simulink model "DFL_IMAP"  (R2018b)
settings: Solver=FixedStepDiscrete  StartTime=0.0  StopTime=10.0  FixedStep=0.01  RelTol=1e-3
(part 1 of 5)
settings Model: Creator=hejr  LastModifiedBy=hejr
settings OptimizationCC: BlockReduction=off  DefaultParameterBehavior=Inlined  DefaultUnderspecifiedDataType=single  EnhancedBackFolding=on  PassReuseOutputArgsAs=Individual arguments  ZeroExternalMemoryAtStartup=off  ZeroInternalMemoryAtStartup=off  OptimizeBlockOrder=speed  DifferentSizesBufferReuse=on  OptimizationCustomize=off
settings DebuggingCC: ParameterTunabilityLossMsg=error
settings SFSimCC: MATLABDynamicMemAlloc=off
settings RTWCC: SystemTargetFile=autosar.tlc  GenCodeOnly=on  TemplateMakefile=ert_default_tmf  Description=AUTOSAR  GenerateReport=on  IncludeHyperlinkInReport=on  LaunchReport=on  GenerateTraceInfo=on  GenerateTraceReport=on  GenerateTraceReportSl=on  GenerateTraceReportSf=on  GenerateTraceReportEml=on  GenerateCodeMetricsReport=on
settings CodeAppCC: ForceParamTrailComments=on  IgnoreCustomStorageClasses=off  OperatorAnnotations=on  SimulinkDataObjDesc=on  SFDataObjDesc=on  InsertBlockDesc=on
settings STFCustomTargetCC: TargetLangStandard=C99 (ISO)  MultiwordLength=256  ParMdlRefBuildCompliant=on  CompOptLevelCompliant=on  IncludeMdlTerminateFcn=off  CombineOutputUpdateFcns=on  SuppressErrorStatus=on  ERTCustomFileBanners=on  SupportNonFinite=off  SupportComplex=off  SupportContinuousTime=off  SupportNonInlinedSFcns=off  RemoveResetFunc=on  MATLABClassNameForMDSCustomization=Simulink.SoftwareTarget.ERTCustomization  AutosarCompliant=on  UseToolchainInfoCompliant=on  LookupTableObjectStructAxisOrder=2,1,3,4,...  LUTObjectStructOrderEvenSpacing=Size,Table,Breakpoints  SystemTargetFile=autosar.tlc
settings ERTTargetCC: TargetLangStandard=C99 (ISO)  ConcurrentExecutionCompliant=off  IncludeMdlTerminateFcn=off  SuppressErrorStatus=on  SupportNonFinite=off  SupportComplex=off  ModelStepFunctionPrototypeControlCompliant=off  CPPClassGenCompliant=off  AutosarCompliant=on  LookupTableObjectStructAxisOrder=2,1,3,4,...  LUTObjectStructOrderEvenSpacing=Size,Table,Breakpoints  GenerateASAP2=on  InlinedParameterPlacement=NonHierarchical  ERTCustomFileTemplate=example_file_process.tlc

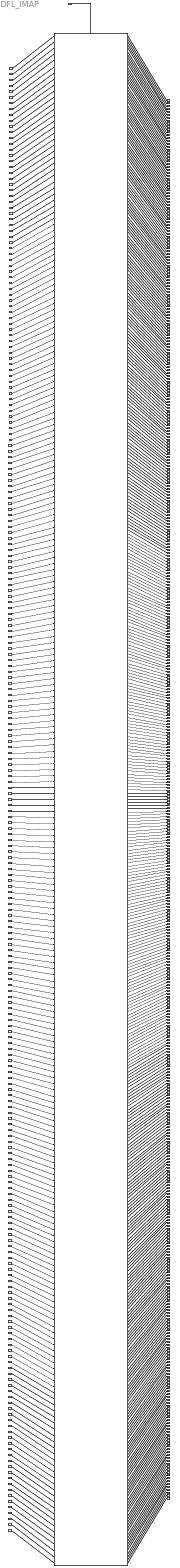
== system DFL_IMAP ==
  SWINve_y_ABS_active : Inport  OutDataTypeStr=UInt8  PortDimensions=1
  SWINve_g_ax : Inport  Port=2  OutDataTypeStr=T_M_Nm_Float32  PortDimensions=1
  SWINve_y_ESP_EnableSts : Inport  Port=3  OutDataTypeStr=UInt8  PortDimensions=1
  SWINve_y_TCS_active : Inport  Port=4  OutDataTypeStr=UInt8  PortDimensions=1
  SWINve_y_Front_Wiper_Status : Inport  Port=5  OutDataTypeStr=UInt8  PortDimensions=1
  SWINve_y_brake_pedal_status : Inport  Port=6  OutDataTypeStr=UInt8  PortDimensions=1
  SWINve_y_Engine1_IND_AccelPadel_Override : Inport  Port=7  OutDataTypeStr=UInt8  PortDimensions=1
  SWINve_y_Engine3_Status_ExtFunctionValid : Inport  Port=8  OutDataTypeStr=UInt8  PortDimensions=1
  SWINve_g_Accelerator_ActPedPos : Inport  Port=9  OutDataTypeStr=T_M_Nm_Float32  PortDimensions=1
  SWINve_g_actual_powertrain_torque : Inport  Port=10  OutDataTypeStr=T_M_Nm_Float32  PortDimensions=1
  SWINve_d_engine_revolution_speed : Inport  Port=11  OutDataTypeStr=UInt16  PortDimensions=1
  SWINve_y_Engine_Status : Inport  Port=12  OutDataTypeStr=UInt8  PortDimensions=1
  SWINve_g_maximum_powertrain_torque : Inport  Port=13  OutDataTypeStr=T_M_Nm_Float32  PortDimensions=1
  SWINve_g_minimum_powertrain_torque : Inport  Port=14  OutDataTypeStr=T_M_Nm_Float32  PortDimensions=1
  SWINve_y_VDC_active : Inport  Port=15  OutDataTypeStr=UInt8  PortDimensions=1
  SWINve_y_ABS3_FLWhlPulseCnt_Valid : Inport  Port=16  OutDataTypeStr=UInt8  PortDimensions=1
  SWINve_y_ABS3_FRWhlPulseCnt_Valid : Inport  Port=17  OutDataTypeStr=UInt8  PortDimensions=1
  SWINve_y_BCM_IgnKeyPOS : Inport  Port=18  OutDataTypeStr=UInt8  PortDimensions=1
  SWINve_y_Engine1_Status_DASReq_Resp : Inport  Port=19  OutDataTypeStr=UInt8  PortDimensions=1
  SWINve_y_Mp5_ISA_Switch : Inport  Port=20  OutDataTypeStr=UInt8  PortDimensions=1
  SWINve_y_Mp5_TSR_Switch : Inport  Port=21  OutDataTypeStr=UInt8  PortDimensions=1
  SWINve_y_BCM1_IND_HighBeamSwt_OnOff : Inport  Port=22  OutDataTypeStr=UInt8  PortDimensions=1
  SWINve_y_MP5_FCWSwitch : Inport  Port=23  OutDataTypeStr=UInt8  PortDimensions=1
  SWINve_y_MP5_FCW_Sensitivity : Inport  Port=24  OutDataTypeStr=UInt8  PortDimensions=1
  SWINve_y_Psngr_Seat_Belt_Sts : Inport  Port=25  OutDataTypeStr=UInt8  PortDimensions=1
  SWINve_y_Driver_Seat_Belt_Sts : Inport  Port=26  OutDataTypeStr=UInt8  PortDimensions=1
  SWINve_y_steering_angle_valid : Inport  Port=27  OutDataTypeStr=UInt8  PortDimensions=1
  SWINve_g_ay : Inport  Port=28  OutDataTypeStr=T_M_Nm_Float32  PortDimensions=1
  SWINve_y_Mp5_LSS_Mode : Inport  Port=29  OutDataTypeStr=UInt8  PortDimensions=1
  SWINve_y_Mp5_LSS_main_SW : Inport  Port=30  OutDataTypeStr=UInt8  PortDimensions=1
  SWINve_y_MP5_AEBSwitch : Inport  Port=31  OutDataTypeStr=UInt8  PortDimensions=1
  SWINve_g_wheel_speed_FL : Inport  Port=32  OutDataTypeStr=T_M_Nm_Float32  PortDimensions=1
  SWINve_g_wheel_speed_FR : Inport  Port=33  OutDataTypeStr=T_M_Nm_Float32  PortDimensions=1
  SWINve_g_wheel_speed_RL : Inport  Port=34  OutDataTypeStr=T_M_Nm_Float32  PortDimensions=1
  SWINve_g_wheel_speed_RR : Inport  Port=35  OutDataTypeStr=T_M_Nm_Float32  PortDimensions=1
  SWINve_g_odometer_value : Inport  Port=36  OutDataTypeStr=UInt32  PortDimensions=1
  SWINve_y_APB_Status : Inport  Port=37  OutDataTypeStr=UInt8  PortDimensions=1
  SWINve_y_ABS3_WhlPulseCnt_FL : Inport  Port=38  OutDataTypeStr=UInt8  PortDimensions=1
  SWINve_y_ABS3_WhlPulseCnt_FR : Inport  Port=39  OutDataTypeStr=UInt8  PortDimensions=1
  SWINve_y_ABS3_WhlPulseCnt_RL : Inport  Port=40  OutDataTypeStr=UInt8  PortDimensions=1
  SWINve_y_ABS3_WhlPulseCnt_RR : Inport  Port=41  OutDataTypeStr=UInt8  PortDimensions=1
  SWINve_y_ABS3_RLWhlPulseCnt_Valid : Inport  Port=42  OutDataTypeStr=UInt8  PortDimensions=1
  SWINve_y_ABS3_RRWhlPulseCnt_Valid : Inport  Port=43  OutDataTypeStr=UInt8  PortDimensions=1
  SWINve_y_VDC_Fault : Inport  Port=44  OutDataTypeStr=UInt8  PortDimensions=1
  SWINve_y_EPS1_Status_Handsoff : Inport  Port=45  OutDataTypeStr=UInt8  PortDimensions=1
  SWINve_y_EPS1_LKA_AvailSts : Inport  Port=46  OutDataTypeStr=UInt8  PortDimensions=1
  SWINve_g_steering_angle : Inport  Port=47  OutDataTypeStr=T_M_Nm_Float32  PortDimensions=1
  SWINve_g_steering_angle_spd : Inport  Port=48  OutDataTypeStr=T_M_Nm_Float32  PortDimensions=1
  SWINve_y_calibrated_status : Inport  Port=49  OutDataTypeStr=UInt8  PortDimensions=1
  SWINve_y_trimming_status : Inport  Port=50  OutDataTypeStr=UInt8  PortDimensions=1
  SWINve_y_TargetGear : Inport  Port=51  OutDataTypeStr=UInt8  PortDimensions=1
  SWINve_y_TCU2_Status_TransFailure : Inport  Port=52  OutDataTypeStr=UInt8  PortDimensions=1
  SWINve_y_ActualGear : Inport  Port=53  OutDataTypeStr=UInt8  PortDimensions=1
  SWINve_y_brake_pressure : Inport  Port=54  OutDataTypeStr=UInt8  PortDimensions=1
  SWINve_y_ESP_Status_Hold : Inport  Port=55  OutDataTypeStr=UInt8  PortDimensions=1
  SWINve_g_vehicle_speed : Inport  Port=56  OutDataTypeStr=T_M_Nm_Float32  PortDimensions=1
  SWINve_g_yrs : Inport  Port=57  OutDataTypeStr=T_M_Nm_Float32  PortDimensions=1
  System_Clock : Inport  Port=58  OutDataTypeStr=UInt16  PortDimensions=1
  SWINve_y_ABS1_RotDir_FL : Inport  Port=59  OutDataTypeStr=UInt8  PortDimensions=1
  SWINve_y_ABS1_RotDir_FR : Inport  Port=60  OutDataTypeStr=UInt8  PortDimensions=1
  SWINve_y_TCS_Fault : Inport  Port=61  OutDataTypeStr=UInt8  PortDimensions=1
  SWINve_y_ABS1_RotDir_RL : Inport  Port=62  OutDataTypeStr=UInt8  PortDimensions=1
  SWINve_y_ABS1_RotDir_RR : Inport  Port=63  OutDataTypeStr=UInt8  PortDimensions=1
  SWINve_y_APB_IND_Error : Inport  Port=64  OutDataTypeStr=UInt8  PortDimensions=1
  SWINve_y_BCM1_Status_ACCSwt : Inport  Port=65  OutDataTypeStr=UInt8  PortDimensions=1
  SWINve_y_Mp5_ISA_Mode : Inport  Port=66  OutDataTypeStr=UInt8  PortDimensions=1
  SWINve_y_Mp5_LDW_Warning_Mode : Inport  Port=67  OutDataTypeStr=UInt8  PortDimensions=1
  SWINve_y_MP5_TLCModeSelection : Inport  Port=68  OutDataTypeStr=UInt8  PortDimensions=1
  SWINve_y_MP5_ESASwitch : Inport  Port=69  OutDataTypeStr=UInt8  PortDimensions=1
  SWINve_y_MP5_BSD_LCW_Activation : Inport  Port=70  OutDataTypeStr=UInt8  PortDimensions=1
  SWINve_y_MP5_FCTAActivation : Inport  Port=71  OutDataTypeStr=UInt8  PortDimensions=1
  SWINve_y_MP5_RCTAActivation : Inport  Port=72  OutDataTypeStr=UInt8  PortDimensions=1
  SWINve_y_MP5_DOWActivation : Inport  Port=73  OutDataTypeStr=UInt8  PortDimensions=1
  SWINve_y_MP5_JASwitch : Inport  Port=74  OutDataTypeStr=UInt8
  Runnable_IMAP_Step : Inport  Port=75  SampleTime=0.01  OutputFunctionCall=on
  SWINve_y_BCM_DrDoorLockSwStatus : Inport  Port=76  OutDataTypeStr=UInt8  PortDimensions=1
  SWINve_y_Low_Beam_Status : Inport  Port=77  OutDataTypeStr=UInt8  PortDimensions=1
  SWINve_g_AC1_Status_AmbientTemp_Lvl : Inport  Port=78  OutDataTypeStr=T_M_Nm_Float32  PortDimensions=1
  SWINve_y_ay_fault : Inport  Port=79  OutDataTypeStr=UInt8  PortDimensions=1
  SWINve_y_yrs_fault : Inport  Port=80  OutDataTypeStr=UInt8  PortDimensions=1
  SWINve_y_ax_fault : Inport  Port=81  OutDataTypeStr=UInt8  PortDimensions=1
  SWINve_y_ABS_fault : Inport  Port=82  OutDataTypeStr=UInt8  PortDimensions=1
  SWINve_y_wheel_speed_FL_fault : Inport  Port=83  OutDataTypeStr=UInt8  PortDimensions=1
  SWINve_y_wheel_speed_FR_fault : Inport  Port=84  OutDataTypeStr=UInt8  PortDimensions=1
  SWINve_y_wheel_speed_RL_fault : Inport  Port=85  OutDataTypeStr=UInt8  PortDimensions=1
  SWINve_y_wheel_speed_RR_fault : Inport  Port=86  OutDataTypeStr=UInt8  PortDimensions=1
  SWINve_y_ESP_Status_AEB_Available : Inport  Port=87  OutDataTypeStr=UInt8  PortDimensions=1
  SWINve_y_ESP_Status_AEBReq_Response : Inport  Port=88  OutDataTypeStr=UInt8  PortDimensions=1
  SWINve_y_ESP_Status_ACC_Available : Inport  Port=89  OutDataTypeStr=UInt8  PortDimensions=1
  SWINve_y_ESP_Status_ACCReq_Response : Inport  Port=90  OutDataTypeStr=UInt8  PortDimensions=1
  SWINve_y_EBD_fault : Inport  Port=91  OutDataTypeStr=UInt8  PortDimensions=1
  SWINve_y_Left_Turn_Lamp_Status : Inport  Port=92  OutDataTypeStr=UInt8  PortDimensions=1
  SWINve_y_Right_Turn_Lamp_Status : Inport  Port=93  OutDataTypeStr=UInt8  PortDimensions=1
  SWINve_y_BCM_LuggageDoorSt : Inport  Port=94  OutDataTypeStr=UInt8  PortDimensions=1
  SWINve_y_BCM_DriverDoorSt : Inport  Port=95  OutDataTypeStr=UInt8  PortDimensions=1
  SWINve_y_BCM_PassDoorSt : Inport  Port=96  OutDataTypeStr=UInt8  PortDimensions=1
  SWINve_y_BCM_RRDoorSt : Inport  Port=97  OutDataTypeStr=UInt8  PortDimensions=1
  SWINve_y_BCM_RLDoorSt : Inport  Port=98  OutDataTypeStr=UInt8  PortDimensions=1
  SWINve_y_High_Beam_Status : Inport  Port=99  OutDataTypeStr=UInt8  PortDimensions=1
  SWINve_y_Front_Fog_Lamp_Status : Inport  Port=100  OutDataTypeStr=UInt8  PortDimensions=1
  SWINve_y_Rear_Fog_Lamp_Status : Inport  Port=101  OutDataTypeStr=UInt8  PortDimensions=1
  SWINve_y_BCM1_Rain_Intensity : Inport  Port=102  OutDataTypeStr=UInt8  PortDimensions=1
  SWINve_y_BCM1_IND_OvertakinglampSwt_OnOff : Inport  Port=103  OutDataTypeStr=UInt8  PortDimensions=1
  SWINve_y_kick_down : Inport  Port=104  OutDataTypeStr=UInt8  PortDimensions=1
  SWINve_g_Mech_Loss_Eng_Torq : Inport  Port=105  OutDataTypeStr=T_M_Nm_Float32  PortDimensions=1
  SWINve_y_Powertrain_Torque_Validity : Inport  Port=106  OutDataTypeStr=UInt8  PortDimensions=1
  SWINve_y_ESP_Status_ACCInfo_Error : Inport  Port=107  OutDataTypeStr=UInt8  PortDimensions=1
  SWINve_y_ESP_Status_Prefill_Response : Inport  Port=108  OutDataTypeStr=UInt8  PortDimensions=1
  SWINve_y_ESP_Status_AEBJerk_Response : Inport  Port=109  OutDataTypeStr=UInt8  PortDimensions=1
  SWINve_y_ESP_Status_FCW_DBS_Response : Inport  Port=110  OutDataTypeStr=UInt8  PortDimensions=1
  SWINve_y_ESP_Status_AEBJerk_Available : Inport  Port=111  OutDataTypeStr=UInt8  PortDimensions=1
  SWINve_y_ESP_Status_FCW_DBS_Available : Inport  Port=112  OutDataTypeStr=UInt8  PortDimensions=1
  SWINve_y_ESP_Status_Prefill_Available : Inport  Port=113  OutDataTypeStr=UInt8  PortDimensions=1
  SWINve_g_EPS1_IND_LKAOverlayTorque_Value : Inport  Port=114  OutDataTypeStr=T_M_Nm_Float32  PortDimensions=1
  SWINve_g_EPS1_IND_DriverTorque_Value : Inport  Port=115  OutDataTypeStr=T_M_Nm_Float32  PortDimensions=1
  SWINve_y_EPS1_Status_HandsoffValid : Inport  Port=116  OutDataTypeStr=UInt8  PortDimensions=1
  CAFDva_y_F_CameraData600 : Inport  Port=117  OutDataTypeStr=UInt8  PortDimensions=66
  CAFDva_y_F_CameraData424 : Inport  Port=118  OutDataTypeStr=UInt8  PortDimensions=66
  CAFDva_y_F_CameraData425 : Inport  Port=119  OutDataTypeStr=UInt8  PortDimensions=66
  CAFDva_y_F_CameraData450 : Inport  Port=120  OutDataTypeStr=UInt8  PortDimensions=66
  CAFDva_y_F_CameraData459 : Inport  Port=121  OutDataTypeStr=UInt8  PortDimensions=66
  CAFDva_y_F_CameraData45A : Inport  Port=122  OutDataTypeStr=UInt8  PortDimensions=66
  CAFDva_y_F_CameraData45B : Inport  Port=123  OutDataTypeStr=UInt8  PortDimensions=66
  CAFDva_y_F_CameraData45C : Inport  Port=124  OutDataTypeStr=UInt8  PortDimensions=66
  CAFDva_y_F_CameraData45D : Inport  Port=125  OutDataTypeStr=UInt8  PortDimensions=66
  CAFDva_y_F_CameraData45E : Inport  Port=126  OutDataTypeStr=UInt8  PortDimensions=66
  CAFDva_y_F_CameraData45F : Inport  Port=127  OutDataTypeStr=UInt8  PortDimensions=66
  CAFDva_y_F_CameraData420 : Inport  Port=128  OutDataTypeStr=UInt8  PortDimensions=66
  CAFDva_y_F_CameraData421 : Inport  Port=129  OutDataTypeStr=UInt8  PortDimensions=66
  CAFDva_y_F_CameraData422 : Inport  Port=130  OutDataTypeStr=UInt8  PortDimensions=66
  CAFDva_y_F_CameraData451 : Inport  Port=131  OutDataTypeStr=UInt8  PortDimensions=66
  CAFDva_y_F_CameraData423 : Inport  Port=132  OutDataTypeStr=UInt8  PortDimensions=66
  CAFDva_y_F_CameraData452 : Inport  Port=133  OutDataTypeStr=UInt8  PortDimensions=66
  CAFDva_y_F_CameraData453 : Inport  Port=134  OutDataTypeStr=UInt8  PortDimensions=66
  CAFDva_y_F_CameraData454 : Inport  Port=135  OutDataTypeStr=UInt8  PortDimensions=66
  CAFDva_y_F_CameraData455 : Inport  Port=136  OutDataTypeStr=UInt8  PortDimensions=66
  CAFDva_y_F_CameraData456 : Inport  Port=137  OutDataTypeStr=UInt8  PortDimensions=66
  CAFDva_y_F_CameraData457 : Inport  Port=138  OutDataTypeStr=UInt8  PortDimensions=66
  CAFDva_y_F_CameraData458 : Inport  Port=139  OutDataTypeStr=UInt8  PortDimensions=66
  CAFDva_y_F_CameraData426 : Inport  Port=140  OutDataTypeStr=UInt8  PortDimensions=66
  CAFDva_y_F_CameraData47E : Inport  Port=141  OutDataTypeStr=uint8  PortDimensions=66
  SDFAve_d_sensor_status : Inport  Port=142  OutDataTypeStr=UInt16  PortDimensions=1
  SDFAve_d_sen_sta_LF_radar : Inport  Port=143  OutDataTypeStr=UInt16  PortDimensions=1
  SDFAve_d_sen_sta_RF_radar : Inport  Port=144  OutDataTypeStr=UInt16  PortDimensions=1
  SDFAve_d_sen_sta_LB_radar : Inport  Port=145  OutDataTypeStr=UInt16  PortDimensions=1
  SDFAve_d_sen_sta_RB_radar : Inport  Port=146  OutDataTypeStr=UInt16  PortDimensions=1
  SDFAve_d_fusion_status : Inport  Port=147  OutDataTypeStr=UInt16  PortDimensions=1
  SDFAve_g_fusion_time_stamp : Inport  Port=148  OutDataTypeStr=T_M_Nm_Float32  PortDimensions=1
  SDFAve_d_obj_Num : Inport  Port=149  OutDataTypeStr=UInt16  PortDimensions=1
  SDFAva_y_obj_id : Inport  Port=150  OutDataTypeStr=UInt8  PortDimensions=40
  SDFAva_g_obj_pos_x : Inport  Port=151  OutDataTypeStr=T_M_Nm_Float32  PortDimensions=40
  SDFAva_g_obj_pos_y : Inport  Port=152  OutDataTypeStr=T_M_Nm_Float32  PortDimensions=40
  SDFAva_g_obj_vel_x : Inport  Port=153  OutDataTypeStr=T_M_Nm_Float32  PortDimensions=40
  SDFAva_g_obj_vel_y : Inport  Port=154  OutDataTypeStr=T_M_Nm_Float32  PortDimensions=40
  SDFAva_g_obj_acc_x : Inport  Port=155  OutDataTypeStr=T_M_Nm_Float32  PortDimensions=40
  SDFAva_g_obj_acc_y : Inport  Port=156  OutDataTypeStr=T_M_Nm_Float32  PortDimensions=40
  SDFAva_g_obj_pos_var_x : Inport  Port=157  OutDataTypeStr=T_M_Nm_Float32  PortDimensions=40
  SDFAva_g_obj_pos_var_y : Inport  Port=158  OutDataTypeStr=T_M_Nm_Float32  PortDimensions=40
  SDFAva_g_obj_pos_var_xy : Inport  Port=159  OutDataTypeStr=T_M_Nm_Float32  PortDimensions=40
  SDFAva_g_obj_width : Inport  Port=160  OutDataTypeStr=T_M_Nm_Float32  PortDimensions=40
  SDFAva_g_obj_length : Inport  Port=161  OutDataTypeStr=T_M_Nm_Float32  PortDimensions=40
  SDFAva_y_obj_class : Inport  Port=162  OutDataTypeStr=UInt8  PortDimensions=40
  SDFAva_y_obj_lane : Inport  Port=163  OutDataTypeStr=UInt8  PortDimensions=40
  SDFAva_y_obj_status : Inport  Port=164  OutDataTypeStr=UInt8  PortDimensions=40
  SDFAva_d_obj_age : Inport  Port=165  OutDataTypeStr=UInt16  PortDimensions=40
  SDFAva_y_obj_TurnLight : Inport  Port=166  OutDataTypeStr=UInt8  PortDimensions=40
  SDFAva_y_obj_BrakeLight : Inport  Port=167  OutDataTypeStr=UInt8  PortDimensions=40
  SDFAva_y_obj_MotionStatus : Inport  Port=168  OutDataTypeStr=UInt8  PortDimensions=40
  SDFAve_y_LANE_DETECT_ACTIV : Inport  Port=169  OutDataTypeStr=UInt8  PortDimensions=1
  SDFAve_y_ROAD_TYPE : Inport  Port=170  OutDataTypeStr=UInt8  PortDimensions=1
  SDFAve_y_CONSTRUCTION_AREA : Inport  Port=171  OutDataTypeStr=UInt8  PortDimensions=1
  SDFAve_g_L0_C0_COEF : Inport  Port=172  OutDataTypeStr=T_M_Nm_Float32  PortDimensions=1
  SDFAve_g_L0_C1_COEF : Inport  Port=173  OutDataTypeStr=T_M_Nm_Float32  PortDimensions=1
  SDFAve_g_L0_C2_COEF : Inport  Port=174  OutDataTypeStr=T_M_Nm_Float32  PortDimensions=1
  SDFAve_g_L0_C3_COEF : Inport  Port=175  OutDataTypeStr=T_M_Nm_Float32  PortDimensions=1
  SDFAve_g_L0_VIEW_RANGE : Inport  Port=176  OutDataTypeStr=T_M_Nm_Float32  PortDimensions=1
  SDFAve_y_L0_DETECT_QUALITY : Inport  Port=177  OutDataTypeStr=UInt8  PortDimensions=1
  SDFAve_d_L0_LINE_TYPE : Inport  Port=178  OutDataTypeStr=UInt16  PortDimensions=1
  SDFAve_g_L0_LINE_COFIDENCE : Inport  Port=179  OutDataTypeStr=T_M_Nm_Float32  PortDimensions=1
  SDFAve_g_L0_MARK_WIDTH : Inport  Port=180  OutDataTypeStr=T_M_Nm_Float32  PortDimensions=1
  SDFAve_g_L0_TLC : Inport  Port=181  OutDataTypeStr=T_M_Nm_Float32  PortDimensions=1
  SDFAve_y_L0_LANE_CHANGE : Inport  Port=182  OutDataTypeStr=UInt8  PortDimensions=1
  SDFAve_g_R0_C0_COEF : Inport  Port=183  OutDataTypeStr=T_M_Nm_Float32  PortDimensions=1
  SDFAve_g_R0_C1_COEF : Inport  Port=184  OutDataTypeStr=T_M_Nm_Float32  PortDimensions=1
  SDFAve_g_R0_C2_COEF : Inport  Port=185  OutDataTypeStr=T_M_Nm_Float32  PortDimensions=1
  SDFAve_g_R0_C3_COEF : Inport  Port=186  OutDataTypeStr=T_M_Nm_Float32  PortDimensions=1
  SDFAve_g_R0_VIEW_RANGE : Inport  Port=187  OutDataTypeStr=T_M_Nm_Float32  PortDimensions=1
  SDFAve_y_R0_DETECT_QUALITY : Inport  Port=188  OutDataTypeStr=UInt8  PortDimensions=1
  SDFAve_d_R0_LINE_TYPE : Inport  Port=189  OutDataTypeStr=UInt16  PortDimensions=1
  SDFAve_g_R0_LINE_COFIDENCE : Inport  Port=190  OutDataTypeStr=T_M_Nm_Float32  PortDimensions=1
  SDFAve_g_R0_MARK_WIDTH : Inport  Port=191  OutDataTypeStr=T_M_Nm_Float32  PortDimensions=1
  SDFAve_g_R0_TLC : Inport  Port=192  OutDataTypeStr=T_M_Nm_Float32  PortDimensions=1
  SDFAve_y_R0_LANE_CHANGE : Inport  Port=193  OutDataTypeStr=UInt8  PortDimensions=1
  SDFAve_g_L1_C0_COEF : Inport  Port=194  OutDataTypeStr=T_M_Nm_Float32  PortDimensions=1
  SDFAve_g_L1_C1_COEF : Inport  Port=195  OutDataTypeStr=T_M_Nm_Float32  PortDimensions=1
  SDFAve_g_L1_C2_COEF : Inport  Port=196  OutDataTypeStr=T_M_Nm_Float32  PortDimensions=1
  SDFAve_g_L1_C3_COEF : Inport  Port=197  OutDataTypeStr=T_M_Nm_Float32  PortDimensions=1
  SDFAve_g_L1_VIEW_RANGE : Inport  Port=198  OutDataTypeStr=T_M_Nm_Float32  PortDimensions=1
  SDFAve_y_L1_DETECT_QUALITY : Inport  Port=199  OutDataTypeStr=UInt8  PortDimensions=1
  SDFAve_d_L1_LINE_TYPE : Inport  Port=200  OutDataTypeStr=UInt16  PortDimensions=1
  SDFAve_g_L1_LINE_COFIDENCE : Inport  Port=201  OutDataTypeStr=T_M_Nm_Float32  PortDimensions=1
  SDFAve_g_L1_MARK_WIDTH : Inport  Port=202  OutDataTypeStr=T_M_Nm_Float32  PortDimensions=1
  SDFAve_g_L1_TLC : Inport  Port=203  OutDataTypeStr=T_M_Nm_Float32  PortDimensions=1
  SDFAve_y_L1_LANE_CHANGE : Inport  Port=204  OutDataTypeStr=UInt8  PortDimensions=1
  SDFAve_g_R1_C0_COEF : Inport  Port=205  OutDataTypeStr=T_M_Nm_Float32  PortDimensions=1
  SDFAve_g_R1_C1_COEF : Inport  Port=206  OutDataTypeStr=T_M_Nm_Float32  PortDimensions=1
  SDFAve_g_R1_C2_COEF : Inport  Port=207  OutDataTypeStr=T_M_Nm_Float32  PortDimensions=1
  SDFAve_g_R1_C3_COEF : Inport  Port=208  OutDataTypeStr=T_M_Nm_Float32  PortDimensions=1
  SDFAve_g_R1_VIEW_RANGE : Inport  Port=209  OutDataTypeStr=T_M_Nm_Float32  PortDimensions=1
  SDFAve_y_R1_DETECT_QUALITY : Inport  Port=210  OutDataTypeStr=UInt8  PortDimensions=1
  SDFAve_d_R1_LINE_TYPE : Inport  Port=211  OutDataTypeStr=UInt16  PortDimensions=1
  SDFAve_g_R1_LINE_COFIDENCE : Inport  Port=212  OutDataTypeStr=T_M_Nm_Float32  PortDimensions=1
  SDFAve_g_R1_MARK_WIDTH : Inport  Port=213  OutDataTypeStr=T_M_Nm_Float32  PortDimensions=1
  SDFAve_g_R1_TLC : Inport  Port=214  OutDataTypeStr=T_M_Nm_Float32  PortDimensions=1
  SDFAve_y_R1_LANE_CHANGE : Inport  Port=215  OutDataTypeStr=UInt8  PortDimensions=1
  SDFAve_g_L0_C0_BACK_COEF : Inport  Port=216  OutDataTypeStr=T_M_Nm_Float32  PortDimensions=1
  SDFAve_g_L0_C1_BACK_COEF : Inport  Port=217  OutDataTypeStr=T_M_Nm_Float32  PortDimensions=1
  SDFAve_g_L0_C2_BACK_COEF : Inport  Port=218  OutDataTypeStr=T_M_Nm_Float32  PortDimensions=1
  SDFAve_g_L0_C3_BACK_COEF : Inport  Port=219  OutDataTypeStr=T_M_Nm_Float32  PortDimensions=1
  SDFAve_g_L0_BACK_RANGE : Inport  Port=220  OutDataTypeStr=T_M_Nm_Float32  PortDimensions=1
  SDFAve_g_L0_C0_FR_PRE_COEF : Inport  Port=221  OutDataTypeStr=T_M_Nm_Float32  PortDimensions=1
  SDFAve_g_L0_C1_FR_PRE_COEF : Inport  Port=222  OutDataTypeStr=T_M_Nm_Float32  PortDimensions=1
  SDFAve_g_L0_C2_FR_PRE_COEF : Inport  Port=223  OutDataTypeStr=T_M_Nm_Float32  PortDimensions=1
  SDFAve_g_L0_FR_PRED_RANGE : Inport  Port=224  OutDataTypeStr=T_M_Nm_Float32  PortDimensions=1
  SDFAve_g_R0_C0_BACK_COEF : Inport  Port=225  OutDataTypeStr=T_M_Nm_Float32  PortDimensions=1
  SDFAve_g_R0_C1_BACK_COEF : Inport  Port=226  OutDataTypeStr=T_M_Nm_Float32  PortDimensions=1
  SDFAve_g_R0_C2_BACK_COEF : Inport  Port=227  OutDataTypeStr=T_M_Nm_Float32  PortDimensions=1
  SDFAve_g_R0_C3_BACK_COEF : Inport  Port=228  OutDataTypeStr=T_M_Nm_Float32  PortDimensions=1
  SDFAve_g_R0_BACK_RANGE : Inport  Port=229  OutDataTypeStr=T_M_Nm_Float32  PortDimensions=1
  SDFAve_g_R0_C0_FR_PRE_COEF : Inport  Port=230  OutDataTypeStr=T_M_Nm_Float32  PortDimensions=1
  SDFAve_g_R0_C1_FR_PRE_COEF : Inport  Port=231  OutDataTypeStr=T_M_Nm_Float32  PortDimensions=1
  SDFAve_g_R0_C2_FR_PRE_COEF : Inport  Port=232  OutDataTypeStr=T_M_Nm_Float32  PortDimensions=1
  SDFAve_g_R0_FR_PRED_RANGE : Inport  Port=233  OutDataTypeStr=T_M_Nm_Float32  PortDimensions=1
  SDFAve_g_L1_C0_BACK_COEF : Inport  Port=234  OutDataTypeStr=T_M_Nm_Float32  PortDimensions=1
  SDFAve_g_L1_C1_BACK_COEF : Inport  Port=235  OutDataTypeStr=T_M_Nm_Float32  PortDimensions=1
  SDFAve_g_L1_C2_BACK_COEF : Inport  Port=236  OutDataTypeStr=T_M_Nm_Float32  PortDimensions=1
  SDFAve_g_L1_C3_BACK_COEF : Inport  Port=237  OutDataTypeStr=T_M_Nm_Float32  PortDimensions=1
  SDFAve_g_L1_BACK_RANGE : Inport  Port=238  OutDataTypeStr=T_M_Nm_Float32  PortDimensions=1
  SDFAve_g_L1_C0_FR_PRE_COEF : Inport  Port=239  OutDataTypeStr=T_M_Nm_Float32  PortDimensions=1
  SDFAve_g_L1_C1_FR_PRE_COEF : Inport  Port=240  OutDataTypeStr=T_M_Nm_Float32  PortDimensions=1
  SDFAve_g_L1_C2_FR_PRE_COEF : Inport  Port=241  OutDataTypeStr=T_M_Nm_Float32  PortDimensions=1
  SDFAve_g_L1_FR_PRED_RANGE : Inport  Port=242  OutDataTypeStr=T_M_Nm_Float32  PortDimensions=1
  SDFAve_g_R1_C0_BACK_COEF : Inport  Port=243  OutDataTypeStr=T_M_Nm_Float32  PortDimensions=1
  SDFAve_g_R1_C1_BACK_COEF : Inport  Port=244  OutDataTypeStr=T_M_Nm_Float32  PortDimensions=1
  SDFAve_g_R1_C2_BACK_COEF : Inport  Port=245  OutDataTypeStr=T_M_Nm_Float32  PortDimensions=1
  SDFAve_g_R1_C3_BACK_COEF : Inport  Port=246  OutDataTypeStr=T_M_Nm_Float32  PortDimensions=1
  SDFAve_g_R1_BACK_RANGE : Inport  Port=247  OutDataTypeStr=T_M_Nm_Float32  PortDimensions=1
  SDFAve_g_R1_C0_FR_PRE_COEF : Inport  Port=248  OutDataTypeStr=T_M_Nm_Float32  PortDimensions=1
  SDFAve_g_R1_C1_FR_PRE_COEF : Inport  Port=249  OutDataTypeStr=T_M_Nm_Float32  PortDimensions=1
  SDFAve_g_R1_C2_FR_PRE_COEF : Inport  Port=250  OutDataTypeStr=T_M_Nm_Float32  PortDimensions=1
  SDFAve_g_R1_FR_PRED_RANGE : Inport  Port=251  OutDataTypeStr=T_M_Nm_Float32  PortDimensions=1
  SDFAve_y_SIGN_ISA_Value : Inport  Port=252  OutDataTypeStr=UInt8  PortDimensions=1
  SDFAve_y_TSR_Sign_Type : Inport  Port=253  OutDataTypeStr=UInt8  PortDimensions=1
  SDFAve_y_CameraSignalFault : Inport  Port=254  OutDataTypeStr=UInt8  PortDimensions=1
  Runnable_IMAP_10ms_sys : Subsystem  TreatAsAtomicUnit=on
  IMAPve_d_LKA_Main_Switch : Outport  OutDataTypeStr=UInt16  PortDimensions=1
  IMAPve_d_LKA_Mode : Outport  Port=2  OutDataTypeStr=UInt16  PortDimensions=1
  IMAPve_d_AEB_Switch : Outport  Port=3  OutDataTypeStr=UInt16  PortDimensions=1
  IMAPve_d_FCW_Switch : Outport  Port=4  OutDataTypeStr=UInt16  PortDimensions=1
  IMAPve_d_FCW_Sensitivity : Outport  Port=5  OutDataTypeStr=UInt16  PortDimensions=1
  IMAPve_d_ISA_Switch : Outport  Port=6  OutDataTypeStr=UInt16  PortDimensions=1  LockScale=on
  IMAPve_d_TSR_Switch : Outport  Port=7  OutDataTypeStr=UInt16  PortDimensions=1
  IMAPve_d_ISA_ISLC_Mode : Outport  Port=8  OutDataTypeStr=UInt16  PortDimensions=1
  IMAPve_d_LDW_Warn_Mode : Outport  Port=9  OutDataTypeStr=UInt16  PortDimensions=1
  IMAPve_d_Speed_Limit : Outport  Port=10  OutDataTypeStr=UInt16  PortDimensions=1
  IMAPve_d_ALC_TLC_Mode : Outport  Port=11  OutDataTypeStr=UInt16  PortDimensions=1
  IMAPve_d_ESA_Switch : Outport  Port=12  OutDataTypeStr=UInt16  PortDimensions=1
  IMAPve_d_ELK_Switch : Outport  Port=13  OutDataTypeStr=UInt16  PortDimensions=1
  IMAPve_d_APA_Command : Outport  Port=14  OutDataTypeStr=UInt16  PortDimensions=1
  IMAPve_d_PEPS_RKE_Command : Outport  Port=15  OutDataTypeStr=UInt16  PortDimensions=1
  IMAPve_d_BSD_LCW_Switch : Outport  Port=16  OutDataTypeStr=UInt16  PortDimensions=1
  IMAPve_d_FCTA_Switch : Outport  Port=17  OutDataTypeStr=UInt16  PortDimensions=1
  IMAPve_d_RCTA_Swtich : Outport  Port=18  OutDataTypeStr=UInt16  PortDimensions=1
  IMAPve_d_DOW_Switch : Outport  Port=19  OutDataTypeStr=UInt16  PortDimensions=1
  IMAPve_d_JA_Brake_Switch : Outport  Port=20  OutDataTypeStr=UInt16  PortDimensions=1
  IMAPve_d_JA_Alert_Switch : Outport  Port=21  OutDataTypeStr=UInt16  PortDimensions=1
  IMAPve_d_JA_Alert_Sensitivity : Outport  Port=22  OutDataTypeStr=UInt16  PortDimensions=1
  IMAPve_d_LF_Switch : Outport  Port=23  OutDataTypeStr=UInt16  PortDimensions=1
  IMAPve_d_ICA_Config : Outport  Port=24  OutDataTypeStr=UInt16  PortDimensions=1
  IMAPve_d_ALC_Sensitivity : Outport  Port=25  OutDataTypeStr=UInt16  PortDimensions=1
  IMAPve_d_EPS_LKA_State : Outport  Port=26  OutDataTypeStr=UInt16  PortDimensions=1
  IMAPve_g_EPS_SW_Trq : Outport  Port=27  OutDataTypeStr=T_M_Nm_Float32  PortDimensions=1
  IMAPve_d_EPS_Error_State : Outport  Port=28  OutDataTypeStr=UInt16  PortDimensions=1
  IMAPve_d_EPS_Trq_State : Outport  Port=29  OutDataTypeStr=UInt16  PortDimensions=1
  IMAPve_d_SAS_Clb_State : Outport  Port=30  OutDataTypeStr=UInt16  PortDimensions=1
  IMAPve_d_SAS_Trim_State : Outport  Port=31  OutDataTypeStr=UInt16  PortDimensions=1
  IMAPve_d_EPS_TrqLim_State : Outport  Port=32  OutDataTypeStr=UInt16  PortDimensions=1
  IMAPve_g_EPS_LKA_Current : Outport  Port=33  OutDataTypeStr=T_M_Nm_Float32  PortDimensions=1
  IMAPve_g_ESC_LatAcc : Outport  Port=34  OutDataTypeStr=T_M_Nm_Float32  PortDimensions=1
  IMAPve_d_ESC_LatAcc_Valid : Outport  Port=35  OutDataTypeStr=UInt16  PortDimensions=1
  IMAPve_g_ESC_YawRate : Outport  Port=36  OutDataTypeStr=T_M_Nm_Float32  PortDimensions=1
  IMAPve_d_ESC_YawRate_Valid : Outport  Port=37  OutDataTypeStr=UInt16  PortDimensions=1
  IMAPve_g_ESC_UnYawRate : Outport  Port=38  OutDataTypeStr=T_M_Nm_Float32  PortDimensions=1
  IMAPve_g_ESC_VehSpd : Outport  Port=39  OutDataTypeStr=T_M_Nm_Float32  PortDimensions=1
  IMAPve_g_ESC_LonAcc : Outport  Port=40  OutDataTypeStr=T_M_Nm_Float32  PortDimensions=1
  IMAPve_d_ESC_LonAcc_Valid : Outport  Port=41  OutDataTypeStr=UInt16  PortDimensions=1
  IMAPve_g_ESC_Brake_Press : Outport  Port=42  OutDataTypeStr=T_M_Nm_Float32  PortDimensions=1
  IMAPve_g_ESC_Static_Slope : Outport  Port=43  OutDataTypeStr=T_M_Nm_Float32  PortDimensions=1
  IMAPve_g_ESC_DySlope_Accuracy : Outport  Port=44  OutDataTypeStr=T_M_Nm_Float32  PortDimensions=1
  IMAPve_g_ESC_DySlope : Outport  Port=45  OutDataTypeStr=T_M_Nm_Float32  PortDimensions=1
  IMAPve_g_SW_Angle : Outport  Port=46  OutDataTypeStr=T_M_Nm_Float32  PortDimensions=1
  IMAPve_g_SW_Angle_Speed : Outport  Port=47  OutDataTypeStr=T_M_Nm_Float32  PortDimensions=1
  IMAPve_d_BCM_HazardLamp : Outport  Port=48  OutDataTypeStr=UInt16  PortDimensions=1
  IMAPve_d_BCM_Left_Light : Outport  Port=49  OutDataTypeStr=UInt16  PortDimensions=1
  IMAPve_d_BCM_Right_Light : Outport  Port=50  OutDataTypeStr=UInt16  PortDimensions=1
  IMAPve_d_ESC_BrakeLamp_Req : Outport  Port=51  OutDataTypeStr=UInt16  PortDimensions=1
  IMAPve_d_BCM_Opening_State : Outport  Port=52  OutDataTypeStr=UInt16  PortDimensions=1
  IMAPve_d_BCM_Trunk_State : Outport  Port=53  OutDataTypeStr=UInt16  PortDimensions=1
  IMAPve_d_BCM_LF_Door_State : Outport  Port=54  OutDataTypeStr=UInt16  PortDimensions=1
  IMAPve_d_BCM_RF_Door_State : Outport  Port=55  OutDataTypeStr=UInt16  PortDimensions=1
  IMAPve_d_BCM_RR_Door_State : Outport  Port=56  OutDataTypeStr=UInt16  PortDimensions=1
  IMAPve_d_BCM_LR_Door_State : Outport  Port=57  OutDataTypeStr=UInt16  PortDimensions=1
  IMAPve_d_SCC_Left_SwitchSig : Outport  Port=58  OutDataTypeStr=UInt16  PortDimensions=1
  IMAPve_d_SCC_Right_SwitchSig : Outport  Port=59  OutDataTypeStr=UInt16  PortDimensions=1
  IMAPve_d_PEPS_Door_Lock_Req : Outport  Port=60  OutDataTypeStr=UInt16  PortDimensions=1
  IMAPve_d_BCM_Door_Lock_State : Outport  Port=61  OutDataTypeStr=UInt16  PortDimensions=1
  IMAPve_d_EMS_ACC_Status : Outport  Port=62  OutDataTypeStr=UInt16  PortDimensions=1
  IMAPve_g_EMS_Pot_WhlT_Max : Outport  Port=63  OutDataTypeStr=T_M_Nm_Float32  PortDimensions=1
  IMAPve_g_EMS_Pot_WhlT_Min : Outport  Port=64  OutDataTypeStr=T_M_Nm_Float32  PortDimensions=1
  IMAPve_g_EMS_RealPedal : Outport  Port=65  OutDataTypeStr=T_M_Nm_Float32  PortDimensions=1
  IMAPve_g_EMS_MaxTWhl : Outport  Port=66  OutDataTypeStr=T_M_Nm_Float32  PortDimensions=1
  IMAPve_g_EMS_MaxTWhl_Offset : Outport  Port=67  OutDataTypeStr=T_M_Nm_Float32  PortDimensions=1
  IMAPve_g_EMS_MinTWhl : Outport  Port=68  OutDataTypeStr=T_M_Nm_Float32  PortDimensions=1
  IMAPve_g_EMS_MinTWhl_Offset : Outport  Port=69  OutDataTypeStr=T_M_Nm_Float32  PortDimensions=1
  IMAPve_g_EMS_Actual_FlwT : Outport  Port=70  OutDataTypeStr=T_M_Nm_Float32  PortDimensions=1
  IMAPve_g_EMS_Actual_IndT : Outport  Port=71  OutDataTypeStr=T_M_Nm_Float32  PortDimensions=1
  IMAPve_g_EMS_Realize_TWhl : Outport  Port=72  OutDataTypeStr=T_M_Nm_Float32  PortDimensions=1
  IMAPve_g_EMS_ACC_VirtualPedal : Outport  Port=73  OutDataTypeStr=T_M_Nm_Float32  PortDimensions=1
  IMAPve_d_EMS_AccPedal_Fault : Outport  Port=74  OutDataTypeStr=UInt16  PortDimensions=1
  IMAPve_g_EMS_Driver_Torque : Outport  Port=75  OutDataTypeStr=T_M_Nm_Float32  PortDimensions=1
  IMAPve_d_ESC_Brake_Effort : Outport  Port=76  OutDataTypeStr=UInt16  PortDimensions=1
  IMAPve_g_EMS_Engine_Speed : Outport  Port=77  OutDataTypeStr=T_M_Nm_Float32  PortDimensions=1
  IMAPve_d_ESC_Veh_Standstill : Outport  Port=78  OutDataTypeStr=UInt16  PortDimensions=1
  IMAPve_d_TCU_Actual_Gear : Outport  Port=79  OutDataTypeStr=UInt16  PortDimensions=1
  IMAPve_d_TCU_Target_Gear : Outport  Port=80  OutDataTypeStr=UInt16  PortDimensions=1
  IMAPve_d_TCU_PRND_State : Outport  Port=81  OutDataTypeStr=UInt16  PortDimensions=1
  IMAPve_d_BCM_Ignition_State : Outport  Port=82  OutDataTypeStr=UInt16  PortDimensions=1
  IMAPve_d_ACU_Driver_Belt : Outport  Port=83  OutDataTypeStr=UInt16  PortDimensions=1
  IMAPve_d_SWS_Fault_Code : Outport  Port=84  OutDataTypeStr=UInt16  PortDimensions=1
  IMAPve_d_SWS_Failure_Status : Outport  Port=85  OutDataTypeStr=UInt16  PortDimensions=1
  IMAPve_d_ESC_OFF : Outport  Port=86  OutDataTypeStr=UInt16  PortDimensions=1
  IMAPve_d_ESC_AlarmSig : Outport  Port=87  OutDataTypeStr=UInt16  PortDimensions=1
  IMAPve_d_Speed_Limit_Switch : Outport  Port=88  OutDataTypeStr=UInt16  PortDimensions=1
  IMAPve_d_ESC_ESC_Active : Outport  Port=89  OutDataTypeStr=UInt16  PortDimensions=1
  IMAPve_d_ESC_MSR_Active : Outport  Port=90  OutDataTypeStr=UInt16  PortDimensions=1
  IMAPve_d_ESC_TCS_Active : Outport  Port=91  OutDataTypeStr=UInt16  PortDimensions=1
  IMAPve_d_ESC_VehSpd_Valid : Outport  Port=92  OutDataTypeStr=UInt16  PortDimensions=1
  IMAPve_d_Brake_Pedal_Fault : Outport  Port=93  OutDataTypeStr=UInt16  PortDimensions=1
  IMAPve_d_ESC_ABS_Active : Outport  Port=94  OutDataTypeStr=UInt16  PortDimensions=1
  IMAPve_d_ESC_ABS_Valid : Outport  Port=95  OutDataTypeStr=UInt16  PortDimensions=1
  IMAPve_d_ESC_ABS_AlarmSig : Outport  Port=96  OutDataTypeStr=UInt16  PortDimensions=1
  IMAPve_d_ESC_FL_WheelPulVal : Outport  Port=97  OutDataTypeStr=UInt16  PortDimensions=1
  IMAPve_d_ESC_FR_WheelPulVal : Outport  Port=98  OutDataTypeStr=UInt16  PortDimensions=1
  IMAPve_d_ESC_RL_WheelPulVal : Outport  Port=99  OutDataTypeStr=UInt16  PortDimensions=1
  IMAPve_d_ESC_RR_WheelPulVal : Outport  Port=100  OutDataTypeStr=UInt16  PortDimensions=1
  IMAPve_g_ESC_FL_WhlSpd : Outport  Port=101  OutDataTypeStr=T_M_Nm_Float32  PortDimensions=1
  IMAPve_d_ESC_FL_WhlSpd_Fault : Outport  Port=102  OutDataTypeStr=UInt16  PortDimensions=1
  IMAPve_g_ESC_FR_WhlSpd : Outport  Port=103  OutDataTypeStr=T_M_Nm_Float32  PortDimensions=1
  IMAPve_d_ESC_FR_WhlSpd_Fault : Outport  Port=104  OutDataTypeStr=UInt16  PortDimensions=1
  IMAPve_g_ESC_RL_WhlSpd : Outport  Port=105  OutDataTypeStr=T_M_Nm_Float32  PortDimensions=1
  IMAPve_d_ESC_RL_WhlSpd_Fault : Outport  Port=106  OutDataTypeStr=UInt16  PortDimensions=1
  IMAPve_g_ESC_RR_WhlSpd : Outport  Port=107  OutDataTypeStr=T_M_Nm_Float32  PortDimensions=1
  IMAPve_d_ESC_RR_WhlSpd_Fault : Outport  Port=108  OutDataTypeStr=UInt16  PortDimensions=1
  IMAPve_d_ESC_FL_Wheel_Pulse : Outport  Port=109  OutDataTypeStr=UInt16  PortDimensions=1
  IMAPve_d_ESC_FR_Wheel_Pulse : Outport  Port=110  OutDataTypeStr=UInt16  PortDimensions=1
  IMAPve_d_ESC_RL_Wheel_Pulse : Outport  Port=111  OutDataTypeStr=UInt16  PortDimensions=1
  IMAPve_d_ESC_RR_Wheel_Pulse : Outport  Port=112  OutDataTypeStr=UInt16  PortDimensions=1
  IMAPve_d_TCU_AT_Failure : Outport  Port=113  OutDataTypeStr=UInt16  PortDimensions=1
  IMAPve_d_TCU_Shift_Valid : Outport  Port=114  OutDataTypeStr=UInt16  PortDimensions=1
  IMAPve_d_TCU_DCT_Clutch_State : Outport  Port=115  OutDataTypeStr=UInt16  PortDimensions=1
  IMAPve_d_TCU_Gear_Engage : Outport  Port=116  OutDataTypeStr=UInt16  PortDimensions=1
  IMAPve_d_TCU_Select_ATMode : Outport  Port=117  OutDataTypeStr=UInt16  PortDimensions=1
  IMAPve_d_EMS_Engine_Status : Outport  Port=118  OutDataTypeStr=UInt16  PortDimensions=1
  IMAPve_d_EMS_Gearbox_CtlAvail : Outport  Port=119  OutDataTypeStr=UInt16  PortDimensions=1
  IMAPve_d_ESC_Brake_Failsafe : Outport  Port=120  OutDataTypeStr=UInt16  PortDimensions=1
  IMAPve_d_ESC_AEB_Status : Outport  Port=121  OutDataTypeStr=UInt16  PortDimensions=1
  IMAPve_d_ESC_AEB_Available : Outport  Port=122  OutDataTypeStr=UInt16  PortDimensions=1
  IMAPve_d_ESC_AEB_Active : Outport  Port=123  OutDataTypeStr=UInt16  PortDimensions=1
  IMAPve_d_ESC_ACC_Status : Outport  Port=124  OutDataTypeStr=UInt16  PortDimensions=1
  IMAPve_d_ESC_ACC_Available : Outport  Port=125  OutDataTypeStr=UInt16  PortDimensions=1
  IMAPve_d_ESC_ACC_Active : Outport  Port=126  OutDataTypeStr=UInt16  PortDimensions=1
  IMAPve_d_EMS_ACC_Effective : Outport  Port=127  OutDataTypeStr=UInt16  PortDimensions=1
  IMAPve_d_BCM_FrontWiper_State : Outport  Port=128  OutDataTypeStr=UInt16  PortDimensions=1
  IMAPve_d_BCM_CHMSL_Status : Outport  Port=129  OutDataTypeStr=UInt16  PortDimensions=1
  IMAPve_d_BCM_BrakeLamp_State : Outport  Port=130  OutDataTypeStr=UInt16  PortDimensions=1
  IMAPve_d_GW_Brake_Only_Req : Outport  Port=131  OutDataTypeStr=UInt16  PortDimensions=1
  IMAPve_d_ACU_Passenger_Belt : Outport  Port=132  OutDataTypeStr=UInt16  PortDimensions=1
  IMAPve_d_EMS_ACC_CtlAvail : Outport  Port=133  OutDataTypeStr=UInt16  PortDimensions=1
  IMAPve_d_EMS_ACC_Inhibited : Outport  Port=134  OutDataTypeStr=UInt16  PortDimensions=1
  IMAPve_d_EMS_Brake_Pedal : Outport  Port=135  OutDataTypeStr=UInt16  PortDimensions=1
  IMAPve_d_BCM_LowBeam_State : Outport  Port=136  OutDataTypeStr=UInt16  PortDimensions=1
  IMAPve_d_BCM_HighBeam_State : Outport  Port=137  OutDataTypeStr=UInt16  PortDimensions=1
  IMAPve_d_EPB_Status : Outport  Port=138  OutDataTypeStr=UInt16  PortDimensions=1
  IMAPve_d_EPB_Display_Req : Outport  Port=139  OutDataTypeStr=UInt16  PortDimensions=1
  IMAPve_d_EPB_Warn_Req : Outport  Port=140  OutDataTypeStr=UInt16  PortDimensions=1
  IMAPve_d_EPB_Switch_State : Outport  Port=141  OutDataTypeStr=UInt16  PortDimensions=1
  IMAPve_d_EPB_Switch_Valid : Outport  Port=142  OutDataTypeStr=UInt16  PortDimensions=1
  IMAPve_d_ESC_Drive_Direction : Outport  Port=143  OutDataTypeStr=UInt16  PortDimensions=1
  IMAPve_d_ESC_Hold_State : Outport  Port=144  OutDataTypeStr=UInt16  PortDimensions=1
  IMAPve_d_EPS_Steer_Hold_State : Outport  Port=145  OutDataTypeStr=UInt16  PortDimensions=1
  IMAPve_d_EPS_Warning_State : Outport  Port=146  OutDataTypeStr=UInt16  PortDimensions=1
  IMAPve_g_EPS_PowerCon : Outport  Port=147  OutDataTypeStr=T_M_Nm_Float32  PortDimensions=1
  IMAPve_d_ESC_EBD_AlarmSig : Outport  Port=148  OutDataTypeStr=UInt16  PortDimensions=1
  IMAPve_d_ESC_AVH_Status : Outport  Port=149  OutDataTypeStr=UInt16  PortDimensions=1
  IMAPve_d_Radar_Detective_Req : Outport  Port=150  OutDataTypeStr=UInt16  PortDimensions=1
  IMAPve_g_BCM_Battery_Voltage : Outport  Port=151  OutDataTypeStr=T_M_Nm_Float32  PortDimensions=1
  IMAPve_d_TBOX_LocalTimeY : Outport  Port=152  OutDataTypeStr=UInt16  PortDimensions=1
  IMAPve_d_TBOX_LocalTimeM : Outport  Port=153  OutDataTypeStr=UInt16  PortDimensions=1
  IMAPve_d_TBOX_LocalTimeD : Outport  Port=154  OutDataTypeStr=UInt16  PortDimensions=1
  IMAPve_d_TBOX_LocalTimeH : Outport  Port=155  OutDataTypeStr=UInt16  PortDimensions=1
  IMAPve_d_TBOX_LocalTimeMin : Outport  Port=156  OutDataTypeStr=UInt16  PortDimensions=1
  IMAPve_d_TBOX_LocalTimeS : Outport  Port=157  OutDataTypeStr=UInt16  PortDimensions=1
  IMAPve_d_TBOX_LocalTime_Valid : Outport  Port=158  OutDataTypeStr=UInt16  PortDimensions=1
  IMAPve_d_TPMS_Warn_Indicate : Outport  Port=159  OutDataTypeStr=UInt16  PortDimensions=1
  IMAPve_d_Radar_State : Outport  Port=160  OutDataTypeStr=UInt16  PortDimensions=1
  IMAPve_d_ACC_Desired_Headway : Outport  Port=161  OutDataTypeStr=UInt16  PortDimensions=1
  IMAPve_d_Time_System_Clock : Outport  Port=162  OutDataTypeStr=UInt16  PortDimensions=1
  IMAPve_d_Signal_Time_Stamp : Outport  Port=163  OutDataTypeStr=UInt16  PortDimensions=1
  IMAPve_g_GW_IC_Odometer : Outport  Port=164  OutDataTypeStr=UInt32  PortDimensions=1
  IMAPve_g_FAPA_State : Outport  Port=165  OutDataTypeStr=UInt32  PortDimensions=1
  IMAPve_d_Outside_Temp : Outport  Port=166  OutDataTypeStr=UInt16  PortDimensions=1
  IMAPve_d_ORI_CIPV_ID : Outport  Port=167  OutDataTypeStr=UInt16  PortDimensions=1
  IMAPve_d_ORI_Obj_Num : Outport  Port=168  OutDataTypeStr=UInt16  PortDimensions=1
  IMAPva_g_ORI_Probability : Outport  Port=169  OutDataTypeStr=T_M_Nm_Float32  PortDimensions=20
  IMAPva_d_ORI_Obj_Class : Outport  Port=170  OutDataTypeStr=UInt16  PortDimensions=20
  IMAPva_d_ORI_Obj_Motion : Outport  Port=171  OutDataTypeStr=UInt16  PortDimensions=20
  IMAPva_g_ORI_Obj_RelVel : Outport  Port=172  OutDataTypeStr=T_M_Nm_Float32  PortDimensions=20
  IMAPva_g_ORI_Obj_LongDis : Outport  Port=173  OutDataTypeStr=T_M_Nm_Float32  PortDimensions=20
  IMAPva_d_ORI_Obj_Lane : Outport  Port=174  OutDataTypeStr=UInt16  PortDimensions=20
  IMAPva_g_ORI_Obj_LAngle : Outport  Port=175  OutDataTypeStr=T_M_Nm_Float32  PortDimensions=20
  IMAPva_g_ORI_Obj_RAngle : Outport  Port=176  OutDataTypeStr=T_M_Nm_Float32  PortDimensions=20
  IMAPva_g_ORI_Obj_Width : Outport  Port=177  OutDataTypeStr=T_M_Nm_Float32  PortDimensions=20
  IMAPva_d_ORI_Obj_ID : Outport  Port=178  OutDataTypeStr=UInt16  PortDimensions=20
  IMAPve_d_ORI_Lane_Valid : Outport  Port=179  OutDataTypeStr=UInt16  PortDimensions=1
  IMAPve_d_ORI_Lane_ConsArea : Outport  Port=180  OutDataTypeStr=UInt16  PortDimensions=1
  IMAPve_d_ORI_Lane_RoadType : Outport  Port=181  OutDataTypeStr=UInt16  PortDimensions=1
  IMAPve_g_ORI_L0_C3 : Outport  Port=182  OutDataTypeStr=T_M_Nm_Float32  PortDimensions=1
  IMAPve_g_ORI_L0_C2 : Outport  Port=183  OutDataTypeStr=T_M_Nm_Float32  PortDimensions=1
  IMAPve_g_ORI_L0_C1 : Outport  Port=184  OutDataTypeStr=T_M_Nm_Float32  PortDimensions=1
  IMAPve_g_ORI_L0_C0 : Outport  Port=185  OutDataTypeStr=T_M_Nm_Float32  PortDimensions=1
  IMAPve_d_ORI_L0_Q : Outport  Port=186  OutDataTypeStr=UInt16  PortDimensions=1
  IMAPve_d_ORI_L0_Type : Outport  Port=187  OutDataTypeStr=UInt16  PortDimensions=1
  IMAPve_g_ORI_L0_VR : Outport  Port=188  OutDataTypeStr=T_M_Nm_Float32  PortDimensions=1
  IMAPve_g_ORI_L0_TLC : Outport  Port=189  OutDataTypeStr=T_M_Nm_Float32  PortDimensions=1
  IMAPve_g_ORI_L0_W : Outport  Port=190  OutDataTypeStr=T_M_Nm_Float32  PortDimensions=1
  IMAPve_d_ORI_L0_LC : Outport  Port=191  OutDataTypeStr=UInt16  PortDimensions=1
  IMAPve_g_ORI_L1_C3 : Outport  Port=192  OutDataTypeStr=T_M_Nm_Float32  PortDimensions=1
  IMAPve_g_ORI_L1_C2 : Outport  Port=193  OutDataTypeStr=T_M_Nm_Float32  PortDimensions=1
  IMAPve_g_ORI_L1_C1 : Outport  Port=194  OutDataTypeStr=T_M_Nm_Float32  PortDimensions=1
  IMAPve_g_ORI_L1_C0 : Outport  Port=195  OutDataTypeStr=T_M_Nm_Float32  PortDimensions=1
  IMAPve_d_ORI_L1_Q : Outport  Port=196  OutDataTypeStr=UInt16  PortDimensions=1
  IMAPve_d_ORI_L1_Type : Outport  Port=197  OutDataTypeStr=UInt16  PortDimensions=1
  IMAPve_g_ORI_L1_VR : Outport  Port=198  OutDataTypeStr=T_M_Nm_Float32  PortDimensions=1
  IMAPve_g_ORI_L1_TLC : Outport  Port=199  OutDataTypeStr=T_M_Nm_Float32  PortDimensions=1
  IMAPve_g_ORI_L1_W : Outport  Port=200  OutDataTypeStr=T_M_Nm_Float32  PortDimensions=1
  IMAPve_d_ORI_L1_LC : Outport  Port=201  OutDataTypeStr=UInt16  PortDimensions=1
  IMAPve_g_ORI_R0_C3 : Outport  Port=202  OutDataTypeStr=T_M_Nm_Float32  PortDimensions=1
  IMAPve_g_ORI_R0_C2 : Outport  Port=203  OutDataTypeStr=T_M_Nm_Float32  PortDimensions=1
  IMAPve_g_ORI_R0_C1 : Outport  Port=204  OutDataTypeStr=T_M_Nm_Float32  PortDimensions=1
  IMAPve_g_ORI_R0_C0 : Outport  Port=205  OutDataTypeStr=T_M_Nm_Float32  PortDimensions=1
  IMAPve_d_ORI_R0_Q : Outport  Port=206  OutDataTypeStr=UInt16  PortDimensions=1
  IMAPve_d_ORI_R0_LT : Outport  Port=207  OutDataTypeStr=UInt16  PortDimensions=1
  IMAPve_g_ORI_R0_VR : Outport  Port=208  OutDataTypeStr=T_M_Nm_Float32  PortDimensions=1
  IMAPve_g_ORI_R0_TLC : Outport  Port=209  OutDataTypeStr=T_M_Nm_Float32  PortDimensions=1
  IMAPve_g_ORI_R0_W : Outport  Port=210  OutDataTypeStr=T_M_Nm_Float32  PortDimensions=1
  IMAPve_d_ORI_R0_LC : Outport  Port=211  OutDataTypeStr=UInt16  PortDimensions=1
  IMAPve_g_ORI_R1_C3 : Outport  Port=212  OutDataTypeStr=T_M_Nm_Float32  PortDimensions=1
  IMAPve_g_ORI_R1_C2 : Outport  Port=213  OutDataTypeStr=T_M_Nm_Float32  PortDimensions=1
  IMAPve_g_ORI_R1_C1 : Outport  Port=214  OutDataTypeStr=T_M_Nm_Float32  PortDimensions=1
  IMAPve_g_ORI_R1_C0 : Outport  Port=215  OutDataTypeStr=T_M_Nm_Float32  PortDimensions=1
  IMAPve_d_ORI_R1_Q : Outport  Port=216  OutDataTypeStr=UInt16  PortDimensions=1
  IMAPve_d_ORI_R1_LT : Outport  Port=217  OutDataTypeStr=UInt16  PortDimensions=1
  IMAPve_g_ORI_R1_VR : Outport  Port=218  OutDataTypeStr=T_M_Nm_Float32  PortDimensions=1
  IMAPve_g_ORI_R1_TLC : Outport  Port=219  OutDataTypeStr=T_M_Nm_Float32  PortDimensions=1
  IMAPve_g_ORI_R1_W : Outport  Port=220  OutDataTypeStr=T_M_Nm_Float32  PortDimensions=1
  IMAPve_d_ORI_R1_LC : Outport  Port=221  OutDataTypeStr=UInt16  PortDimensions=1
  IMAPve_d_Sensor_Status : Outport  Port=222  OutDataTypeStr=UInt16  PortDimensions=1
  IMAPve_d_LF_Radar_Status : Outport  Port=223  OutDataTypeStr=UInt16  PortDimensions=1
  IMAPve_d_RF_Radar_Status : Outport  Port=224  OutDataTypeStr=UInt16  PortDimensions=1
  IMAPve_d_LR_Radar_Status : Outport  Port=225  OutDataTypeStr=UInt16  PortDimensions=1
  IMAPve_d_RR_Radar_Status : Outport  Port=226  OutDataTypeStr=UInt16  PortDimensions=1
  IMAPve_d_Fusion_Status : Outport  Port=227  OutDataTypeStr=UInt16  PortDimensions=1
  IMAPve_g_Fusion_Time_Stamp : Outport  Port=228  OutDataTypeStr=T_M_Nm_Float32  PortDimensions=1
  IMAPve_d_obj_Num : Outport  Port=229  OutDataTypeStr=UInt16  PortDimensions=1
  IMAPva_d_obj_id : Outport  Port=230  OutDataTypeStr=UInt16  PortDimensions=40
  IMAPva_g_obj_pos_x : Outport  Port=231  OutDataTypeStr=T_M_Nm_Float32  PortDimensions=40
  IMAPva_g_obj_pos_y : Outport  Port=232  OutDataTypeStr=T_M_Nm_Float32  PortDimensions=40
  IMAPva_g_obj_vel_x : Outport  Port=233  OutDataTypeStr=T_M_Nm_Float32  PortDimensions=40
  IMAPva_g_obj_vel_y : Outport  Port=234  OutDataTypeStr=T_M_Nm_Float32  PortDimensions=40
  IMAPva_g_obj_acc_x : Outport  Port=235  OutDataTypeStr=T_M_Nm_Float32  PortDimensions=40
  IMAPva_g_obj_acc_y : Outport  Port=236  OutDataTypeStr=T_M_Nm_Float32  PortDimensions=40
  IMAPva_g_obj_pos_var_x : Outport  Port=237  OutDataTypeStr=T_M_Nm_Float32  PortDimensions=40
  IMAPva_g_obj_pos_var_y : Outport  Port=238  OutDataTypeStr=T_M_Nm_Float32  PortDimensions=40
  IMAPva_g_obj_pos_var_xy : Outport  Port=239  OutDataTypeStr=T_M_Nm_Float32  PortDimensions=40
  IMAPva_g_obj_width : Outport  Port=240  OutDataTypeStr=T_M_Nm_Float32  PortDimensions=40
  IMAPva_g_obj_length : Outport  Port=241  OutDataTypeStr=T_M_Nm_Float32  PortDimensions=40
  IMAPva_d_obj_class : Outport  Port=242  OutDataTypeStr=UInt16  PortDimensions=40
  IMAPva_d_obj_lane : Outport  Port=243  OutDataTypeStr=UInt16  PortDimensions=40
  IMAPva_d_obj_status : Outport  Port=244  OutDataTypeStr=UInt16  PortDimensions=40
  IMAPva_d_obj_age : Outport  Port=245  OutDataTypeStr=UInt16  PortDimensions=40
  IMAPva_d_obj_TurnLight : Outport  Port=246  OutDataTypeStr=UInt16  PortDimensions=40
  IMAPva_d_obj_BrakeLight : Outport  Port=247  OutDataTypeStr=UInt16  PortDimensions=40
  IMAPva_d_obj_MotionStatus : Outport  Port=248  OutDataTypeStr=UInt16  PortDimensions=40
  IMAPve_d_Lane_Valid : Outport  Port=249  OutDataTypeStr=UInt16  PortDimensions=1
  IMAPve_d_Road_Type : Outport  Port=250  OutDataTypeStr=UInt16  PortDimensions=1
  IMAPve_d_ConsArea : Outport  Port=251  OutDataTypeStr=UInt16  PortDimensions=1
  IMAPve_g_L0_C0 : Outport  Port=252  OutDataTypeStr=T_M_Nm_Float32  PortDimensions=1
  IMAPve_g_L0_C1 : Outport  Port=253  OutDataTypeStr=T_M_Nm_Float32  PortDimensions=1
  IMAPve_g_L0_C2 : Outport  Port=254  OutDataTypeStr=T_M_Nm_Float32  PortDimensions=1
  IMAPve_g_L0_C3 : Outport  Port=255  OutDataTypeStr=T_M_Nm_Float32  PortDimensions=1
  IMAPve_g_L0_VR : Outport  Port=256  OutDataTypeStr=T_M_Nm_Float32  PortDimensions=1
  IMAPve_d_L0_Q : Outport  Port=257  OutDataTypeStr=UInt16  PortDimensions=1
  IMAPve_d_L0_Type : Outport  Port=258  OutDataTypeStr=UInt16  PortDimensions=1
  IMAPve_g_L0_Confidence : Outport  Port=259  OutDataTypeStr=T_M_Nm_Float32  PortDimensions=1
  IMAPve_g_L0_W : Outport  Port=260  OutDataTypeStr=T_M_Nm_Float32  PortDimensions=1
  IMAPve_g_L0_TLC : Outport  Port=261  OutDataTypeStr=T_M_Nm_Float32  PortDimensions=1
  IMAPve_d_L0_LC : Outport  Port=262  OutDataTypeStr=UInt16  PortDimensions=1
  IMAPve_g_R0_C0 : Outport  Port=263  OutDataTypeStr=T_M_Nm_Float32  PortDimensions=1
  IMAPve_g_R0_C1 : Outport  Port=264  OutDataTypeStr=T_M_Nm_Float32  PortDimensions=1
  IMAPve_g_R0_C2 : Outport  Port=265  OutDataTypeStr=T_M_Nm_Float32  PortDimensions=1
  IMAPve_g_R0_C3 : Outport  Port=266  OutDataTypeStr=T_M_Nm_Float32  PortDimensions=1
  IMAPve_g_R0_VR : Outport  Port=267  OutDataTypeStr=T_M_Nm_Float32  PortDimensions=1
  IMAPve_d_R0_Q : Outport  Port=268  OutDataTypeStr=UInt16  PortDimensions=1
  IMAPve_d_R0_Type : Outport  Port=269  OutDataTypeStr=UInt16  PortDimensions=1
  IMAPve_g_R0_Confidence : Outport  Port=270  OutDataTypeStr=T_M_Nm_Float32  PortDimensions=1
  IMAPve_g_R0_W : Outport  Port=271  OutDataTypeStr=T_M_Nm_Float32  PortDimensions=1
  IMAPve_g_R0_TLC : Outport  Port=272  OutDataTypeStr=T_M_Nm_Float32  PortDimensions=1
  IMAPve_d_R0_LC : Outport  Port=273  OutDataTypeStr=UInt16  PortDimensions=1
  IMAPve_g_L1_C0 : Outport  Port=274  OutDataTypeStr=T_M_Nm_Float32  PortDimensions=1
  IMAPve_g_L1_C1 : Outport  Port=275  OutDataTypeStr=T_M_Nm_Float32  PortDimensions=1
  IMAPve_g_L1_C2 : Outport  Port=276  OutDataTypeStr=T_M_Nm_Float32  PortDimensions=1
  IMAPve_g_L1_C3 : Outport  Port=277  OutDataTypeStr=T_M_Nm_Float32  PortDimensions=1
  IMAPve_g_L1_VR : Outport  Port=278  OutDataTypeStr=T_M_Nm_Float32  PortDimensions=1
  IMAPve_d_L1_Q : Outport  Port=279  OutDataTypeStr=UInt16  PortDimensions=1
  IMAPve_d_L1_Type : Outport  Port=280  OutDataTypeStr=UInt16  PortDimensions=1
  IMAPve_g_L1_Confidence : Outport  Port=281  OutDataTypeStr=T_M_Nm_Float32  PortDimensions=1
  IMAPve_g_L1_W : Outport  Port=282  OutDataTypeStr=T_M_Nm_Float32  PortDimensions=1
  IMAPve_g_L1_TLC : Outport  Port=283  OutDataTypeStr=T_M_Nm_Float32  PortDimensions=1
  IMAPve_d_L1_LC : Outport  Port=284  OutDataTypeStr=UInt16  PortDimensions=1
  IMAPve_g_R1_C0 : Outport  Port=285  OutDataTypeStr=T_M_Nm_Float32  PortDimensions=1
  IMAPve_g_R1_C1 : Outport  Port=286  OutDataTypeStr=T_M_Nm_Float32  PortDimensions=1
  IMAPve_g_R1_C2 : Outport  Port=287  OutDataTypeStr=T_M_Nm_Float32  PortDimensions=1
  IMAPve_g_R1_C3 : Outport  Port=288  OutDataTypeStr=T_M_Nm_Float32  PortDimensions=1
  IMAPve_g_R1_VR : Outport  Port=289  OutDataTypeStr=T_M_Nm_Float32  PortDimensions=1
  IMAPve_d_R1_Q : Outport  Port=290  OutDataTypeStr=UInt16  PortDimensions=1
  IMAPve_d_R1_Type : Outport  Port=291  OutDataTypeStr=UInt16  PortDimensions=1
  IMAPve_g_R1_Confidence : Outport  Port=292  OutDataTypeStr=T_M_Nm_Float32  PortDimensions=1
  IMAPve_g_R1_W : Outport  Port=293  OutDataTypeStr=T_M_Nm_Float32  PortDimensions=1
  IMAPve_g_R1_TLC : Outport  Port=294  OutDataTypeStr=T_M_Nm_Float32  PortDimensions=1
  IMAPve_d_R1_LC : Outport  Port=295  OutDataTypeStr=UInt16  PortDimensions=1
  IMAPve_g_L0_C0_Back : Outport  Port=296  OutDataTypeStr=T_M_Nm_Float32  PortDimensions=1
  IMAPve_g_L0_C1_Back : Outport  Port=297  OutDataTypeStr=T_M_Nm_Float32  PortDimensions=1
  IMAPve_g_L0_C2_Back : Outport  Port=298  OutDataTypeStr=T_M_Nm_Float32  PortDimensions=1
  IMAPve_g_L0_C3_Back : Outport  Port=299  OutDataTypeStr=T_M_Nm_Float32  PortDimensions=1
  IMAPve_g_L0_Range_Back : Outport  Port=300  OutDataTypeStr=T_M_Nm_Float32  PortDimensions=1
  IMAPve_g_L0_C0_FR_Pred : Outport  Port=301  OutDataTypeStr=T_M_Nm_Float32  PortDimensions=1
  IMAPve_g_L0_C1_FR_Pred : Outport  Port=302  OutDataTypeStr=T_M_Nm_Float32  PortDimensions=1
  IMAPve_g_L0_C2_FR_Pred : Outport  Port=303  OutDataTypeStr=T_M_Nm_Float32  PortDimensions=1
  IMAPve_g_L0_Range_FR_Pred : Outport  Port=304  OutDataTypeStr=T_M_Nm_Float32  PortDimensions=1
  IMAPve_g_R0_C0_Back : Outport  Port=305  OutDataTypeStr=T_M_Nm_Float32  PortDimensions=1
  IMAPve_g_R0_C1_Back : Outport  Port=306  OutDataTypeStr=T_M_Nm_Float32  PortDimensions=1
  IMAPve_g_R0_C2_Back : Outport  Port=307  OutDataTypeStr=T_M_Nm_Float32  PortDimensions=1
  IMAPve_g_R0_C3_Back : Outport  Port=308  OutDataTypeStr=T_M_Nm_Float32  PortDimensions=1
  IMAPve_g_R0_Range_Back : Outport  Port=309  OutDataTypeStr=T_M_Nm_Float32  PortDimensions=1
  IMAPve_g_R0_C0_FR_Pred : Outport  Port=310  OutDataTypeStr=T_M_Nm_Float32  PortDimensions=1
  IMAPve_g_R0_C1_FR_Pred : Outport  Port=311  OutDataTypeStr=T_M_Nm_Float32  PortDimensions=1
  IMAPve_g_R0_C2_FR_Pred : Outport  Port=312  OutDataTypeStr=T_M_Nm_Float32  PortDimensions=1
  IMAPve_g_R0_Range_FR_Pred : Outport  Port=313  OutDataTypeStr=T_M_Nm_Float32  PortDimensions=1
  IMAPve_g_L1_C0_Back : Outport  Port=314  OutDataTypeStr=T_M_Nm_Float32  PortDimensions=1
  IMAPve_g_L1_C1_Back : Outport  Port=315  OutDataTypeStr=T_M_Nm_Float32  PortDimensions=1
  IMAPve_g_L1_C2_Back : Outport  Port=316  OutDataTypeStr=T_M_Nm_Float32  PortDimensions=1
  IMAPve_g_L1_C3_Back : Outport  Port=317  OutDataTypeStr=T_M_Nm_Float32  PortDimensions=1
  IMAPve_g_L1_Range_Back : Outport  Port=318  OutDataTypeStr=T_M_Nm_Float32  PortDimensions=1
  IMAPve_g_L1_C0_FR_Pred : Outport  Port=319  OutDataTypeStr=T_M_Nm_Float32  PortDimensions=1
  IMAPve_g_L1_C1_FR_Pred : Outport  Port=320  OutDataTypeStr=T_M_Nm_Float32  PortDimensions=1
  IMAPve_g_L1_C2_FR_Pred : Outport  Port=321  OutDataTypeStr=T_M_Nm_Float32  PortDimensions=1
  IMAPve_g_L1_Range_FR_Pred : Outport  Port=322  OutDataTypeStr=T_M_Nm_Float32  PortDimensions=1
  IMAPve_g_R1_C0_Back : Outport  Port=323  OutDataTypeStr=T_M_Nm_Float32  PortDimensions=1
  IMAPve_g_R1_C1_Back : Outport  Port=324  OutDataTypeStr=T_M_Nm_Float32  PortDimensions=1
  IMAPve_g_R1_C2_Back : Outport  Port=325  OutDataTypeStr=T_M_Nm_Float32  PortDimensions=1
  IMAPve_g_R1_C3_Back : Outport  Port=326  OutDataTypeStr=T_M_Nm_Float32  PortDimensions=1
  IMAPve_g_R1_Range_Back : Outport  Port=327  OutDataTypeStr=T_M_Nm_Float32  PortDimensions=1
  IMAPve_g_R1_C0_FR_Pred : Outport  Port=328  OutDataTypeStr=T_M_Nm_Float32  PortDimensions=1
  IMAPve_g_R1_C1_FR_Pred : Outport  Port=329  OutDataTypeStr=T_M_Nm_Float32  PortDimensions=1
  IMAPve_g_R1_C2_FR_Pred : Outport  Port=330  OutDataTypeStr=T_M_Nm_Float32  PortDimensions=1
  IMAPve_g_R1_Range_FR_Pred : Outport  Port=331  OutDataTypeStr=T_M_Nm_Float32  PortDimensions=1
  IMAPve_d_Sign_ISA_Value : Outport  Port=332  OutDataTypeStr=UInt16  PortDimensions=1
  IMAPve_d_TSR_Sign_Type : Outport  Port=333  OutDataTypeStr=UInt16  PortDimensions=1
  IMAPve_d_Camera_Signal_Fault : Outport  Port=334  OutDataTypeStr=UInt16  PortDimensions=1
  IMAPve_d_Radar_Status : Outport  Port=335  OutDataTypeStr=UInt16  PortDimensions=1
  IMAPve_d_Camera_Status : Outport  Port=336  OutDataTypeStr=UInt16  PortDimensions=1
  IMAPve_d_ESC_FLW_Direction : Outport  Port=337  OutDataTypeStr=UInt16
  IMAPve_d_ESC_FRW_Direction : Outport  Port=338  OutDataTypeStr=UInt16
  IMAPve_d_ESC_TCS_ErrorStatus : Outport  Port=339  OutDataTypeStr=UInt16
  IMAPve_d_ESC_RLW_Direction : Outport  Port=340  OutDataTypeStr=UInt16
  IMAPve_d_ESC_RRW_Direction : Outport  Port=341  OutDataTypeStr=UInt16
  IMAPve_d_ESC_EPB_ErrorStatus : Outport  Port=342  OutDataTypeStr=UInt16
  IMAPve_d_EPS_SteeringAngle_Flag : Outport  Port=343  OutDataTypeStr=UInt16
  IMAPve_g_EPS_SteeringAngle : Outport  Port=344  OutDataTypeStr=T_M_Nm_Float32
  IMAPve_d_EPS_Driver_Override : Outport  Port=345  OutDataTypeStr=UInt16
  IMAPve_d_EPS_Driver_Active_ESA : Outport  Port=346  OutDataTypeStr=UInt16
  IMAPve_d_EPS_ESA_State : Outport  Port=347  OutDataTypeStr=UInt16
  IMAPve_d_ACU_RearLeft_Belt : Outport  Port=348  OutDataTypeStr=UInt16
  IMAPve_d_ACU_RearMiddle_Belt : Outport  Port=349  OutDataTypeStr=UInt16
  IMAPve_d_ACU_RearRight_Belt : Outport  Port=350  OutDataTypeStr=UInt16
  IMAPve_d_EMS_PowertrainCtl_State : Outport  Port=351  OutDataTypeStr=UInt16
  IMAPve_d_TCU_TCU_Available : Outport  Port=352  OutDataTypeStr=UInt16
  IMAPve_d_BCM_LeftTurn_Switch : Outport  Port=353  OutDataTypeStr=UInt16
  IMAPve_d_BCM_RightTurn_Switch : Outport  Port=354  OutDataTypeStr=UInt16
  IMAPve_d_BCM_FrontWiper_Switch : Outport  Port=355  OutDataTypeStr=UInt16
  IMAPve_d_BCM_IHBC_Enabled : Outport  Port=356  OutDataTypeStr=UInt16
  IMAPve_d_MP5_Work_State : Outport  Port=357  OutDataTypeStr=UInt16
  IMAPve_d_MP5_APA_ModeSelect : Outport  Port=358  OutDataTypeStr=UInt16
  IMAPve_d_MP5_LanguageSet : Outport  Port=359  OutDataTypeStr=UInt16
  IMAPve_d_MP5_UPA_Switch : Outport  Port=360  OutDataTypeStr=UInt16
  IMAPve_d_MP5_FLK_Activation : Outport  Port=361  OutDataTypeStr=UInt16
  IMAPve_d_MP5_AutoPilot_Switch : Outport  Port=362  OutDataTypeStr=UInt16
  IMAPve_d_MP5_DMS_MessageType : Outport  Port=363  OutDataTypeStr=UInt16
  IMAPve_d_MP5_DMS_SystemEnable : Outport  Port=364  OutDataTypeStr=UInt16
  IMAPve_d_MP5_DMS_DelUserNum : Outport  Port=365  OutDataTypeStr=UInt16
  IMAPve_d_MP5_DMS_Sensity : Outport  Port=366  OutDataTypeStr=UInt16
  IMAPve_d_MP5_DMS_EyeFatigue : Outport  Port=367  OutDataTypeStr=UInt16
  IMAPve_d_MP5_DMS_LongtimeDrive : Outport  Port=368  OutDataTypeStr=UInt16
  IMAPve_d_MP5_DMS_SideView : Outport  Port=369  OutDataTypeStr=UInt16
  IMAPve_d_MP5_DMS_UsingPhone : Outport  Port=370  OutDataTypeStr=UInt16
  IMAPve_d_MP5_DMS_Smoking : Outport  Port=371  OutDataTypeStr=UInt16
  IMAPve_d_MP5_DMS_DrinkWater : Outport  Port=372  OutDataTypeStr=UInt16
  IMAPve_d_MP5_DMS_UserAccount : Outport  Port=373  OutDataTypeStr=UInt16
  IMAPve_d_High_Beam_State : Outport  Port=374  OutDataTypeStr=UInt16
  IMAPve_d_Front_Fog_Lamp_State : Outport  Port=375  OutDataTypeStr=UInt16
  IMAPve_d_Rear_Fog_Lamp_State : Outport  Port=376  OutDataTypeStr=UInt16
  IMAPve_d_BCM_Rain_Intensity : Outport  Port=377  OutDataTypeStr=UInt16
  IMAPve_d_BCM_OvertakinglampSwt : Outport  Port=378  OutDataTypeStr=UInt16
  IMAPve_d_EMS_Kickdown : Outport  Port=379  OutDataTypeStr=UInt16
  IMAPve_g_EMS_Mech_Loss_Trq : Outport  Port=380  OutDataTypeStr=T_M_Nm_Float32
  IMAPve_d_Powertrain_Torque_Valid : Outport  Port=381  OutDataTypeStr=UInt16
  IMAPve_d_ESC_ACCInfo_Error : Outport  Port=382  OutDataTypeStr=UInt16
  IMAPve_d_ESC_Prefill_Response : Outport  Port=383  OutDataTypeStr=UInt16
  IMAPve_d_ESC_AEBJerk_Response : Outport  Port=384  OutDataTypeStr=UInt16
  IMAPve_d_ESC_FCW_DBS_Response : Outport  Port=385  OutDataTypeStr=UInt16
  IMAPve_d_ESC_AEBJerk_Available : Outport  Port=386  OutDataTypeStr=UInt16
  IMAPve_d_ESC_FCW_DBS_Available : Outport  Port=387  OutDataTypeStr=UInt16
  IMAPve_d_ESC_Prefill_Available : Outport  Port=388  OutDataTypeStr=UInt16
  IMAPve_g_EPS_LKAOverlay_Trq : Outport  Port=389  OutDataTypeStr=T_M_Nm_Float32
  IMAPve_g_EPS_DriverTorque : Outport  Port=390  OutDataTypeStr=T_M_Nm_Float32
  IMAPve_d_EPS_Steer_Hold_State_Valid : Outport  Port=391  OutDataTypeStr=UInt16
  IMAPva_d_ORI_Obj_TimeStamp : Outport  Port=392  OutDataTypeStr=UInt16  PortDimensions=20
  IMAPve_d_ORI_FS_OutOfCalib : Outport  Port=393  OutDataTypeStr=UInt16
  IMAPve_d_ORI_FS_Rain : Outport  Port=394  OutDataTypeStr=UInt16
  IMAPve_d_ORI_FS_Fog : Outport  Port=395  OutDataTypeStr=UInt16
  IMAPve_d_ORI_FS_Splashes0 : Outport  Port=396  OutDataTypeStr=UInt16
  IMAPve_d_ORI_FS_SunRay0 : Outport  Port=397  OutDataTypeStr=UInt16
  IMAPve_d_ORI_FS_LowSun0 : Outport  Port=398  OutDataTypeStr=UInt16
  IMAPve_d_ORI_FS_BlurImage0 : Outport  Port=399  OutDataTypeStr=UInt16
  IMAPve_d_ORI_FS_PartialBlockage0 : Outport  Port=400  OutDataTypeStr=UInt16
  IMAPve_d_ORI_FS_FullBlockage0 : Outport  Port=401  OutDataTypeStr=UInt16
  IMAPve_d_ORI_FS_FrozenWindshield0 : Outport  Port=402  OutDataTypeStr=UInt16
  IMAPve_d_ORI_FS_OutOfFocus0 : Outport  Port=403  OutDataTypeStr=UInt16
  IMAPva_g_ORI_Obj_AbsAx : Outport  Port=404  OutDataTypeStr=T_M_Nm_Float32  PortDimensions=20
  IMAPva_g_ORI_Obj_AbsAy : Outport  Port=405  OutDataTypeStr=T_M_Nm_Float32  PortDimensions=20
  IMAPva_g_ORI_Obj_TTIPCStdDev : Outport  Port=406  OutDataTypeStr=T_M_Nm_Float32  PortDimensions=20
  IMAPva_g_ORI_Obj_RelVely : Outport  Port=407  OutDataTypeStr=T_M_Nm_Float32  PortDimensions=20
  IMAPva_g_ORI_Obj_LateralDis : Outport  Port=408  OutDataTypeStr=T_M_Nm_Float32  PortDimensions=20
  IMAPva_g_ORI_Obj_AbsAxStdDev : Outport  Port=409  OutDataTypeStr=T_M_Nm_Float32  PortDimensions=20
  IMAPva_g_ORI_Obj_AbsAyStdDev : Outport  Port=410  OutDataTypeStr=T_M_Nm_Float32  PortDimensions=20
  IMAPva_g_ORI_Obj_RelVelStdDev : Outport  Port=411  OutDataTypeStr=T_M_Nm_Float32  PortDimensions=20
  IMAPva_g_ORI_Obj_RelVelyStdDev : Outport  Port=412  OutDataTypeStr=T_M_Nm_Float32  PortDimensions=20
  IMAPva_g_ORI_Obj_LongDisStdDev : Outport  Port=413  OutDataTypeStr=T_M_Nm_Float32  PortDimensions=20
  IMAPva_g_ORI_Obj_LateralDisStdDev : Outport  Port=414  OutDataTypeStr=T_M_Nm_Float32  PortDimensions=20
  IMAPva_d_ORI_Obj_RelVelValid : Outport  Port=415  OutDataTypeStr=UInt16  PortDimensions=20
  IMAPva_d_ORI_Obj_RelVelyValid : Outport  Port=416  OutDataTypeStr=UInt16  PortDimensions=20
  IMAPva_d_ORI_Obj_RelVelStdDevValid : Outport  Port=417  OutDataTypeStr=UInt16  PortDimensions=20
  IMAPva_d_ORI_Obj_RelVelyStdDevValid : Outport  Port=418  OutDataTypeStr=UInt16  PortDimensions=20
  IMAPva_g_ORI_Obj_ExistProb : Outport  Port=419  OutDataTypeStr=T_M_Nm_Float32  PortDimensions=20
  IMAPva_g_ORI_Obj_ClassProb : Outport  Port=420  OutDataTypeStr=T_M_Nm_Float32  PortDimensions=20
  IMAPva_g_ORI_Obj_Height : Outport  Port=421  OutDataTypeStr=T_M_Nm_Float32  PortDimensions=20
  IMAPva_g_ORI_Obj_LengthStdDev : Outport  Port=422  OutDataTypeStr=T_M_Nm_Float32  PortDimensions=20
  IMAPva_g_ORI_Obj_WidthStdDev : Outport  Port=423  OutDataTypeStr=T_M_Nm_Float32  PortDimensions=20
  IMAPva_g_ORI_Obj_HeightStdDev : Outport  Port=424  OutDataTypeStr=T_M_Nm_Float32  PortDimensions=20
  IMAPva_g_ORI_Obj_3DAngle : Outport  Port=425  OutDataTypeStr=T_M_Nm_Float32  PortDimensions=20
  IMAPva_g_ORI_Obj_LAngleStdDev : Outport  Port=426  OutDataTypeStr=T_M_Nm_Float32  PortDimensions=20
  IMAPva_g_ORI_Obj_RAngleStdDev : Outport  Port=427  OutDataTypeStr=T_M_Nm_Float32  PortDimensions=20
  IMAPva_g_ORI_Obj_3DAngleStdDev : Outport  Port=428  OutDataTypeStr=T_M_Nm_Float32  PortDimensions=20
  IMAPva_g_ORI_Obj_AngleRate : Outport  Port=429  OutDataTypeStr=T_M_Nm_Float32  PortDimensions=20
  IMAPva_g_ORI_Obj_AngleRateStdDev : Outport  Port=430  OutDataTypeStr=T_M_Nm_Float32  PortDimensions=20
  IMAPva_g_ORI_Obj_PhiBottom : Outport  Port=431  OutDataTypeStr=T_M_Nm_Float32  PortDimensions=20
  IMAPva_g_ORI_Obj_PhiBottomStdDev : Outport  Port=432  OutDataTypeStr=T_M_Nm_Float32  PortDimensions=20
  IMAPva_d_ORI_Obj_Measured : Outport  Port=433  OutDataTypeStr=UInt16  PortDimensions=20
  IMAPva_g_ORI_Obj_Heading : Outport  Port=434  OutDataTypeStr=T_M_Nm_Float32  PortDimensions=20
  IMAPva_g_ORI_Obj_HeadingStdDev : Outport  Port=435  OutDataTypeStr=T_M_Nm_Float32  PortDimensions=20
  IMAPva_d_ORI_Obj_HeadOrientation : Outport  Port=436  OutDataTypeStr=UInt16  PortDimensions=20
  IMAPva_g_ORI_Obj_TTIPC : Outport  Port=437  OutDataTypeStr=T_M_Nm_Float32  PortDimensions=20
  IMAPva_d_ORI_Obj_DirectionIndicator : Outport  Port=438  OutDataTypeStr=UInt16  PortDimensions=20
  IMAPva_d_ORI_Obj_BrakeLight : Outport  Port=439  OutDataTypeStr=UInt16  PortDimensions=20
  IMAPve_d_ORI_L0_ID : Outport  Port=440  OutDataTypeStr=UInt16
  IMAPve_g_ORI_L0_ExistProb : Outport  Port=441  OutDataTypeStr=T_M_Nm_Float32
  IMAPve_g_ORI_L0_DxStart : Outport  Port=442  OutDataTypeStr=T_M_Nm_Float32
  IMAPve_d_ORI_L0_ColorClass : Outport  Port=443  OutDataTypeStr=UInt16
  IMAPve_d_ORI_L0_MeasureType : Outport  Port=444  OutDataTypeStr=UInt16
  IMAPve_g_ORI_L0_TypeConf : Outport  Port=445  OutDataTypeStr=T_M_Nm_Float32
  IMAPve_d_ORI_R0_ID : Outport  Port=446  OutDataTypeStr=UInt16
  IMAPve_g_ORI_R0_ExistProb : Outport  Port=447  OutDataTypeStr=T_M_Nm_Float32
  IMAPve_g_ORI_R0_Dxstart : Outport  Port=448  OutDataTypeStr=T_M_Nm_Float32
  IMAPve_d_ORI_R0_ColorClass : Outport  Port=449  OutDataTypeStr=UInt16
  IMAPve_d_ORI_R0_MeasureType : Outport  Port=450  OutDataTypeStr=UInt16
  IMAPve_g_ORI_R0_TypeConf : Outport  Port=451  OutDataTypeStr=T_M_Nm_Float32
  IMAPve_d_ORI_L1_ID : Outport  Port=452  OutDataTypeStr=UInt16
  IMAPve_g_ORI_L1_ExistProb : Outport  Port=453  OutDataTypeStr=T_M_Nm_Float32
  IMAPve_g_ORI_L1_Dxstart : Outport  Port=454  OutDataTypeStr=T_M_Nm_Float32
  IMAPve_d_ORI_L1_ColorClass : Outport  Port=455  OutDataTypeStr=UInt16
  IMAPve_d_ORI_L1_MeasureType : Outport  Port=456  OutDataTypeStr=UInt16
  IMAPve_g_ORI_L1_TypeConf : Outport  Port=457  OutDataTypeStr=T_M_Nm_Float32
  IMAPve_d_ORI_R1_ID : Outport  Port=458  OutDataTypeStr=UInt16
  IMAPve_g_ORI_R1_ExistProb : Outport  Port=459  OutDataTypeStr=T_M_Nm_Float32
  IMAPve_g_ORI_R1_Dxstart : Outport  Port=460  OutDataTypeStr=T_M_Nm_Float32
  IMAPve_d_ORI_R1_ColorClass : Outport  Port=461  OutDataTypeStr=UInt16
  IMAPve_d_ORI_R1_MeasureType : Outport  Port=462  OutDataTypeStr=UInt16
  IMAPve_g_ORI_R1_TypeConf : Outport  Port=463  OutDataTypeStr=T_M_Nm_Float32
  IMAPve_d_ORI_RoadedgeL0_ID : Outport  Port=464  OutDataTypeStr=UInt16
  IMAPve_g_ORI_RoadedgeL0_ExistProb : Outport  Port=465  OutDataTypeStr=T_M_Nm_Float32
  IMAPve_g_ORI_RoadedgeL0_DxStart : Outport  Port=466  OutDataTypeStr=T_M_Nm_Float32
  IMAPve_g_ORI_RoadedgeL0_DxEnd : Outport  Port=467  OutDataTypeStr=T_M_Nm_Float32
  IMAPve_g_ORI_RoadedgeL0_C1 : Outport  Port=468  OutDataTypeStr=T_M_Nm_Float32
  IMAPve_g_ORI_RoadedgeL0_C0 : Outport  Port=469  OutDataTypeStr=T_M_Nm_Float32
  IMAPve_g_ORI_RoadedgeL0_C3 : Outport  Port=470  OutDataTypeStr=T_M_Nm_Float32
  IMAPve_g_ORI_RoadedgeL0_C2 : Outport  Port=471  OutDataTypeStr=T_M_Nm_Float32
  IMAPve_d_ORI_RoadedgeL0_MeasureType : Outport  Port=472  OutDataTypeStr=UInt16
  IMAPve_d_ORI_RoadedgeL0_Type : Outport  Port=473  OutDataTypeStr=UInt16
  IMAPve_d_ORI_RoadedgeR0_ID : Outport  Port=474  OutDataTypeStr=UInt16
  IMAPve_g_ORI_RoadedgeR0_ExistProb : Outport  Port=475  OutDataTypeStr=T_M_Nm_Float32
  IMAPve_g_ORI_RoadedgeR0_DxStart : Outport  Port=476  OutDataTypeStr=T_M_Nm_Float32
  IMAPve_g_ORI_RoadedgeR0_DxEnd : Outport  Port=477  OutDataTypeStr=T_M_Nm_Float32
  IMAPve_g_ORI_RoadedgeR0_C1 : Outport  Port=478  OutDataTypeStr=T_M_Nm_Float32
  IMAPve_g_ORI_RoadedgeR0_C0 : Outport  Port=479  OutDataTypeStr=T_M_Nm_Float32
  IMAPve_g_ORI_RoadedgeR0_C3 : Outport  Port=480  OutDataTypeStr=T_M_Nm_Float32
  IMAPve_g_ORI_RoadedgeR0_C2 : Outport  Port=481  OutDataTypeStr=T_M_Nm_Float32
  IMAPve_d_ORI_RoadedgeR0_MeasureType : Outport  Port=482  OutDataTypeStr=UInt16
  IMAPve_d_ORI_RoadedgeR0_Type : Outport  Port=483  OutDataTypeStr=UInt16
  wires:
  Runnable_IMAP_10ms_sys/417(IMAPva_d_ORI_Obj_RelVelStdDevValid) -> IMAPva_d_ORI_Obj_RelVelStdDevValid/1
  Runnable_IMAP_10ms_sys/455(IMAPve_d_ORI_L1_ColorClass) -> IMAPve_d_ORI_L1_ColorClass/1
  Runnable_IMAP_10ms_sys/456(IMAPve_d_ORI_L1_MeasureType) -> IMAPve_d_ORI_L1_MeasureType/1
  Runnable_IMAP_10ms_sys/437(IMAPva_g_ORI_Obj_TTIPC) -> IMAPva_g_ORI_Obj_TTIPC/1
  Runnable_IMAP_10ms_sys/404(IMAPva_g_ORI_Obj_AbsAx) -> IMAPva_g_ORI_Obj_AbsAx/1
  Runnable_IMAP_10ms_sys/463(IMAPve_g_ORI_R1_TypeConf) -> IMAPve_g_ORI_R1_TypeConf/1
  Runnable_IMAP_10ms_sys/480(IMAPve_g_ORI_RoadedgeR0_C3) -> IMAPve_g_ORI_RoadedgeR0_C3/1
  Runnable_IMAP_10ms_sys/395(IMAPve_d_ORI_FS_Fog) -> IMAPve_d_ORI_FS_Fog/1
  Runnable_IMAP_10ms_sys/414(IMAPva_g_ORI_Obj_LateralDisStdDev) -> IMAPva_g_ORI_Obj_LateralDisStdDev/1
  Runnable_IMAP_10ms_sys/433(IMAPva_d_ORI_Obj_Measured) -> IMAPva_d_ORI_Obj_Measured/1
  Runnable_IMAP_10ms_sys/443(IMAPve_d_ORI_L0_ColorClass) -> IMAPve_d_ORI_L0_ColorClass/1
  Runnable_IMAP_10ms_sys/406(IMAPva_g_ORI_Obj_TTIPCStdDev) -> IMAPva_g_ORI_Obj_TTIPCStdDev/1
  Runnable_IMAP_10ms_sys/403(IMAPve_d_ORI_FS_OutOfFocus0) -> IMAPve_d_ORI_FS_OutOfFocus0/1
  Runnable_IMAP_10ms_sys/416(IMAPva_d_ORI_Obj_RelVelyValid) -> IMAPva_d_ORI_Obj_RelVelyValid/1
  Runnable_IMAP_10ms_sys/472(IMAPve_d_ORI_RoadedgeL0_MeasureType) -> IMAPve_d_ORI_RoadedgeL0_MeasureType/1
  Runnable_IMAP_10ms_sys/407(IMAPva_g_ORI_Obj_RelVely) -> IMAPva_g_ORI_Obj_RelVely/1
  Runnable_IMAP_10ms_sys/474(IMAPve_d_ORI_RoadedgeR0_ID) -> IMAPve_d_ORI_RoadedgeR0_ID/1
  Runnable_IMAP_10ms_sys/394(IMAPve_d_ORI_FS_Rain) -> IMAPve_d_ORI_FS_Rain/1
  Runnable_IMAP_10ms_sys/425(IMAPva_g_ORI_Obj_3DAngle) -> IMAPva_g_ORI_Obj_3DAngle/1
  Runnable_IMAP_10ms_sys/431(IMAPva_g_ORI_Obj_PhiBottom) -> IMAPva_g_ORI_Obj_PhiBottom/1
  Runnable_IMAP_10ms_sys/423(IMAPva_g_ORI_Obj_WidthStdDev) -> IMAPva_g_ORI_Obj_WidthStdDev/1
  Runnable_IMAP_10ms_sys/458(IMAPve_d_ORI_R1_ID) -> IMAPve_d_ORI_R1_ID/1
  Runnable_IMAP_10ms_sys/461(IMAPve_d_ORI_R1_ColorClass) -> IMAPve_d_ORI_R1_ColorClass/1
  Runnable_IMAP_10ms_sys/415(IMAPva_d_ORI_Obj_RelVelValid) -> IMAPva_d_ORI_Obj_RelVelValid/1
  Runnable_IMAP_10ms_sys/451(IMAPve_g_ORI_R0_TypeConf) -> IMAPve_g_ORI_R0_TypeConf/1
  Runnable_IMAP_10ms_sys/418(IMAPva_d_ORI_Obj_RelVelyStdDevValid) -> IMAPva_d_ORI_Obj_RelVelyStdDevValid/1
  Runnable_IMAP_10ms_sys/483(IMAPve_d_ORI_RoadedgeR0_Type) -> IMAPve_d_ORI_RoadedgeR0_Type/1
  CAFDva_y_F_CameraData45F/1 -> Runnable_IMAP_10ms_sys/239(CAFDva_y_F_CameraData45F)
  Runnable_IMAP_10ms_sys/325(IMAPve_g_R1_C2_Back) -> IMAPve_g_R1_C2_Back/1
  Runnable_IMAP_10ms_sys/29(IMAPve_d_EPS_Trq_State) -> IMAPve_d_EPS_Trq_State/1
  Runnable_IMAP_10ms_sys/244(IMAPva_d_obj_status) -> IMAPva_d_obj_status/1
  SWINve_y_Left_Turn_Lamp_Status/1 -> Runnable_IMAP_10ms_sys/204(SWINve_y_BCM_LeftlightSt)
  Runnable_IMAP_10ms_sys/355(IMAPve_d_BCM_FrontWiper_Switch) -> IMAPve_d_BCM_FrontWiper_Switch/1
  Runnable_IMAP_10ms_sys/118(IMAPve_d_EMS_Engine_Status) -> IMAPve_d_EMS_Engine_Status/1
  Runnable_IMAP_10ms_sys/274(IMAPve_g_L1_C0) -> IMAPve_g_L1_C0/1
  Runnable_IMAP_10ms_sys/289(IMAPve_g_R1_VR) -> IMAPve_g_R1_VR/1
  Runnable_IMAP_10ms_sys/123(IMAPve_d_ESC_AEB_Active) -> IMAPve_d_ESC_AEB_Active/1
  Runnable_IMAP_10ms_sys/186(IMAPve_d_ORI_L0_Q) -> IMAPve_d_ORI_L0_Q/1
  SWINve_d_engine_revolution_speed/1 -> Runnable_IMAP_10ms_sys/11(SWINve_d_EMS_Engine_RPM)
  Runnable_IMAP_10ms_sys/52(IMAPve_d_BCM_Opening_State) -> IMAPve_d_BCM_Opening_State/1
  Runnable_IMAP_10ms_sys/156(IMAPve_d_TBOX_LocalTimeMin) -> IMAPve_d_TBOX_LocalTimeMin/1
  Runnable_IMAP_10ms_sys/242(IMAPva_d_obj_class) -> IMAPva_d_obj_class/1
  Runnable_IMAP_10ms_sys/66(IMAPve_g_EMS_MaxTWhl) -> IMAPve_g_EMS_MaxTWhl/1
  CAFDva_y_F_CameraData45D/1 -> Runnable_IMAP_10ms_sys/237(CAFDva_y_F_CameraData45D)
  SWINve_g_EPS1_IND_DriverTorque_Value/1 -> Runnable_IMAP_10ms_sys/227(SWINve_g_EPS1_IND_DriverTorque_Value)
  CAFDva_y_F_CameraData426/1 -> Runnable_IMAP_10ms_sys/252(CAFDva_y_F_CameraData426)
  SWINve_y_brake_pedal_status/1 -> Runnable_IMAP_10ms_sys/6(SWINve_y_Brake_secondary_contact)
  SDFAve_y_ROAD_TYPE/1 -> Runnable_IMAP_10ms_sys/87(SDFAve_y_ROAD_TYPE)
  SDFAva_g_obj_acc_y/1 -> Runnable_IMAP_10ms_sys/73(SDFAva_g_obj_acc_y)
  SWINve_g_wheel_speed_RR/1 -> Runnable_IMAP_10ms_sys/35(SWINve_g_No_filtered_rear_rignt_speed)
  SDFAve_g_R1_MARK_WIDTH/1 -> Runnable_IMAP_10ms_sys/130(SDFAve_g_R1_MARK_WIDTH)
  Runnable_IMAP_10ms_sys/196(IMAPve_d_ORI_L1_Q) -> IMAPve_d_ORI_L1_Q/1
  Runnable_IMAP_10ms_sys/273(IMAPve_d_R0_LC) -> IMAPve_d_R0_LC/1
  Runnable_IMAP_10ms_sys/292(IMAPve_g_R1_Confidence) -> IMAPve_g_R1_Confidence/1
  Runnable_IMAP_10ms_sys/310(IMAPve_g_R0_C0_FR_Pred) -> IMAPve_g_R0_C0_FR_Pred/1
  Runnable_IMAP_10ms_sys/111(IMAPve_d_ESC_RL_Wheel_Pulse) -> IMAPve_d_ESC_RL_Wheel_Pulse/1
  System_Clock/1 -> Runnable_IMAP_10ms_sys/58(System_Clock)
  Runnable_IMAP_10ms_sys/388(IMAPve_d_ESC_Prefill_Available) -> IMAPve_d_ESC_Prefill_Available/1
  Runnable_IMAP_10ms_sys/158(IMAPve_d_TBOX_LocalTime_Valid) -> IMAPve_d_TBOX_LocalTime_Valid/1
  SDFAva_g_obj_length/1 -> Runnable_IMAP_10ms_sys/78(SDFAva_g_obj_length)
  Runnable_IMAP_10ms_sys/64(IMAPve_g_EMS_Pot_WhlT_Min) -> IMAPve_g_EMS_Pot_WhlT_Min/1
  Runnable_IMAP_10ms_sys/27(IMAPve_g_EPS_SW_Trq) -> IMAPve_g_EPS_SW_Trq/1
  Runnable_IMAP_10ms_sys/72(IMAPve_g_EMS_Realize_TWhl) -> IMAPve_g_EMS_Realize_TWhl/1
  Runnable_IMAP_10ms_sys/208(IMAPve_g_ORI_R0_VR) -> IMAPve_g_ORI_R0_VR/1
  Runnable_IMAP_10ms_sys/56(IMAPve_d_BCM_RR_Door_State) -> IMAPve_d_BCM_RR_Door_State/1
  CAFDva_y_F_CameraData452/1 -> Runnable_IMAP_10ms_sys/245(CAFDva_y_F_CameraData452)
  SWINve_g_AC1_Status_AmbientTemp_Lvl/1 -> Runnable_IMAP_10ms_sys/190(SWINve_g_AC_AmbTemp)
  Runnable_IMAP_10ms_sys/149(IMAPve_d_ESC_AVH_Status) -> IMAPve_d_ESC_AVH_Status/1
  SDFAve_g_L0_TLC/1 -> Runnable_IMAP_10ms_sys/98(SDFAve_g_L0_TLC)
  Runnable_IMAP_10ms_sys/359(IMAPve_d_MP5_LanguageSet) -> IMAPve_d_MP5_LanguageSet/1
  Runnable_IMAP_10ms_sys/481(IMAPve_g_ORI_RoadedgeR0_C2) -> IMAPve_g_ORI_RoadedgeR0_C2/1
  SDFAve_g_R0_MARK_WIDTH/1 -> Runnable_IMAP_10ms_sys/108(SDFAve_g_R0_MARK_WIDTH)
  Runnable_IMAP_10ms_sys/299(IMAPve_g_L0_C3_Back) -> IMAPve_g_L0_C3_Back/1
  Runnable_IMAP_10ms_sys/171(IMAPva_d_ORI_Obj_Motion) -> IMAPva_d_ORI_Obj_Motion/1
  SWINve_y_Engine1_Status_DASReq_Resp/1 -> Runnable_IMAP_10ms_sys/19(SWINve_y_GW_EMS_EMS_Status_ACC)
  Runnable_IMAP_10ms_sys/85(IMAPve_d_SWS_Failure_Status) -> IMAPve_d_SWS_Failure_Status/1
  CAFDva_y_F_CameraData456/1 -> Runnable_IMAP_10ms_sys/249(CAFDva_y_F_CameraData456)
  Runnable_IMAP_10ms_sys/271(IMAPve_g_R0_W) -> IMAPve_g_R0_W/1
  Runnable_IMAP_10ms_sys/117(IMAPve_d_TCU_Select_ATMode) -> IMAPve_d_TCU_Select_ATMode/1
  SWINve_y_ESP_Status_FCW_DBS_Response/1 -> Runnable_IMAP_10ms_sys/222(SWINve_y_ESP_Status_FCW_DBS_Response)
  Runnable_IMAP_10ms_sys/90(IMAPve_d_ESC_MSR_Active) -> IMAPve_d_ESC_MSR_Active/1
  Runnable_IMAP_10ms_sys/120(IMAPve_d_ESC_Brake_Failsafe) -> IMAPve_d_ESC_Brake_Failsafe/1
  Runnable_IMAP_10ms_sys/445(IMAPve_g_ORI_L0_TypeConf) -> IMAPve_g_ORI_L0_TypeConf/1
  Runnable_IMAP_10ms_sys/49(IMAPve_d_BCM_Left_Light) -> IMAPve_d_BCM_Left_Light/1
  Runnable_IMAP_10ms_sys/253(IMAPve_g_L0_C1) -> IMAPve_g_L0_C1/1
  SDFAve_g_L0_C3_BACK_COEF/1 -> Runnable_IMAP_10ms_sys/136(SDFAve_g_L0_C3_BACK_COEF)
  SWINve_y_EBD_fault/1 -> Runnable_IMAP_10ms_sys/203(SWINve_y_ESC_EBDAlarmSig)
  Runnable_IMAP_10ms_sys/353(IMAPve_d_BCM_LeftTurn_Switch) -> IMAPve_d_BCM_LeftTurn_Switch/1
  Runnable_IMAP_10ms_sys/142(IMAPve_d_EPB_Switch_Valid) -> IMAPve_d_EPB_Switch_Valid/1
  Runnable_IMAP_10ms_sys/213(IMAPve_g_ORI_R1_C2) -> IMAPve_g_ORI_R1_C2/1
  Runnable_IMAP_10ms_sys/134(IMAPve_d_EMS_ACC_Inhibited) -> IMAPve_d_EMS_ACC_Inhibited/1
  Runnable_IMAP_10ms_sys/283(IMAPve_g_L1_TLC) -> IMAPve_g_L1_TLC/1
  Runnable_IMAP_10ms_sys/468(IMAPve_g_ORI_RoadedgeL0_C1) -> IMAPve_g_ORI_RoadedgeL0_C1/1
  Runnable_IMAP_10ms_sys/157(IMAPve_d_TBOX_LocalTimeS) -> IMAPve_d_TBOX_LocalTimeS/1
  Runnable_IMAP_10ms_sys/347(IMAPve_d_EPS_ESA_State) -> IMAPve_d_EPS_ESA_State/1
  Runnable_IMAP_10ms_sys/264(IMAPve_g_R0_C1) -> IMAPve_g_R0_C1/1
  Runnable_IMAP_10ms_sys/469(IMAPve_g_ORI_RoadedgeL0_C0) -> IMAPve_g_ORI_RoadedgeL0_C0/1
  Runnable_IMAP_10ms_sys/60(IMAPve_d_PEPS_Door_Lock_Req) -> IMAPve_d_PEPS_Door_Lock_Req/1
  SDFAve_y_R1_DETECT_QUALITY/1 -> Runnable_IMAP_10ms_sys/127(SDFAve_y_R1_DETECT_QUALITY)
  Runnable_IMAP_10ms_sys/398(IMAPve_d_ORI_FS_LowSun0) -> IMAPve_d_ORI_FS_LowSun0/1
  Runnable_IMAP_10ms_sys/87(IMAPve_d_ESC_AlarmSig) -> IMAPve_d_ESC_AlarmSig/1
  Runnable_IMAP_10ms_sys/185(IMAPve_g_ORI_L0_C0) -> IMAPve_g_ORI_L0_C0/1
  Runnable_IMAP_10ms_sys/115(IMAPve_d_TCU_DCT_Clutch_State) -> IMAPve_d_TCU_DCT_Clutch_State/1
  SDFAve_g_L1_LINE_COFIDENCE/1 -> Runnable_IMAP_10ms_sys/118(SDFAve_g_L1_LINE_COFIDENCE)
  Runnable_IMAP_10ms_sys/23(IMAPve_d_LF_Switch) -> IMAPve_d_LF_Switch/1
  Runnable_IMAP_10ms_sys/184(IMAPve_g_ORI_L0_C1) -> IMAPve_g_ORI_L0_C1/1
  Runnable_IMAP_10ms_sys/236(IMAPva_g_obj_acc_y) -> IMAPva_g_obj_acc_y/1
  Runnable_IMAP_10ms_sys/41(IMAPve_d_ESC_LonAcc_Valid) -> IMAPve_d_ESC_LonAcc_Valid/1
  Runnable_IMAP_10ms_sys/197(IMAPve_d_ORI_L1_Type) -> IMAPve_d_ORI_L1_Type/1
  Runnable_IMAP_10ms_sys/221(IMAPve_d_ORI_R1_LC) -> IMAPve_d_ORI_R1_LC/1
  Runnable_IMAP_10ms_sys/237(IMAPva_g_obj_pos_var_x) -> IMAPva_g_obj_pos_var_x/1
  SDFAva_g_obj_vel_x/1 -> Runnable_IMAP_10ms_sys/70(SDFAva_g_obj_vel_x)
  Runnable_IMAP_10ms_sys/97(IMAPve_d_ESC_FL_WheelPulVal) -> IMAPve_d_ESC_FL_WheelPulVal/1
  Runnable_IMAP_10ms_sys/233(IMAPva_g_obj_vel_x) -> IMAPva_g_obj_vel_x/1
  Runnable_IMAP_10ms_sys/330(IMAPve_g_R1_C2_FR_Pred) -> IMAPve_g_R1_C2_FR_Pred/1
  Runnable_IMAP_10ms_sys/50(IMAPve_d_BCM_Right_Light) -> IMAPve_d_BCM_Right_Light/1
  Runnable_IMAP_10ms_sys/110(IMAPve_d_ESC_FR_Wheel_Pulse) -> IMAPve_d_ESC_FR_Wheel_Pulse/1
  SWINve_g_Mech_Loss_Eng_Torq/1 -> Runnable_IMAP_10ms_sys/217(SWINve_g_Mech_Loss_Eng_Torq)
  CAFDva_y_F_CameraData453/1 -> Runnable_IMAP_10ms_sys/246(CAFDva_y_F_CameraData453)
  SWINve_y_ESP_Status_AEBJerk_Response/1 -> Runnable_IMAP_10ms_sys/221(SWINve_y_ESP_Status_AEBJerk_Response)
  SDFAve_g_R1_FR_PRED_RANGE/1 -> Runnable_IMAP_10ms_sys/168(SDFAve_g_R1_FR_PRED_RANGE)
  SDFAve_g_R0_C3_COEF/1 -> Runnable_IMAP_10ms_sys/103(SDFAve_g_R0_C3_COEF)
  Runnable_IMAP_10ms_sys/162(IMAPve_d_Time_System_Clock) -> IMAPve_d_Time_System_Clock/1
  Runnable_IMAP_10ms_sys/201(IMAPve_d_ORI_L1_LC) -> IMAPve_d_ORI_L1_LC/1
  SWINve_y_ESP_Status_ACC_Available/1 -> Runnable_IMAP_10ms_sys/201(SWINve_y_ESC_ACCAvailable)
  SDFAve_g_R0_C2_FR_PRE_COEF/1 -> Runnable_IMAP_10ms_sys/149(SDFAve_g_R0_C2_FR_PRE_COEF)
  SWINve_g_ax/1 -> Runnable_IMAP_10ms_sys/2(SWINve_g_ACCEL_LONGI_CALIB)
  Runnable_IMAP_10ms_sys/58(IMAPve_d_SCC_Left_SwitchSig) -> IMAPve_d_SCC_Left_SwitchSig/1
  Runnable_IMAP_10ms_sys/195(IMAPve_g_ORI_L1_C0) -> IMAPve_g_ORI_L1_C0/1
  Runnable_IMAP_10ms_sys/211(IMAPve_d_ORI_R0_LC) -> IMAPve_d_ORI_R0_LC/1
  Runnable_IMAP_10ms_sys/164(IMAPve_g_GW_IC_Odometer) -> IMAPve_g_GW_IC_Odometer/1
  SDFAve_g_L1_BACK_RANGE/1 -> Runnable_IMAP_10ms_sys/155(SDFAve_g_L1_BACK_RANGE)
  Runnable_IMAP_10ms_sys/333(IMAPve_d_TSR_Sign_Type) -> IMAPve_d_TSR_Sign_Type/1
  Runnable_IMAP_10ms_sys/187(IMAPve_d_ORI_L0_Type) -> IMAPve_d_ORI_L0_Type/1
  Runnable_IMAP_10ms_sys/301(IMAPve_g_L0_C0_FR_Pred) -> IMAPve_g_L0_C0_FR_Pred/1
  SDFAve_d_sen_sta_LF_radar/1 -> Runnable_IMAP_10ms_sys/60(SDFAve_d_sen_sta_LF_radar)
  SWINve_y_High_Beam_Status/1 -> Runnable_IMAP_10ms_sys/211(SWINve_y_High_Beam_Status)
  CAFDva_y_F_CameraData455/1 -> Runnable_IMAP_10ms_sys/248(CAFDva_y_F_CameraData455)
  SWINve_y_ABS1_RotDir_RR/1 -> Runnable_IMAP_10ms_sys/176(SWINve_y_ESC_RRWDirection)
  SWINve_y_ABS_active/1 -> Runnable_IMAP_10ms_sys/1(SWINve_y_ABS_in_regulation)
  SDFAva_g_obj_pos_var_x/1 -> Runnable_IMAP_10ms_sys/74(SDFAva_g_obj_pos_var_x)
  Runnable_IMAP_10ms_sys/188(IMAPve_g_ORI_L0_VR) -> IMAPve_g_ORI_L0_VR/1
  Runnable_IMAP_10ms_sys/354(IMAPve_d_BCM_RightTurn_Switch) -> IMAPve_d_BCM_RightTurn_Switch/1
  SDFAve_g_L1_MARK_WIDTH/1 -> Runnable_IMAP_10ms_sys/119(SDFAve_g_L1_MARK_WIDTH)
  Runnable_IMAP_10ms_sys/89(IMAPve_d_ESC_ESC_Active) -> IMAPve_d_ESC_ESC_Active/1
  Runnable_IMAP_10ms_sys/128(IMAPve_d_BCM_FrontWiper_State) -> IMAPve_d_BCM_FrontWiper_State/1
  SDFAve_g_R0_C2_BACK_COEF/1 -> Runnable_IMAP_10ms_sys/144(SDFAve_g_R0_C2_BACK_COEF)
  Runnable_IMAP_10ms_sys/183(IMAPve_g_ORI_L0_C2) -> IMAPve_g_ORI_L0_C2/1
  SDFAve_d_sensor_status/1 -> Runnable_IMAP_10ms_sys/59(SDFAve_d_sensor_status)
  Runnable_IMAP_10ms_sys/312(IMAPve_g_R0_C2_FR_Pred) -> IMAPve_g_R0_C2_FR_Pred/1
  Runnable_IMAP_10ms_sys/293(IMAPve_g_R1_W) -> IMAPve_g_R1_W/1
  Runnable_IMAP_10ms_sys/83(IMAPve_d_ACU_Driver_Belt) -> IMAPve_d_ACU_Driver_Belt/1
  Runnable_IMAP_10ms_sys/132(IMAPve_d_ACU_Passenger_Belt) -> IMAPve_d_ACU_Passenger_Belt/1
  Runnable_IMAP_10ms_sys/69(IMAPve_g_EMS_MinTWhl_Offset) -> IMAPve_g_EMS_MinTWhl_Offset/1
  Runnable_IMAP_10ms_sys/16(IMAPve_d_BSD_LCW_Switch) -> IMAPve_d_BSD_LCW_Switch/1
  Runnable_IMAP_10ms_sys/231(IMAPva_g_obj_pos_x) -> IMAPva_g_obj_pos_x/1
  Runnable_IMAP_10ms_sys/247(IMAPva_d_obj_BrakeLight) -> IMAPva_d_obj_BrakeLight/1
  SDFAve_g_L1_FR_PRED_RANGE/1 -> Runnable_IMAP_10ms_sys/159(SDFAve_g_L1_FR_PRED_RANGE)
  Runnable_IMAP_10ms_sys/308(IMAPve_g_R0_C3_Back) -> IMAPve_g_R0_C3_Back/1
  Runnable_IMAP_10ms_sys/376(IMAPve_d_Rear_Fog_Lamp_State) -> IMAPve_d_Rear_Fog_Lamp_State/1
  Runnable_IMAP_10ms_sys/277(IMAPve_g_L1_C3) -> IMAPve_g_L1_C3/1
  Runnable_IMAP_10ms_sys/339(IMAPve_d_ESC_TCS_ErrorStatus) -> IMAPve_d_ESC_TCS_ErrorStatus/1
  SDFAva_g_obj_width/1 -> Runnable_IMAP_10ms_sys/77(SDFAva_g_obj_width)
  SDFAve_g_L0_C2_FR_PRE_COEF/1 -> Runnable_IMAP_10ms_sys/140(SDFAve_g_L0_C2_FR_PRE_COEF)
  SWINve_y_MP5_FCTAActivation/1 -> Runnable_IMAP_10ms_sys/184(SWINve_y_MP5_FCTAActivation)
  Runnable_IMAP_10ms_sys/344(IMAPve_g_EPS_SteeringAngle) -> IMAPve_g_EPS_SteeringAngle/1
  SWINve_y_Mp5_ISA_Mode/1 -> Runnable_IMAP_10ms_sys/179(SWINve_y_Mp5_ISAMode)
  SWINve_y_ESP_Status_AEB_Available/1 -> Runnable_IMAP_10ms_sys/199(SWINve_y_ESC_AEBAvailable)
  SDFAve_g_L0_C1_FR_PRE_COEF/1 -> Runnable_IMAP_10ms_sys/139(SDFAve_g_L0_C1_FR_PRE_COEF)
  Runnable_IMAP_10ms_sys/169(IMAPva_g_ORI_Probability) -> IMAPva_g_ORI_Probability/1
  SWINve_y_wheel_speed_FL_fault/1 -> Runnable_IMAP_10ms_sys/195(SWINve_y_ESC_FLWHeelSpdFaultSignal)
  SDFAve_d_sen_sta_LB_radar/1 -> Runnable_IMAP_10ms_sys/62(SDFAve_d_sen_sta_LB_radar)
  Runnable_IMAP_10ms_sys/105(IMAPve_g_ESC_RL_WhlSpd) -> IMAPve_g_ESC_RL_WhlSpd/1
  Runnable_IMAP_10ms_sys/281(IMAPve_g_L1_Confidence) -> IMAPve_g_L1_Confidence/1
  SDFAve_g_L0_FR_PRED_RANGE/1 -> Runnable_IMAP_10ms_sys/141(SDFAve_g_L0_FR_PRED_RANGE)
  SWINve_y_Rear_Fog_Lamp_Status/1 -> Runnable_IMAP_10ms_sys/213(SWINve_y_Rear_Fog_Lamp_Status)
  Runnable_IMAP_10ms_sys/206(IMAPve_d_ORI_R0_Q) -> IMAPve_d_ORI_R0_Q/1
  Runnable_IMAP_10ms_sys/181(IMAPve_d_ORI_Lane_RoadType) -> IMAPve_d_ORI_Lane_RoadType/1
  Runnable_IMAP_10ms_sys/167(IMAPve_d_ORI_CIPV_ID) -> IMAPve_d_ORI_CIPV_ID/1
  SDFAve_g_R1_BACK_RANGE/1 -> Runnable_IMAP_10ms_sys/164(SDFAve_g_R1_BACK_RANGE)
  SDFAve_d_L1_LINE_TYPE/1 -> Runnable_IMAP_10ms_sys/117(SDFAve_d_L1_LINE_TYPE)
  SWINve_y_kick_down/1 -> Runnable_IMAP_10ms_sys/216(SWINve_y_kick_down)
  Runnable_IMAP_10ms_sys/447(IMAPve_g_ORI_R0_ExistProb) -> IMAPve_g_ORI_R0_ExistProb/1
  Runnable_IMAP_10ms_sys/375(IMAPve_d_Front_Fog_Lamp_State) -> IMAPve_d_Front_Fog_Lamp_State/1
  SDFAve_d_L0_LINE_TYPE/1 -> Runnable_IMAP_10ms_sys/95(SDFAve_d_L0_LINE_TYPE)
  Runnable_IMAP_10ms_sys/389(IMAPve_g_EPS_LKAOverlay_Trq) -> IMAPve_g_EPS_LKAOverlay_Trq/1
  SWINve_y_TCS_active/1 -> Runnable_IMAP_10ms_sys/4(SWINve_y_ASR_in_regulation)
  Runnable_IMAP_10ms_sys/204(IMAPve_g_ORI_R0_C1) -> IMAPve_g_ORI_R0_C1/1
  Runnable_IMAP_10ms_sys/412(IMAPva_g_ORI_Obj_RelVelyStdDev) -> IMAPva_g_ORI_Obj_RelVelyStdDev/1
  SDFAve_g_R0_C3_BACK_COEF/1 -> Runnable_IMAP_10ms_sys/145(SDFAve_g_R0_C3_BACK_COEF)
  Runnable_IMAP_10ms_sys/328(IMAPve_g_R1_C0_FR_Pred) -> IMAPve_g_R1_C0_FR_Pred/1
  Runnable_IMAP_10ms_sys/78(IMAPve_d_ESC_Veh_Standstill) -> IMAPve_d_ESC_Veh_Standstill/1
  SWINve_y_BCM_DrDoorLockSwStatus/1 -> Runnable_IMAP_10ms_sys/188(SWINve_y_BCM_DoorLockSt)
  Runnable_IMAP_10ms_sys/94(IMAPve_d_ESC_ABS_Active) -> IMAPve_d_ESC_ABS_Active/1
  Runnable_IMAP_10ms_sys/383(IMAPve_d_ESC_Prefill_Response) -> IMAPve_d_ESC_Prefill_Response/1
  SWINve_y_ESP_Status_Prefill_Available/1 -> Runnable_IMAP_10ms_sys/225(SWINve_y_ESP_Status_Prefill_Available)
  Runnable_IMAP_10ms_sys/363(IMAPve_d_MP5_DMS_MessageType) -> IMAPve_d_MP5_DMS_MessageType/1
  SDFAve_g_L0_BACK_RANGE/1 -> Runnable_IMAP_10ms_sys/137(SDFAve_g_L0_BACK_RANGE)
  Runnable_IMAP_10ms_sys/6(IMAPve_d_ISA_Switch) -> IMAPve_d_ISA_Switch/1
  Runnable_IMAP_10ms_sys/287(IMAPve_g_R1_C2) -> IMAPve_g_R1_C2/1
  Runnable_IMAP_10ms_sys/47(IMAPve_g_SW_Angle_Speed) -> IMAPve_g_SW_Angle_Speed/1
  SWINve_g_steering_angle_spd/1 -> Runnable_IMAP_10ms_sys/48(SWINve_g_Steering_wheel_rotation_speed)
  Runnable_IMAP_10ms_sys/7(IMAPve_d_TSR_Switch) -> IMAPve_d_TSR_Switch/1
  SDFAve_y_L1_DETECT_QUALITY/1 -> Runnable_IMAP_10ms_sys/116(SDFAve_y_L1_DETECT_QUALITY)
  Runnable_IMAP_10ms_sys/452(IMAPve_d_ORI_L1_ID) -> IMAPve_d_ORI_L1_ID/1
  Runnable_IMAP_10ms_sys/96(IMAPve_d_ESC_ABS_AlarmSig) -> IMAPve_d_ESC_ABS_AlarmSig/1
  Runnable_IMAP_10ms_sys/331(IMAPve_g_R1_Range_FR_Pred) -> IMAPve_g_R1_Range_FR_Pred/1
  SWINve_y_MP5_DOWActivation/1 -> Runnable_IMAP_10ms_sys/186(SWINve_y_MP5_DOWActivation)
  Runnable_IMAP_10ms_sys/9(IMAPve_d_LDW_Warn_Mode) -> IMAPve_d_LDW_Warn_Mode/1
  SDFAva_y_obj_BrakeLight/1 -> Runnable_IMAP_10ms_sys/84(SDFAva_y_obj_BrakeLight)
  Runnable_IMAP_10ms_sys/278(IMAPve_g_L1_VR) -> IMAPve_g_L1_VR/1
  SWINve_y_Engine_Status/1 -> Runnable_IMAP_10ms_sys/12(SWINve_y_EMS_Engine_state)
  SWINve_y_Mp5_LSS_main_SW/1 -> Runnable_IMAP_10ms_sys/30(SWINve_y_LKA_main_switch)
  SWINve_g_wheel_speed_FL/1 -> Runnable_IMAP_10ms_sys/32(SWINve_g_No_filtered_front_left_speed)
  SWINve_y_EPS1_Status_HandsoffValid/1 -> Runnable_IMAP_10ms_sys/228(SWINve_y_EPS1_Status_HandsoffValid)
  SDFAva_g_obj_vel_y/1 -> Runnable_IMAP_10ms_sys/71(SDFAva_g_obj_vel_y)
  Runnable_IMAP_10ms_sys/265(IMAPve_g_R0_C2) -> IMAPve_g_R0_C2/1
  SDFAve_g_R0_C1_FR_PRE_COEF/1 -> Runnable_IMAP_10ms_sys/148(SDFAve_g_R0_C1_FR_PRE_COEF)
  Runnable_IMAP_10ms_sys/200(IMAPve_g_ORI_L1_W) -> IMAPve_g_ORI_L1_W/1
  SDFAve_g_L1_C1_BACK_COEF/1 -> Runnable_IMAP_10ms_sys/152(SDFAve_g_L1_C1_BACK_COEF)
  SWINve_g_minimum_powertrain_torque/1 -> Runnable_IMAP_10ms_sys/14(SWINve_g_EMS_WhlTrq_min)
  Runnable_IMAP_10ms_sys/131(IMAPve_d_GW_Brake_Only_Req) -> IMAPve_d_GW_Brake_Only_Req/1
  Runnable_IMAP_10ms_sys/17(IMAPve_d_FCTA_Switch) -> IMAPve_d_FCTA_Switch/1
  SWINve_y_MP5_ESASwitch/1 -> Runnable_IMAP_10ms_sys/182(SWINve_y_MP5_ESASwitch)
  Runnable_IMAP_10ms_sys/252(IMAPve_g_L0_C0) -> IMAPve_g_L0_C0/1
  Runnable_IMAP_10ms_sys/390(IMAPve_g_EPS_DriverTorque) -> IMAPve_g_EPS_DriverTorque/1
  Runnable_IMAP_10ms_sys/67(IMAPve_g_EMS_MaxTWhl_Offset) -> IMAPve_g_EMS_MaxTWhl_Offset/1
  SWINve_y_brake_pressure/1 -> Runnable_IMAP_10ms_sys/54(SWINve_g_TMC_pressure)
  SWINve_y_Mp5_LDW_Warning_Mode/1 -> Runnable_IMAP_10ms_sys/180(SWINve_y_Mp5_LDWWarningMode)
  SDFAve_g_L0_C0_BACK_COEF/1 -> Runnable_IMAP_10ms_sys/133(SDFAve_g_L0_C0_BACK_COEF)
  Runnable_IMAP_10ms_sys/294(IMAPve_g_R1_TLC) -> IMAPve_g_R1_TLC/1
  Runnable_IMAP_10ms_sys/367(IMAPve_d_MP5_DMS_EyeFatigue) -> IMAPve_d_MP5_DMS_EyeFatigue/1
  SDFAve_g_L1_C0_FR_PRE_COEF/1 -> Runnable_IMAP_10ms_sys/156(SDFAve_g_L1_C0_FR_PRE_COEF)
  SDFAve_g_L0_C1_BACK_COEF/1 -> Runnable_IMAP_10ms_sys/134(SDFAve_g_L0_C1_BACK_COEF)
  Runnable_IMAP_10ms_sys/340(IMAPve_d_ESC_RLW_Direction) -> IMAPve_d_ESC_RLW_Direction/1
  CAFDva_y_F_CameraData450/1 -> Runnable_IMAP_10ms_sys/232(CAFDva_y_F_CameraData450)
  Runnable_IMAP_10ms_sys/267(IMAPve_g_R0_VR) -> IMAPve_g_R0_VR/1
  Runnable_IMAP_10ms_sys/343(IMAPve_d_EPS_SteeringAngle_Flag) -> IMAPve_d_EPS_SteeringAngle_Flag/1
  Runnable_IMAP_10ms_sys/160(IMAPve_d_Radar_State) -> IMAPve_d_Radar_State/1
  Runnable_IMAP_10ms_sys/4(IMAPve_d_FCW_Switch) -> IMAPve_d_FCW_Switch/1
  SDFAva_y_obj_status/1 -> Runnable_IMAP_10ms_sys/81(SDFAva_y_obj_status)
  Runnable_IMAP_10ms_sys/116(IMAPve_d_TCU_Gear_Engage) -> IMAPve_d_TCU_Gear_Engage/1
  Runnable_IMAP_10ms_sys/391(IMAPve_d_EPS_Steer_Hold_State_Valid) -> IMAPve_d_EPS_Steer_Hold_State_Valid/1
  Runnable_IMAP_10ms_sys/336(IMAPve_d_Camera_Status) -> IMAPve_d_Camera_Status/1
  Runnable_IMAP_10ms_sys/73(IMAPve_g_EMS_ACC_VirtualPedal) -> IMAPve_g_EMS_ACC_VirtualPedal/1
  Runnable_IMAP_10ms_sys/302(IMAPve_g_L0_C1_FR_Pred) -> IMAPve_g_L0_C1_FR_Pred/1
  Runnable_IMAP_10ms_sys/254(IMAPve_g_L0_C2) -> IMAPve_g_L0_C2/1
  Runnable_IMAP_10ms_sys/119(IMAPve_d_EMS_Gearbox_CtlAvail) -> IMAPve_d_EMS_Gearbox_CtlAvail/1
  SDFAve_d_sen_sta_RF_radar/1 -> Runnable_IMAP_10ms_sys/61(SDFAve_d_sen_sta_RF_radar)
  Runnable_IMAP_10ms_sys/65(IMAPve_g_EMS_RealPedal) -> IMAPve_g_EMS_RealPedal/1
  SWINve_y_Mp5_LSS_Mode/1 -> Runnable_IMAP_10ms_sys/29(SWINve_y_LC_Mode)
  Runnable_IMAP_10ms_sys/32(IMAPve_d_EPS_TrqLim_State) -> IMAPve_d_EPS_TrqLim_State/1
  Runnable_IMAP_10ms_sys/351(IMAPve_d_EMS_PowertrainCtl_State) -> IMAPve_d_EMS_PowertrainCtl_State/1
  Runnable_IMAP_10ms_sys/21(IMAPve_d_JA_Alert_Switch) -> IMAPve_d_JA_Alert_Switch/1
  Runnable_IMAP_10ms_sys/46(IMAPve_g_SW_Angle) -> IMAPve_g_SW_Angle/1
  Runnable_IMAP_10ms_sys/342(IMAPve_d_ESC_EPB_ErrorStatus) -> IMAPve_d_ESC_EPB_ErrorStatus/1
  SWINve_g_EPS1_IND_LKAOverlayTorque_Value/1 -> Runnable_IMAP_10ms_sys/226(SWINve_g_EPS1_IND_LKAOverlayTorque_Value)
  Runnable_IMAP_10ms_sys/323(IMAPve_g_R1_C0_Back) -> IMAPve_g_R1_C0_Back/1
  SWINve_y_TCU2_Status_TransFailure/1 -> Runnable_IMAP_10ms_sys/52(SWINve_y_TCU_ATFailure)
  Runnable_IMAP_10ms_sys/217(IMAPve_d_ORI_R1_LT) -> IMAPve_d_ORI_R1_LT/1
  SWINve_y_Right_Turn_Lamp_Status/1 -> Runnable_IMAP_10ms_sys/205(SWINve_y_BCM_RightlightSt)
  Runnable_IMAP_10ms_sys/261(IMAPve_g_L0_TLC) -> IMAPve_g_L0_TLC/1
  Runnable_IMAP_10ms_sys/125(IMAPve_d_ESC_ACC_Available) -> IMAPve_d_ESC_ACC_Available/1
  Runnable_IMAP_10ms_sys/370(IMAPve_d_MP5_DMS_UsingPhone) -> IMAPve_d_MP5_DMS_UsingPhone/1
  SDFAve_g_R1_C0_BACK_COEF/1 -> Runnable_IMAP_10ms_sys/160(SDFAve_g_R1_C0_BACK_COEF)
  SWINve_y_ax_fault/1 -> Runnable_IMAP_10ms_sys/193(SWINve_y_ESC_LongitudinalAccelerationValidity)
  Runnable_IMAP_10ms_sys/202(IMAPve_g_ORI_R0_C3) -> IMAPve_g_ORI_R0_C3/1
  SWINve_y_steering_angle_valid/1 -> Runnable_IMAP_10ms_sys/27(SWINve_y_Internal_SWS_status)
  Runnable_IMAP_10ms_sys/371(IMAPve_d_MP5_DMS_Smoking) -> IMAPve_d_MP5_DMS_Smoking/1
  Runnable_IMAP_10ms_sys/318(IMAPve_g_L1_Range_Back) -> IMAPve_g_L1_Range_Back/1
  Runnable_IMAP_10ms_sys/86(IMAPve_d_ESC_OFF) -> IMAPve_d_ESC_OFF/1
  Runnable_IMAP_10ms_sys/225(IMAPve_d_LR_Radar_Status) -> IMAPve_d_LR_Radar_Status/1
  SWINve_y_TargetGear/1 -> Runnable_IMAP_10ms_sys/51(SWINve_y_TCU_AGB_Target_position)
  Runnable_IMAP_10ms_sys/360(IMAPve_d_MP5_UPA_Switch) -> IMAPve_d_MP5_UPA_Switch/1
  Runnable_IMAP_10ms_sys/138(IMAPve_d_EPB_Status) -> IMAPve_d_EPB_Status/1
  Runnable_IMAP_10ms_sys/161(IMAPve_d_ACC_Desired_Headway) -> IMAPve_d_ACC_Desired_Headway/1
  SDFAve_g_R1_VIEW_RANGE/1 -> Runnable_IMAP_10ms_sys/126(SDFAve_g_R1_VIEW_RANGE)
  Runnable_IMAP_10ms_sys/159(IMAPve_d_TPMS_Warn_Indicate) -> IMAPve_d_TPMS_Warn_Indicate/1
  Runnable_IMAP_10ms_sys/36(IMAPve_g_ESC_YawRate) -> IMAPve_g_ESC_YawRate/1
  SDFAve_y_LANE_DETECT_ACTIV/1 -> Runnable_IMAP_10ms_sys/86(SDFAve_y_LANE_DETECT_ACTIV)
  Runnable_IMAP_10ms_sys/240(IMAPva_g_obj_width) -> IMAPva_g_obj_width/1
  Runnable_IMAP_10ms_sys/80(IMAPve_d_TCU_Target_Gear) -> IMAPve_d_TCU_Target_Gear/1
  Runnable_IMAP_10ms_sys/25(IMAPve_d_ALC_Sensitivity) -> IMAPve_d_ALC_Sensitivity/1
  Runnable_IMAP_10ms_sys/112(IMAPve_d_ESC_RR_Wheel_Pulse) -> IMAPve_d_ESC_RR_Wheel_Pulse/1
  SWINve_y_ABS_fault/1 -> Runnable_IMAP_10ms_sys/194(SWINve_y_ESC_ABSValidity)
  SWINve_y_ABS3_WhlPulseCnt_RL/1 -> Runnable_IMAP_10ms_sys/40(SWINve_g_Pulse_counter_rearleft_wheel)
  CAFDva_y_F_CameraData457/1 -> Runnable_IMAP_10ms_sys/250(CAFDva_y_F_CameraData457)
  Runnable_IMAP_10ms_sys/129(IMAPve_d_BCM_CHMSL_Status) -> IMAPve_d_BCM_CHMSL_Status/1
  Runnable_IMAP_10ms_sys/81(IMAPve_d_TCU_PRND_State) -> IMAPve_d_TCU_PRND_State/1
  SWINve_y_Mp5_TSR_Switch/1 -> Runnable_IMAP_10ms_sys/21(SWINve_y_GW_Mp5_TSR_Switch)
  Runnable_IMAP_10ms_sys/307(IMAPve_g_R0_C2_Back) -> IMAPve_g_R0_C2_Back/1
  Runnable_IMAP_10ms_sys/379(IMAPve_d_EMS_Kickdown) -> IMAPve_d_EMS_Kickdown/1
  Runnable_IMAP_10ms_sys/393(IMAPve_d_ORI_FS_OutOfCalib) -> IMAPve_d_ORI_FS_OutOfCalib/1
  Runnable_IMAP_10ms_sys/243(IMAPva_d_obj_lane) -> IMAPva_d_obj_lane/1
  Runnable_IMAP_10ms_sys/22(IMAPve_d_JA_Alert_Sensitivity) -> IMAPve_d_JA_Alert_Sensitivity/1
  Runnable_IMAP_10ms_sys/286(IMAPve_g_R1_C1) -> IMAPve_g_R1_C1/1
  Runnable_IMAP_10ms_sys/144(IMAPve_d_ESC_Hold_State) -> IMAPve_d_ESC_Hold_State/1
  CAFDva_y_F_CameraData45E/1 -> Runnable_IMAP_10ms_sys/238(CAFDva_y_F_CameraData45E)
  Runnable_IMAP_10ms_sys/126(IMAPve_d_ESC_ACC_Active) -> IMAPve_d_ESC_ACC_Active/1
  CAFDva_y_F_CameraData422/1 -> Runnable_IMAP_10ms_sys/242(CAFDva_y_F_CameraData422)
  Runnable_IMAP_10ms_sys/153(IMAPve_d_TBOX_LocalTimeM) -> IMAPve_d_TBOX_LocalTimeM/1
  Runnable_IMAP_10ms_sys/224(IMAPve_d_RF_Radar_Status) -> IMAPve_d_RF_Radar_Status/1
  CAFDva_y_F_CameraData421/1 -> Runnable_IMAP_10ms_sys/241(CAFDva_y_F_CameraData421)
  SWINve_y_MP5_RCTAActivation/1 -> Runnable_IMAP_10ms_sys/185(SWINve_y_MP5_RCTAActivation)
  Runnable_IMAP_10ms_sys/63(IMAPve_g_EMS_Pot_WhlT_Max) -> IMAPve_g_EMS_Pot_WhlT_Max/1
  SDFAve_g_L1_C0_COEF/1 -> Runnable_IMAP_10ms_sys/111(SDFAve_g_L1_C0_COEF)
  Runnable_IMAP_10ms_sys/173(IMAPva_g_ORI_Obj_LongDis) -> IMAPva_g_ORI_Obj_LongDis/1
  SWINve_y_BCM_DriverDoorSt/1 -> Runnable_IMAP_10ms_sys/207(SWINve_y_BCM_LFDoorSwitchSt)
  SWINve_g_vehicle_speed/1 -> Runnable_IMAP_10ms_sys/56(SWINve_g_Vehicle_speed_of_wheelsensor)
  SWINve_y_calibrated_status/1 -> Runnable_IMAP_10ms_sys/49(SWINve_y_SWS_calibration)
  SDFAve_g_L1_TLC/1 -> Runnable_IMAP_10ms_sys/120(SDFAve_g_L1_TLC)
  Runnable_IMAP_10ms_sys/436(IMAPva_d_ORI_Obj_HeadOrientation) -> IMAPva_d_ORI_Obj_HeadOrientation/1
  Runnable_IMAP_10ms_sys/238(IMAPva_g_obj_pos_var_y) -> IMAPva_g_obj_pos_var_y/1
  Runnable_IMAP_10ms_sys/20(IMAPve_d_JA_Brake_Switch) -> IMAPve_d_JA_Brake_Switch/1
  Runnable_IMAP_10ms_sys/270(IMAPve_g_R0_Confidence) -> IMAPve_g_R0_Confidence/1
  Runnable_IMAP_10ms_sys/95(IMAPve_d_ESC_ABS_Valid) -> IMAPve_d_ESC_ABS_Valid/1
  SWINve_g_ay/1 -> Runnable_IMAP_10ms_sys/28(SWINve_g_Lateral_acceleration)
  Runnable_IMAP_10ms_sys/136(IMAPve_d_BCM_LowBeam_State) -> IMAPve_d_BCM_LowBeam_State/1
  Runnable_IMAP_10ms_sys/165(IMAPve_g_FAPA_State) -> IMAPve_g_FAPA_State/1
  SWINve_y_ABS3_RRWhlPulseCnt_Valid/1 -> Runnable_IMAP_10ms_sys/43(SWINve_y_Rear_Right_pulse_malfunction)
  Runnable_IMAP_10ms_sys/100(IMAPve_d_ESC_RR_WheelPulVal) -> IMAPve_d_ESC_RR_WheelPulVal/1
  Runnable_IMAP_10ms_sys/348(IMAPve_d_ACU_RearLeft_Belt) -> IMAPve_d_ACU_RearLeft_Belt/1
  SDFAva_y_obj_lane/1 -> Runnable_IMAP_10ms_sys/80(SDFAva_y_obj_lane)
  Runnable_IMAP_10ms_sys/448(IMAPve_g_ORI_R0_Dxstart) -> IMAPve_g_ORI_R0_Dxstart/1
  Runnable_IMAP_10ms_sys/15(IMAPve_d_PEPS_RKE_Command) -> IMAPve_d_PEPS_RKE_Command/1
  SWINve_y_Mp5_ISA_Switch/1 -> Runnable_IMAP_10ms_sys/20(SWINve_y_GW_Mp5_ISA_Switch)
  SDFAve_g_L1_VIEW_RANGE/1 -> Runnable_IMAP_10ms_sys/115(SDFAve_g_L1_VIEW_RANGE)
  SWINve_y_ActualGear/1 -> Runnable_IMAP_10ms_sys/53(SWINve_y_TCU_Gear_lever_position)
  Runnable_IMAP_10ms_sys/11(IMAPve_d_ALC_TLC_Mode) -> IMAPve_d_ALC_TLC_Mode/1
  SDFAve_g_fusion_time_stamp/1 -> Runnable_IMAP_10ms_sys/65(SDFAve_g_fusion_time_stamp)
  SWINve_y_ABS3_FLWhlPulseCnt_Valid/1 -> Runnable_IMAP_10ms_sys/16(SWINve_y_Front_Left_pulse_malfunction)
  Runnable_IMAP_10ms_sys/306(IMAPve_g_R0_C1_Back) -> IMAPve_g_R0_C1_Back/1
  SDFAve_g_L0_VIEW_RANGE/1 -> Runnable_IMAP_10ms_sys/93(SDFAve_g_L0_VIEW_RANGE)
  SDFAva_g_obj_pos_var_y/1 -> Runnable_IMAP_10ms_sys/75(SDFAva_g_obj_pos_var_y)
  Runnable_IMAP_10ms_sys/385(IMAPve_d_ESC_FCW_DBS_Response) -> IMAPve_d_ESC_FCW_DBS_Response/1
  SDFAve_g_L1_C3_BACK_COEF/1 -> Runnable_IMAP_10ms_sys/154(SDFAve_g_L1_C3_BACK_COEF)
  SWINve_y_ay_fault/1 -> Runnable_IMAP_10ms_sys/191(SWINve_y_ESC_LateralAccelarationValidity)
  Runnable_IMAP_10ms_sys/380(IMAPve_g_EMS_Mech_Loss_Trq) -> IMAPve_g_EMS_Mech_Loss_Trq/1
  SWINve_g_wheel_speed_RL/1 -> Runnable_IMAP_10ms_sys/34(SWINve_g_No_filtered_rear_left_speed)
  Runnable_IMAP_10ms_sys/12(IMAPve_d_ESA_Switch) -> IMAPve_d_ESA_Switch/1
  SDFAve_g_L0_C0_COEF/1 -> Runnable_IMAP_10ms_sys/89(SDFAve_g_L0_C0_COEF)
  Runnable_IMAP_10ms_sys/368(IMAPve_d_MP5_DMS_LongtimeDrive) -> IMAPve_d_MP5_DMS_LongtimeDrive/1
  Runnable_IMAP_10ms_sys/314(IMAPve_g_L1_C0_Back) -> IMAPve_g_L1_C0_Back/1
  Runnable_IMAP_10ms_sys/1(IMAPve_d_LKA_Main_Switch) -> IMAPve_d_LKA_Main_Switch/1
  SDFAve_g_R0_C1_COEF/1 -> Runnable_IMAP_10ms_sys/101(SDFAve_g_R0_C1_COEF)
  Runnable_IMAP_10ms_sys/28(IMAPve_d_EPS_Error_State) -> IMAPve_d_EPS_Error_State/1
  CAFDva_y_F_CameraData45A/1 -> Runnable_IMAP_10ms_sys/234(CAFDva_y_F_CameraData45A)
  SWINve_y_MP5_BSD_LCW_Activation/1 -> Runnable_IMAP_10ms_sys/183(SWINve_y_MP5_BSD_LCW_Activation)
  Runnable_IMAP_10ms_sys/374(IMAPve_d_High_Beam_State) -> IMAPve_d_High_Beam_State/1
  SWINve_y_BCM1_Status_ACCSwt/1 -> Runnable_IMAP_10ms_sys/178(SWINve_y_MP5_AutoPilotSwitch)
  Runnable_IMAP_10ms_sys/319(IMAPve_g_L1_C0_FR_Pred) -> IMAPve_g_L1_C0_FR_Pred/1
  Runnable_IMAP_10ms_sys/449(IMAPve_d_ORI_R0_ColorClass) -> IMAPve_d_ORI_R0_ColorClass/1
  SWINve_y_BCM_LuggageDoorSt/1 -> Runnable_IMAP_10ms_sys/206(SWINve_y_BCM_TrunkSt)
  SDFAve_g_L0_C2_BACK_COEF/1 -> Runnable_IMAP_10ms_sys/135(SDFAve_g_L0_C2_BACK_COEF)
  Runnable_IMAP_10ms_sys/234(IMAPva_g_obj_vel_y) -> IMAPva_g_obj_vel_y/1
  SDFAve_g_R1_TLC/1 -> Runnable_IMAP_10ms_sys/131(SDFAve_g_R1_TLC)
  Runnable_IMAP_10ms_sys/77(IMAPve_g_EMS_Engine_Speed) -> IMAPve_g_EMS_Engine_Speed/1
  Runnable_IMAP_10ms_sys/166(IMAPve_d_Outside_Temp) -> IMAPve_d_Outside_Temp/1
  SDFAve_g_L0_LINE_COFIDENCE/1 -> Runnable_IMAP_10ms_sys/96(SDFAve_g_L0_LINE_COFIDENCE)
  SDFAve_g_R1_C2_FR_PRE_COEF/1 -> Runnable_IMAP_10ms_sys/167(SDFAve_g_R1_C2_FR_PRE_COEF)
  Runnable_IMAP_10ms_sys/305(IMAPve_g_R0_C0_Back) -> IMAPve_g_R0_C0_Back/1
  SWINve_y_ESP_Status_Prefill_Response/1 -> Runnable_IMAP_10ms_sys/220(SWINve_y_ESP_Status_Prefill_Response)
  Runnable_IMAP_10ms_sys/145(IMAPve_d_EPS_Steer_Hold_State) -> IMAPve_d_EPS_Steer_Hold_State/1
  CAFDva_y_F_CameraData47E/1 -> Runnable_IMAP_10ms_sys/253(CAFDva_y_F_CameraData47E)
  SWINve_y_ESP_Status_AEBReq_Response/1 -> Runnable_IMAP_10ms_sys/200(SWINve_y_ESC_AEBActive)
  Runnable_IMAP_10ms_sys/106(IMAPve_d_ESC_RL_WhlSpd_Fault) -> IMAPve_d_ESC_RL_WhlSpd_Fault/1
  Runnable_IMAP_10ms_sys/369(IMAPve_d_MP5_DMS_SideView) -> IMAPve_d_MP5_DMS_SideView/1
  Runnable_IMAP_10ms_sys/424(IMAPva_g_ORI_Obj_HeightStdDev) -> IMAPva_g_ORI_Obj_HeightStdDev/1
  Runnable_IMAP_10ms_sys/358(IMAPve_d_MP5_APA_ModeSelect) -> IMAPve_d_MP5_APA_ModeSelect/1
  SWINve_y_ESP_Status_FCW_DBS_Available/1 -> Runnable_IMAP_10ms_sys/224(SWINve_y_ESP_Status_FCW_DBS_Available)
  Runnable_IMAP_10ms_sys/104(IMAPve_d_ESC_FR_WhlSpd_Fault) -> IMAPve_d_ESC_FR_WhlSpd_Fault/1
  Runnable_IMAP_10ms_sys/284(IMAPve_d_L1_LC) -> IMAPve_d_L1_LC/1
  SDFAve_y_R1_LANE_CHANGE/1 -> Runnable_IMAP_10ms_sys/132(SDFAve_y_R1_LANE_CHANGE)
  SWINve_y_Front_Fog_Lamp_Status/1 -> Runnable_IMAP_10ms_sys/212(SWINve_y_Front_Fog_Lamp_Status)
  Runnable_IMAP_10ms_sys/3(IMAPve_d_AEB_Switch) -> IMAPve_d_AEB_Switch/1
  Runnable_IMAP_10ms_sys/241(IMAPva_g_obj_length) -> IMAPva_g_obj_length/1
  Runnable_IMAP_10ms_sys/255(IMAPve_g_L0_C3) -> IMAPve_g_L0_C3/1
  Runnable_IMAP_10ms_sys/245(IMAPva_d_obj_age) -> IMAPva_d_obj_age/1
  SDFAve_g_R0_C0_FR_PRE_COEF/1 -> Runnable_IMAP_10ms_sys/147(SDFAve_g_R0_C0_FR_PRE_COEF)
  SWINve_y_TCS_Fault/1 -> Runnable_IMAP_10ms_sys/174(SWINve_y_ESC_TCSErrorStatus)
  SDFAve_g_R0_BACK_RANGE/1 -> Runnable_IMAP_10ms_sys/146(SDFAve_g_R0_BACK_RANGE)
  Runnable_IMAP_10ms_sys/382(IMAPve_d_ESC_ACCInfo_Error) -> IMAPve_d_ESC_ACCInfo_Error/1
  SWINve_y_Engine3_Status_ExtFunctionValid/1 -> Runnable_IMAP_10ms_sys/8(SWINve_y_EMS_ACCcontrol_Available)
  Runnable_IMAP_10ms_sys/232(IMAPva_g_obj_pos_y) -> IMAPva_g_obj_pos_y/1
  SDFAve_g_L1_C1_COEF/1 -> Runnable_IMAP_10ms_sys/112(SDFAve_g_L1_C1_COEF)
  Runnable_IMAP_10ms_sys/55(IMAPve_d_BCM_RF_Door_State) -> IMAPve_d_BCM_RF_Door_State/1
  Runnable_IMAP_10ms_sys/285(IMAPve_g_R1_C0) -> IMAPve_g_R1_C0/1
  Runnable_IMAP_10ms_sys/178(IMAPva_d_ORI_Obj_ID) -> IMAPva_d_ORI_Obj_ID/1
  Runnable_IMAP_10ms_sys/295(IMAPve_d_R1_LC) -> IMAPve_d_R1_LC/1
  Runnable_IMAP_10ms_sys/13(IMAPve_d_ELK_Switch) -> IMAPve_d_ELK_Switch/1
  SWINve_y_wheel_speed_RL_fault/1 -> Runnable_IMAP_10ms_sys/197(SWINve_y_ESC_RLWHeelSpdFaultSignal)
  Runnable_IMAP_10ms_sys/320(IMAPve_g_L1_C1_FR_Pred) -> IMAPve_g_L1_C1_FR_Pred/1
  SWINve_y_Engine1_IND_AccelPadel_Override/1 -> Runnable_IMAP_10ms_sys/7(SWINve_y_EMS_ACC_Effecitive_EMS)
  Runnable_IMAP_10ms_sys/51(IMAPve_d_ESC_BrakeLamp_Req) -> IMAPve_d_ESC_BrakeLamp_Req/1
  SWINve_y_ESP_Status_ACCReq_Response/1 -> Runnable_IMAP_10ms_sys/202(SWINve_y_ESC_ACCActive)
  SDFAve_g_R0_TLC/1 -> Runnable_IMAP_10ms_sys/109(SDFAve_g_R0_TLC)
  Runnable_IMAP_10ms_sys/82(IMAPve_d_BCM_Ignition_State) -> IMAPve_d_BCM_Ignition_State/1
  Runnable_IMAP_10ms_sys/338(IMAPve_d_ESC_FRW_Direction) -> IMAPve_d_ESC_FRW_Direction/1
  Runnable_IMAP_10ms_sys/152(IMAPve_d_TBOX_LocalTimeY) -> IMAPve_d_TBOX_LocalTimeY/1
  Runnable_IMAP_10ms_sys/361(IMAPve_d_MP5_FLK_Activation) -> IMAPve_d_MP5_FLK_Activation/1
  Runnable_IMAP_10ms_sys/19(IMAPve_d_DOW_Switch) -> IMAPve_d_DOW_Switch/1
  Runnable_IMAP_10ms_sys/107(IMAPve_g_ESC_RR_WhlSpd) -> IMAPve_g_ESC_RR_WhlSpd/1
  SDFAve_g_R0_FR_PRED_RANGE/1 -> Runnable_IMAP_10ms_sys/150(SDFAve_g_R0_FR_PRED_RANGE)
  SWINve_y_EPS1_LKA_AvailSts/1 -> Runnable_IMAP_10ms_sys/46(SWINve_y_State_of_EPS_for_LKA_function)
  SDFAve_g_R1_C2_BACK_COEF/1 -> Runnable_IMAP_10ms_sys/162(SDFAve_g_R1_C2_BACK_COEF)
  SWINve_y_ESP_Status_AEBJerk_Available/1 -> Runnable_IMAP_10ms_sys/223(SWINve_y_ESP_Status_AEBJerk_Available)
  Runnable_IMAP_10ms_sys/109(IMAPve_d_ESC_FL_Wheel_Pulse) -> IMAPve_d_ESC_FL_Wheel_Pulse/1
  Runnable_IMAP_10ms_sys/45(IMAPve_g_ESC_DySlope) -> IMAPve_g_ESC_DySlope/1
  Runnable_IMAP_10ms_sys/214(IMAPve_g_ORI_R1_C1) -> IMAPve_g_ORI_R1_C1/1
  Runnable_IMAP_10ms_sys/163(IMAPve_d_Signal_Time_Stamp) -> IMAPve_d_Signal_Time_Stamp/1
  Runnable_IMAP_10ms_sys/172(IMAPva_g_ORI_Obj_RelVel) -> IMAPva_g_ORI_Obj_RelVel/1
  Runnable_IMAP_10ms_sys/228(IMAPve_g_Fusion_Time_Stamp) -> IMAPve_g_Fusion_Time_Stamp/1
  SWINve_y_VDC_Fault/1 -> Runnable_IMAP_10ms_sys/44(SWINve_y_Request_to_light_fault_lamp)
  Runnable_IMAP_10ms_sys/235(IMAPva_g_obj_acc_x) -> IMAPva_g_obj_acc_x/1
  Runnable_IMAP_10ms_sys/334(IMAPve_d_Camera_Signal_Fault) -> IMAPve_d_Camera_Signal_Fault/1
  SWINve_y_MP5_TLCModeSelection/1 -> Runnable_IMAP_10ms_sys/181(SWINve_y_MP5_TLCModeSelection)
  Runnable_IMAP_10ms_sys/313(IMAPve_g_R0_Range_FR_Pred) -> IMAPve_g_R0_Range_FR_Pred/1
  SDFAve_g_R1_C1_COEF/1 -> Runnable_IMAP_10ms_sys/123(SDFAve_g_R1_C1_COEF)
  Runnable_IMAP_10ms_sys/239(IMAPva_g_obj_pos_var_xy) -> IMAPva_g_obj_pos_var_xy/1
  SDFAve_y_R0_LANE_CHANGE/1 -> Runnable_IMAP_10ms_sys/110(SDFAve_y_R0_LANE_CHANGE)
  SWINve_y_ESP_Status_ACCInfo_Error/1 -> Runnable_IMAP_10ms_sys/219(SWINve_y_ESP_Status_ACCInfo_Error)
  SWINve_y_Powertrain_Torque_Validity/1 -> Runnable_IMAP_10ms_sys/218(SWINve_y_Powertrain_Torque_Validity)
  Runnable_IMAP_10ms_sys/68(IMAPve_g_EMS_MinTWhl) -> IMAPve_g_EMS_MinTWhl/1
  CAFDva_y_F_CameraData45B/1 -> Runnable_IMAP_10ms_sys/235(CAFDva_y_F_CameraData45B)
  Runnable_IMAP_10ms_sys/190(IMAPve_g_ORI_L0_W) -> IMAPve_g_ORI_L0_W/1
  Runnable_IMAP_10ms_sys/137(IMAPve_d_BCM_HighBeam_State) -> IMAPve_d_BCM_HighBeam_State/1
  SDFAve_d_sen_sta_RB_radar/1 -> Runnable_IMAP_10ms_sys/63(SDFAve_d_sen_sta_RB_radar)
  SWINve_g_wheel_speed_FR/1 -> Runnable_IMAP_10ms_sys/33(SWINve_g_No_filtered_front_right_speed)
  SWINve_g_maximum_powertrain_torque/1 -> Runnable_IMAP_10ms_sys/13(SWINve_g_EMS_WhlTrq_max)
  Runnable_IMAP_10ms_sys/194(IMAPve_g_ORI_L1_C1) -> IMAPve_g_ORI_L1_C1/1
  Runnable_IMAP_10ms_sys/57(IMAPve_d_BCM_LR_Door_State) -> IMAPve_d_BCM_LR_Door_State/1
  SWINve_y_BCM_IgnKeyPOS/1 -> Runnable_IMAP_10ms_sys/18(SWINve_y_GW_BCM_SEV_main_state)
  CAFDva_y_F_CameraData424/1 -> Runnable_IMAP_10ms_sys/230(CAFDva_y_F_CameraData424)
  SWINve_y_ESP_Status_Hold/1 -> Runnable_IMAP_10ms_sys/55(SWINve_y_Vehicle_Hold_Status)
  Runnable_IMAP_10ms_sys/43(IMAPve_g_ESC_Static_Slope) -> IMAPve_g_ESC_Static_Slope/1
  Runnable_IMAP_10ms_sys/38(IMAPve_g_ESC_UnYawRate) -> IMAPve_g_ESC_UnYawRate/1
  Runnable_IMAP_10ms_sys/317(IMAPve_g_L1_C3_Back) -> IMAPve_g_L1_C3_Back/1
  SDFAve_g_L0_C2_COEF/1 -> Runnable_IMAP_10ms_sys/91(SDFAve_g_L0_C2_COEF)
  Runnable_IMAP_10ms_sys/249(IMAPve_d_Lane_Valid) -> IMAPve_d_Lane_Valid/1
  Runnable_IMAP_10ms_sys/79(IMAPve_d_TCU_Actual_Gear) -> IMAPve_d_TCU_Actual_Gear/1
  Runnable_IMAP_10ms_sys/88(IMAPve_d_Speed_Limit_Switch) -> IMAPve_d_Speed_Limit_Switch/1
  CAFDva_y_F_CameraData459/1 -> Runnable_IMAP_10ms_sys/233(CAFDva_y_F_CameraData459)
  SWINve_y_APB_Status/1 -> Runnable_IMAP_10ms_sys/37(SWINve_y_Park_brake_function_status)
  Runnable_IMAP_10ms_sys/155(IMAPve_d_TBOX_LocalTimeH) -> IMAPve_d_TBOX_LocalTimeH/1
  Runnable_IMAP_10ms_sys/198(IMAPve_g_ORI_L1_VR) -> IMAPve_g_ORI_L1_VR/1
  Runnable_IMAP_10ms_sys/31(IMAPve_d_SAS_Trim_State) -> IMAPve_d_SAS_Trim_State/1
  Runnable_IMAP_10ms_sys/372(IMAPve_d_MP5_DMS_DrinkWater) -> IMAPve_d_MP5_DMS_DrinkWater/1
  Runnable_IMAP_10ms_sys/402(IMAPve_d_ORI_FS_FrozenWindshield0) -> IMAPve_d_ORI_FS_FrozenWindshield0/1
  Runnable_IMAP_10ms_sys/316(IMAPve_g_L1_C2_Back) -> IMAPve_g_L1_C2_Back/1
  SDFAve_g_L0_MARK_WIDTH/1 -> Runnable_IMAP_10ms_sys/97(SDFAve_g_L0_MARK_WIDTH)
  Runnable_IMAP_10ms_sys/216(IMAPve_d_ORI_R1_Q) -> IMAPve_d_ORI_R1_Q/1
  Runnable_IMAP_10ms_sys/76(IMAPve_d_ESC_Brake_Effort) -> IMAPve_d_ESC_Brake_Effort/1
  Runnable_IMAP_10ms_sys/291(IMAPve_d_R1_Type) -> IMAPve_d_R1_Type/1
  SDFAva_g_obj_pos_var_xy/1 -> Runnable_IMAP_10ms_sys/76(SDFAva_g_obj_pos_var_xy)
  SDFAve_g_L1_C2_COEF/1 -> Runnable_IMAP_10ms_sys/113(SDFAve_g_L1_C2_COEF)
  Runnable_IMAP_Step/1 -> Runnable_IMAP_10ms_sys/Trigger
  SWINve_y_BCM1_IND_OvertakinglampSwt_OnOff/1 -> Runnable_IMAP_10ms_sys/215(SWINve_y_BCM1_IND_OvertakinglampSwt_OnOff)
  Runnable_IMAP_10ms_sys/296(IMAPve_g_L0_C0_Back) -> IMAPve_g_L0_C0_Back/1
  Runnable_IMAP_10ms_sys/168(IMAPve_d_ORI_Obj_Num) -> IMAPve_d_ORI_Obj_Num/1
  Runnable_IMAP_10ms_sys/335(IMAPve_d_Radar_Status) -> IMAPve_d_Radar_Status/1
  Runnable_IMAP_10ms_sys/101(IMAPve_g_ESC_FL_WhlSpd) -> IMAPve_g_ESC_FL_WhlSpd/1
  SDFAve_y_L0_DETECT_QUALITY/1 -> Runnable_IMAP_10ms_sys/94(SDFAve_y_L0_DETECT_QUALITY)
  SWINve_y_APB_IND_Error/1 -> Runnable_IMAP_10ms_sys/177(SWINve_y_ESC_EPBErrorStatus)
  SDFAve_g_L0_C1_COEF/1 -> Runnable_IMAP_10ms_sys/90(SDFAve_g_L0_C1_COEF)
  Runnable_IMAP_10ms_sys/37(IMAPve_d_ESC_YawRate_Valid) -> IMAPve_d_ESC_YawRate_Valid/1
  Runnable_IMAP_10ms_sys/220(IMAPve_g_ORI_R1_W) -> IMAPve_g_ORI_R1_W/1
  SDFAve_g_R1_C3_COEF/1 -> Runnable_IMAP_10ms_sys/125(SDFAve_g_R1_C3_COEF)
  SDFAve_g_R0_VIEW_RANGE/1 -> Runnable_IMAP_10ms_sys/104(SDFAve_g_R0_VIEW_RANGE)
  Runnable_IMAP_10ms_sys/14(IMAPve_d_APA_Command) -> IMAPve_d_APA_Command/1
  Runnable_IMAP_10ms_sys/476(IMAPve_g_ORI_RoadedgeR0_DxStart) -> IMAPve_g_ORI_RoadedgeR0_DxStart/1
  SDFAve_g_R1_LINE_COFIDENCE/1 -> Runnable_IMAP_10ms_sys/129(SDFAve_g_R1_LINE_COFIDENCE)
  Runnable_IMAP_10ms_sys/18(IMAPve_d_RCTA_Swtich) -> IMAPve_d_RCTA_Swtich/1
  Runnable_IMAP_10ms_sys/103(IMAPve_g_ESC_FR_WhlSpd) -> IMAPve_g_ESC_FR_WhlSpd/1
  Runnable_IMAP_10ms_sys/175(IMAPva_g_ORI_Obj_LAngle) -> IMAPva_g_ORI_Obj_LAngle/1
  SDFAva_g_obj_acc_x/1 -> Runnable_IMAP_10ms_sys/72(SDFAva_g_obj_acc_x)
  Runnable_IMAP_10ms_sys/384(IMAPve_d_ESC_AEBJerk_Response) -> IMAPve_d_ESC_AEBJerk_Response/1
  Runnable_IMAP_10ms_sys/199(IMAPve_g_ORI_L1_TLC) -> IMAPve_g_ORI_L1_TLC/1
  SWINve_y_MP5_AEBSwitch/1 -> Runnable_IMAP_10ms_sys/31(SWINve_y_MP5_AEB_Activation_Config)
  Runnable_IMAP_10ms_sys/268(IMAPve_d_R0_Q) -> IMAPve_d_R0_Q/1
  SWINve_y_Psngr_Seat_Belt_Sts/1 -> Runnable_IMAP_10ms_sys/25(SWINve_y_IC_passengerBeltSwitchSig)
  SWINve_y_trimming_status/1 -> Runnable_IMAP_10ms_sys/50(SWINve_y_SWS_trim)
  Runnable_IMAP_10ms_sys/24(IMAPve_d_ICA_Config) -> IMAPve_d_ICA_Config/1
  SDFAve_g_L1_C3_COEF/1 -> Runnable_IMAP_10ms_sys/114(SDFAve_g_L1_C3_COEF)
  SDFAve_y_SIGN_ISA_Value/1 -> Runnable_IMAP_10ms_sys/169(SDFAve_y_SIGN_ISA_Value)
  SWINve_g_Accelerator_ActPedPos/1 -> Runnable_IMAP_10ms_sys/9(SWINve_g_EMS_Acceleration_pedal_position)
  Runnable_IMAP_10ms_sys/62(IMAPve_d_EMS_ACC_Status) -> IMAPve_d_EMS_ACC_Status/1
  Runnable_IMAP_10ms_sys/2(IMAPve_d_LKA_Mode) -> IMAPve_d_LKA_Mode/1
  Runnable_IMAP_10ms_sys/180(IMAPve_d_ORI_Lane_ConsArea) -> IMAPve_d_ORI_Lane_ConsArea/1
  Runnable_IMAP_10ms_sys/349(IMAPve_d_ACU_RearMiddle_Belt) -> IMAPve_d_ACU_RearMiddle_Belt/1
  Runnable_IMAP_10ms_sys/246(IMAPva_d_obj_TurnLight) -> IMAPva_d_obj_TurnLight/1
  Runnable_IMAP_10ms_sys/42(IMAPve_g_ESC_Brake_Press) -> IMAPve_g_ESC_Brake_Press/1
  Runnable_IMAP_10ms_sys/409(IMAPva_g_ORI_Obj_AbsAxStdDev) -> IMAPva_g_ORI_Obj_AbsAxStdDev/1
  Runnable_IMAP_10ms_sys/98(IMAPve_d_ESC_FR_WheelPulVal) -> IMAPve_d_ESC_FR_WheelPulVal/1
  Runnable_IMAP_10ms_sys/26(IMAPve_d_EPS_LKA_State) -> IMAPve_d_EPS_LKA_State/1
  Runnable_IMAP_10ms_sys/462(IMAPve_d_ORI_R1_MeasureType) -> IMAPve_d_ORI_R1_MeasureType/1
  CAFDva_y_F_CameraData454/1 -> Runnable_IMAP_10ms_sys/247(CAFDva_y_F_CameraData454)
  Runnable_IMAP_10ms_sys/192(IMAPve_g_ORI_L1_C3) -> IMAPve_g_ORI_L1_C3/1
  Runnable_IMAP_10ms_sys/215(IMAPve_g_ORI_R1_C0) -> IMAPve_g_ORI_R1_C0/1
  Runnable_IMAP_10ms_sys/212(IMAPve_g_ORI_R1_C3) -> IMAPve_g_ORI_R1_C3/1
  Runnable_IMAP_10ms_sys/350(IMAPve_d_ACU_RearRight_Belt) -> IMAPve_d_ACU_RearRight_Belt/1
  SWINve_y_ABS3_WhlPulseCnt_FL/1 -> Runnable_IMAP_10ms_sys/38(SWINve_g_Pulse_counter_front_left_wheel)
  Runnable_IMAP_10ms_sys/357(IMAPve_d_MP5_Work_State) -> IMAPve_d_MP5_Work_State/1
  Runnable_IMAP_10ms_sys/227(IMAPve_d_Fusion_Status) -> IMAPve_d_Fusion_Status/1
  Runnable_IMAP_10ms_sys/326(IMAPve_g_R1_C3_Back) -> IMAPve_g_R1_C3_Back/1
  Runnable_IMAP_10ms_sys/170(IMAPva_d_ORI_Obj_Class) -> IMAPva_d_ORI_Obj_Class/1
  SDFAva_d_obj_age/1 -> Runnable_IMAP_10ms_sys/82(SDFAva_d_obj_age)
  Runnable_IMAP_10ms_sys/30(IMAPve_d_SAS_Clb_State) -> IMAPve_d_SAS_Clb_State/1
  SWINve_g_yrs/1 -> Runnable_IMAP_10ms_sys/57(SWINve_g_Yaw_speed)
  Runnable_IMAP_10ms_sys/143(IMAPve_d_ESC_Drive_Direction) -> IMAPve_d_ESC_Drive_Direction/1
  SWINve_y_ABS1_RotDir_FR/1 -> Runnable_IMAP_10ms_sys/173(SWINve_y_ESC_FRWDirection)
  SDFAva_y_obj_class/1 -> Runnable_IMAP_10ms_sys/79(SDFAva_y_obj_class)
  Runnable_IMAP_10ms_sys/387(IMAPve_d_ESC_FCW_DBS_Available) -> IMAPve_d_ESC_FCW_DBS_Available/1
  SDFAve_d_fusion_status/1 -> Runnable_IMAP_10ms_sys/64(SDFAve_d_fusion_status)
  SDFAve_g_R0_C1_BACK_COEF/1 -> Runnable_IMAP_10ms_sys/143(SDFAve_g_R0_C1_BACK_COEF)
  Runnable_IMAP_10ms_sys/280(IMAPve_d_L1_Type) -> IMAPve_d_L1_Type/1
  SWINve_y_BCM1_IND_HighBeamSwt_OnOff/1 -> Runnable_IMAP_10ms_sys/22(SWINve_y_High_beam_state)
  SDFAve_d_R0_LINE_TYPE/1 -> Runnable_IMAP_10ms_sys/106(SDFAve_d_R0_LINE_TYPE)
  SDFAve_d_obj_Num/1 -> Runnable_IMAP_10ms_sys/66(SDFAve_d_obj_Num)
  Runnable_IMAP_10ms_sys/108(IMAPve_d_ESC_RR_WhlSpd_Fault) -> IMAPve_d_ESC_RR_WhlSpd_Fault/1
  SDFAve_g_L0_C0_FR_PRE_COEF/1 -> Runnable_IMAP_10ms_sys/138(SDFAve_g_L0_C0_FR_PRE_COEF)
  SDFAve_y_CameraSignalFault/1 -> Runnable_IMAP_10ms_sys/171(SDFAve_y_CameraSignalFault)
  Runnable_IMAP_10ms_sys/248(IMAPva_d_obj_MotionStatus) -> IMAPva_d_obj_MotionStatus/1
  Runnable_IMAP_10ms_sys/346(IMAPve_d_EPS_Driver_Active_ESA) -> IMAPve_d_EPS_Driver_Active_ESA/1
  Runnable_IMAP_10ms_sys/377(IMAPve_d_BCM_Rain_Intensity) -> IMAPve_d_BCM_Rain_Intensity/1
  Runnable_IMAP_10ms_sys/71(IMAPve_g_EMS_Actual_IndT) -> IMAPve_g_EMS_Actual_IndT/1
  SDFAve_g_L1_C0_BACK_COEF/1 -> Runnable_IMAP_10ms_sys/151(SDFAve_g_L1_C0_BACK_COEF)
  Runnable_IMAP_10ms_sys/332(IMAPve_d_Sign_ISA_Value) -> IMAPve_d_Sign_ISA_Value/1
  Runnable_IMAP_10ms_sys/223(IMAPve_d_LF_Radar_Status) -> IMAPve_d_LF_Radar_Status/1
  Runnable_IMAP_10ms_sys/92(IMAPve_d_ESC_VehSpd_Valid) -> IMAPve_d_ESC_VehSpd_Valid/1
  SWINve_y_ABS1_RotDir_RL/1 -> Runnable_IMAP_10ms_sys/175(SWINve_y_ESC_RLWDirection)
  SWINve_y_VDC_active/1 -> Runnable_IMAP_10ms_sys/15(SWINve_y_ESP_in_regulation)
  Runnable_IMAP_10ms_sys/327(IMAPve_g_R1_Range_Back) -> IMAPve_g_R1_Range_Back/1
  Runnable_IMAP_10ms_sys/275(IMAPve_g_L1_C1) -> IMAPve_g_L1_C1/1
  Runnable_IMAP_10ms_sys/99(IMAPve_d_ESC_RL_WheelPulVal) -> IMAPve_d_ESC_RL_WheelPulVal/1
  Runnable_IMAP_10ms_sys/122(IMAPve_d_ESC_AEB_Available) -> IMAPve_d_ESC_AEB_Available/1
  Runnable_IMAP_10ms_sys/74(IMAPve_d_EMS_AccPedal_Fault) -> IMAPve_d_EMS_AccPedal_Fault/1
  CAFDva_y_F_CameraData600/1 -> Runnable_IMAP_10ms_sys/229(CAFDva_y_F_CameraData600)
  SWINve_y_ABS3_FRWhlPulseCnt_Valid/1 -> Runnable_IMAP_10ms_sys/17(SWINve_y_Front_right_pulse_malfunction)
  Runnable_IMAP_10ms_sys/226(IMAPve_d_RR_Radar_Status) -> IMAPve_d_RR_Radar_Status/1
  Runnable_IMAP_10ms_sys/113(IMAPve_d_TCU_AT_Failure) -> IMAPve_d_TCU_AT_Failure/1
  SWINve_y_wheel_speed_RR_fault/1 -> Runnable_IMAP_10ms_sys/198(SWINve_y_ESC_RRWHeelSpdFaultSignal)
  Runnable_IMAP_10ms_sys/121(IMAPve_d_ESC_AEB_Status) -> IMAPve_d_ESC_AEB_Status/1
  SWINve_y_MP5_JASwitch/1 -> Runnable_IMAP_10ms_sys/187(SWINve_y_MP5_JASwitch)
  Runnable_IMAP_10ms_sys/257(IMAPve_d_L0_Q) -> IMAPve_d_L0_Q/1
  Runnable_IMAP_10ms_sys/40(IMAPve_g_ESC_LonAcc) -> IMAPve_g_ESC_LonAcc/1
  Runnable_IMAP_10ms_sys/258(IMAPve_d_L0_Type) -> IMAPve_d_L0_Type/1
  SDFAva_y_obj_TurnLight/1 -> Runnable_IMAP_10ms_sys/83(SDFAva_y_obj_TurnLight)
  Runnable_IMAP_10ms_sys/44(IMAPve_g_ESC_DySlope_Accuracy) -> IMAPve_g_ESC_DySlope_Accuracy/1
  SDFAva_g_obj_pos_y/1 -> Runnable_IMAP_10ms_sys/69(SDFAva_g_obj_pos_y)
  Runnable_IMAP_10ms_sys/102(IMAPve_d_ESC_FL_WhlSpd_Fault) -> IMAPve_d_ESC_FL_WhlSpd_Fault/1
  Runnable_IMAP_10ms_sys/154(IMAPve_d_TBOX_LocalTimeD) -> IMAPve_d_TBOX_LocalTimeD/1
  Runnable_IMAP_10ms_sys/148(IMAPve_d_ESC_EBD_AlarmSig) -> IMAPve_d_ESC_EBD_AlarmSig/1
  SWINve_y_BCM_RRDoorSt/1 -> Runnable_IMAP_10ms_sys/209(SWINve_y_BCM_RRDoorSwitchSt)
  SDFAva_y_obj_MotionStatus/1 -> Runnable_IMAP_10ms_sys/85(SDFAva_y_obj_MotionStatus)
  Runnable_IMAP_10ms_sys/345(IMAPve_d_EPS_Driver_Override) -> IMAPve_d_EPS_Driver_Override/1
  Runnable_IMAP_10ms_sys/229(IMAPve_d_obj_Num) -> IMAPve_d_obj_Num/1
  SWINve_g_steering_angle/1 -> Runnable_IMAP_10ms_sys/47(SWINve_g_Steering_wheel_angle)
  SDFAve_g_R1_C3_BACK_COEF/1 -> Runnable_IMAP_10ms_sys/163(SDFAve_g_R1_C3_BACK_COEF)
  Runnable_IMAP_10ms_sys/70(IMAPve_g_EMS_Actual_FlwT) -> IMAPve_g_EMS_Actual_FlwT/1
  SWINve_y_ESP_EnableSts/1 -> Runnable_IMAP_10ms_sys/3(SWINve_y_ASR_ESP_disconnected)
  Runnable_IMAP_10ms_sys/329(IMAPve_g_R1_C1_FR_Pred) -> IMAPve_g_R1_C1_FR_Pred/1
  Runnable_IMAP_10ms_sys/59(IMAPve_d_SCC_Right_SwitchSig) -> IMAPve_d_SCC_Right_SwitchSig/1
  Runnable_IMAP_10ms_sys/279(IMAPve_d_L1_Q) -> IMAPve_d_L1_Q/1
  SDFAve_y_L0_LANE_CHANGE/1 -> Runnable_IMAP_10ms_sys/99(SDFAve_y_L0_LANE_CHANGE)
  Runnable_IMAP_10ms_sys/259(IMAPve_g_L0_Confidence) -> IMAPve_g_L0_Confidence/1
  Runnable_IMAP_10ms_sys/10(IMAPve_d_Speed_Limit) -> IMAPve_d_Speed_Limit/1
  SWINve_y_Front_Wiper_Status/1 -> Runnable_IMAP_10ms_sys/5(SWINve_y_BCM_State_Front_Wiper)
  Runnable_IMAP_10ms_sys/262(IMAPve_d_L0_LC) -> IMAPve_d_L0_LC/1
  SDFAva_y_obj_id/1 -> Runnable_IMAP_10ms_sys/67(SDFAva_y_obj_id)
  Runnable_IMAP_10ms_sys/191(IMAPve_d_ORI_L0_LC) -> IMAPve_d_ORI_L0_LC/1
  Runnable_IMAP_10ms_sys/324(IMAPve_g_R1_C1_Back) -> IMAPve_g_R1_C1_Back/1
  CAFDva_y_F_CameraData458/1 -> Runnable_IMAP_10ms_sys/251(CAFDva_y_F_CameraData458)
  Runnable_IMAP_10ms_sys/114(IMAPve_d_TCU_Shift_Valid) -> IMAPve_d_TCU_Shift_Valid/1
  Runnable_IMAP_10ms_sys/124(IMAPve_d_ESC_ACC_Status) -> IMAPve_d_ESC_ACC_Status/1
  Runnable_IMAP_10ms_sys/230(IMAPva_d_obj_id) -> IMAPva_d_obj_id/1
  SWINve_y_MP5_FCWSwitch/1 -> Runnable_IMAP_10ms_sys/23(SWINve_y_IC_Fcw_Activation_Config)
  SWINve_y_Low_Beam_Status/1 -> Runnable_IMAP_10ms_sys/189(SWINve_y_BCM_LowBeamStatus)
  Runnable_IMAP_10ms_sys/139(IMAPve_d_EPB_Display_Req) -> IMAPve_d_EPB_Display_Req/1
  SDFAve_y_R0_DETECT_QUALITY/1 -> Runnable_IMAP_10ms_sys/105(SDFAve_y_R0_DETECT_QUALITY)
  Runnable_IMAP_10ms_sys/174(IMAPva_d_ORI_Obj_Lane) -> IMAPva_d_ORI_Obj_Lane/1
  Runnable_IMAP_10ms_sys/311(IMAPve_g_R0_C1_FR_Pred) -> IMAPve_g_R0_C1_FR_Pred/1
  Runnable_IMAP_10ms_sys/54(IMAPve_d_BCM_LF_Door_State) -> IMAPve_d_BCM_LF_Door_State/1
  Runnable_IMAP_10ms_sys/91(IMAPve_d_ESC_TCS_Active) -> IMAPve_d_ESC_TCS_Active/1
  SDFAve_g_R0_LINE_COFIDENCE/1 -> Runnable_IMAP_10ms_sys/107(SDFAve_g_R0_LINE_COFIDENCE)
  Runnable_IMAP_10ms_sys/84(IMAPve_d_SWS_Fault_Code) -> IMAPve_d_SWS_Fault_Code/1
  SWINve_y_MP5_FCW_Sensitivity/1 -> Runnable_IMAP_10ms_sys/24(SWINve_y_IC_FCW_Sensitivity)
  Runnable_IMAP_10ms_sys/479(IMAPve_g_ORI_RoadedgeR0_C0) -> IMAPve_g_ORI_RoadedgeR0_C0/1
  Runnable_IMAP_10ms_sys/133(IMAPve_d_EMS_ACC_CtlAvail) -> IMAPve_d_EMS_ACC_CtlAvail/1
  CAFDva_y_F_CameraData45C/1 -> Runnable_IMAP_10ms_sys/236(CAFDva_y_F_CameraData45C)
  Runnable_IMAP_10ms_sys/315(IMAPve_g_L1_C1_Back) -> IMAPve_g_L1_C1_Back/1
  Runnable_IMAP_10ms_sys/356(IMAPve_d_BCM_IHBC_Enabled) -> IMAPve_d_BCM_IHBC_Enabled/1
  SWINve_g_odometer_value/1 -> Runnable_IMAP_10ms_sys/36(SWINve_g_number_of_kilometer)
  Runnable_IMAP_10ms_sys/341(IMAPve_d_ESC_RRW_Direction) -> IMAPve_d_ESC_RRW_Direction/1
  Runnable_IMAP_10ms_sys/39(IMAPve_g_ESC_VehSpd) -> IMAPve_g_ESC_VehSpd/1
  SDFAve_g_L1_C2_FR_PRE_COEF/1 -> Runnable_IMAP_10ms_sys/158(SDFAve_g_L1_C2_FR_PRE_COEF)
  SWINve_y_BCM1_Rain_Intensity/1 -> Runnable_IMAP_10ms_sys/214(SWINve_y_BCM1_Rain_Intensity)
  Runnable_IMAP_10ms_sys/130(IMAPve_d_BCM_BrakeLamp_State) -> IMAPve_d_BCM_BrakeLamp_State/1
  Runnable_IMAP_10ms_sys/378(IMAPve_d_BCM_OvertakinglampSwt) -> IMAPve_d_BCM_OvertakinglampSwt/1
  Runnable_IMAP_10ms_sys/150(IMAPve_d_Radar_Detective_Req) -> IMAPve_d_Radar_Detective_Req/1
  Runnable_IMAP_10ms_sys/288(IMAPve_g_R1_C3) -> IMAPve_g_R1_C3/1
  Runnable_IMAP_10ms_sys/298(IMAPve_g_L0_C2_Back) -> IMAPve_g_L0_C2_Back/1
  SDFAve_g_L1_C1_FR_PRE_COEF/1 -> Runnable_IMAP_10ms_sys/157(SDFAve_g_L1_C1_FR_PRE_COEF)
  SWINve_y_ABS3_WhlPulseCnt_FR/1 -> Runnable_IMAP_10ms_sys/39(SWINve_g_Pulse_counter_front_right_wheel)
  Runnable_IMAP_10ms_sys/297(IMAPve_g_L0_C1_Back) -> IMAPve_g_L0_C1_Back/1
  SDFAve_g_L1_C2_BACK_COEF/1 -> Runnable_IMAP_10ms_sys/153(SDFAve_g_L1_C2_BACK_COEF)
  SWINve_y_wheel_speed_FR_fault/1 -> Runnable_IMAP_10ms_sys/196(SWINve_y_ESC_FRWHeelSpdFaultSignal)
  Runnable_IMAP_10ms_sys/303(IMAPve_g_L0_C2_FR_Pred) -> IMAPve_g_L0_C2_FR_Pred/1
  Runnable_IMAP_10ms_sys/33(IMAPve_g_EPS_LKA_Current) -> IMAPve_g_EPS_LKA_Current/1
  Runnable_IMAP_10ms_sys/182(IMAPve_g_ORI_L0_C3) -> IMAPve_g_ORI_L0_C3/1
  Runnable_IMAP_10ms_sys/392(IMAPva_d_ORI_Obj_TimeStamp) -> IMAPva_d_ORI_Obj_TimeStamp/1
  Runnable_IMAP_10ms_sys/399(IMAPve_d_ORI_FS_BlurImage0) -> IMAPve_d_ORI_FS_BlurImage0/1
  Runnable_IMAP_10ms_sys/127(IMAPve_d_EMS_ACC_Effective) -> IMAPve_d_EMS_ACC_Effective/1
  Runnable_IMAP_10ms_sys/420(IMAPva_g_ORI_Obj_ClassProb) -> IMAPva_g_ORI_Obj_ClassProb/1
  Runnable_IMAP_10ms_sys/478(IMAPve_g_ORI_RoadedgeR0_C1) -> IMAPve_g_ORI_RoadedgeR0_C1/1
  Runnable_IMAP_10ms_sys/251(IMAPve_d_ConsArea) -> IMAPve_d_ConsArea/1
  SDFAve_d_R1_LINE_TYPE/1 -> Runnable_IMAP_10ms_sys/128(SDFAve_d_R1_LINE_TYPE)
  Runnable_IMAP_10ms_sys/440(IMAPve_d_ORI_L0_ID) -> IMAPve_d_ORI_L0_ID/1
  Runnable_IMAP_10ms_sys/219(IMAPve_g_ORI_R1_TLC) -> IMAPve_g_ORI_R1_TLC/1
  Runnable_IMAP_10ms_sys/405(IMAPva_g_ORI_Obj_AbsAy) -> IMAPva_g_ORI_Obj_AbsAy/1
  Runnable_IMAP_10ms_sys/337(IMAPve_d_ESC_FLW_Direction) -> IMAPve_d_ESC_FLW_Direction/1
  SWINve_y_ABS3_WhlPulseCnt_RR/1 -> Runnable_IMAP_10ms_sys/41(SWINve_g_Pulse_counter_rearright_wheel)
  Runnable_IMAP_10ms_sys/140(IMAPve_d_EPB_Warn_Req) -> IMAPve_d_EPB_Warn_Req/1
  Runnable_IMAP_10ms_sys/400(IMAPve_d_ORI_FS_PartialBlockage0) -> IMAPve_d_ORI_FS_PartialBlockage0/1
  SDFAva_g_obj_pos_x/1 -> Runnable_IMAP_10ms_sys/68(SDFAva_g_obj_pos_x)
  SWINve_y_Driver_Seat_Belt_Sts/1 -> Runnable_IMAP_10ms_sys/26(SWINve_y_IC_seat_bealt_driver_state)
  Runnable_IMAP_10ms_sys/256(IMAPve_g_L0_VR) -> IMAPve_g_L0_VR/1
  Runnable_IMAP_10ms_sys/410(IMAPva_g_ORI_Obj_AbsAyStdDev) -> IMAPva_g_ORI_Obj_AbsAyStdDev/1
  CAFDva_y_F_CameraData451/1 -> Runnable_IMAP_10ms_sys/243(CAFDva_y_F_CameraData451)
  SWINve_y_BCM_RLDoorSt/1 -> Runnable_IMAP_10ms_sys/210(SWINve_y_BCM_LRDoorSwitchSt)
  SDFAve_y_L1_LANE_CHANGE/1 -> Runnable_IMAP_10ms_sys/121(SDFAve_y_L1_LANE_CHANGE)
  Runnable_IMAP_10ms_sys/146(IMAPve_d_EPS_Warning_State) -> IMAPve_d_EPS_Warning_State/1
  Runnable_IMAP_10ms_sys/141(IMAPve_d_EPB_Switch_State) -> IMAPve_d_EPB_Switch_State/1
  Runnable_IMAP_10ms_sys/473(IMAPve_d_ORI_RoadedgeL0_Type) -> IMAPve_d_ORI_RoadedgeL0_Type/1
  SDFAve_g_R1_C2_COEF/1 -> Runnable_IMAP_10ms_sys/124(SDFAve_g_R1_C2_COEF)
  Runnable_IMAP_10ms_sys/441(IMAPve_g_ORI_L0_ExistProb) -> IMAPve_g_ORI_L0_ExistProb/1
  Runnable_IMAP_10ms_sys/263(IMAPve_g_R0_C0) -> IMAPve_g_R0_C0/1
  Runnable_IMAP_10ms_sys/471(IMAPve_g_ORI_RoadedgeL0_C2) -> IMAPve_g_ORI_RoadedgeL0_C2/1
  Runnable_IMAP_10ms_sys/53(IMAPve_d_BCM_Trunk_State) -> IMAPve_d_BCM_Trunk_State/1
  Runnable_IMAP_10ms_sys/413(IMAPva_g_ORI_Obj_LongDisStdDev) -> IMAPva_g_ORI_Obj_LongDisStdDev/1
  Runnable_IMAP_10ms_sys/482(IMAPve_d_ORI_RoadedgeR0_MeasureType) -> IMAPve_d_ORI_RoadedgeR0_MeasureType/1
  Runnable_IMAP_10ms_sys/322(IMAPve_g_L1_Range_FR_Pred) -> IMAPve_g_L1_Range_FR_Pred/1
  Runnable_IMAP_10ms_sys/321(IMAPve_g_L1_C2_FR_Pred) -> IMAPve_g_L1_C2_FR_Pred/1
  Runnable_IMAP_10ms_sys/411(IMAPva_g_ORI_Obj_RelVelStdDev) -> IMAPva_g_ORI_Obj_RelVelStdDev/1
  Runnable_IMAP_10ms_sys/426(IMAPva_g_ORI_Obj_LAngleStdDev) -> IMAPva_g_ORI_Obj_LAngleStdDev/1
  Runnable_IMAP_10ms_sys/419(IMAPva_g_ORI_Obj_ExistProb) -> IMAPva_g_ORI_Obj_ExistProb/1
  Runnable_IMAP_10ms_sys/434(IMAPva_g_ORI_Obj_Heading) -> IMAPva_g_ORI_Obj_Heading/1
  SWINve_y_EPS1_Status_Handsoff/1 -> Runnable_IMAP_10ms_sys/45(SWINve_y_State_indicating_steer_or_not)
  SDFAve_g_R0_C2_COEF/1 -> Runnable_IMAP_10ms_sys/102(SDFAve_g_R0_C2_COEF)
  Runnable_IMAP_10ms_sys/35(IMAPve_d_ESC_LatAcc_Valid) -> IMAPve_d_ESC_LatAcc_Valid/1
  Runnable_IMAP_10ms_sys/147(IMAPve_g_EPS_PowerCon) -> IMAPve_g_EPS_PowerCon/1
  Runnable_IMAP_10ms_sys/454(IMAPve_g_ORI_L1_Dxstart) -> IMAPve_g_ORI_L1_Dxstart/1
  Runnable_IMAP_10ms_sys/475(IMAPve_g_ORI_RoadedgeR0_ExistProb) -> IMAPve_g_ORI_RoadedgeR0_ExistProb/1
  SWINve_y_ABS3_RLWhlPulseCnt_Valid/1 -> Runnable_IMAP_10ms_sys/42(SWINve_y_Rear_Left_pulse_malfunction)
  Runnable_IMAP_10ms_sys/464(IMAPve_d_ORI_RoadedgeL0_ID) -> IMAPve_d_ORI_RoadedgeL0_ID/1
  Runnable_IMAP_10ms_sys/34(IMAPve_g_ESC_LatAcc) -> IMAPve_g_ESC_LatAcc/1
  SWINve_y_ABS1_RotDir_FL/1 -> Runnable_IMAP_10ms_sys/172(SWINve_y_ESC_FLWDirection)
  Runnable_IMAP_10ms_sys/300(IMAPve_g_L0_Range_Back) -> IMAPve_g_L0_Range_Back/1
  Runnable_IMAP_10ms_sys/408(IMAPva_g_ORI_Obj_LateralDis) -> IMAPva_g_ORI_Obj_LateralDis/1
  Runnable_IMAP_10ms_sys/266(IMAPve_g_R0_C3) -> IMAPve_g_R0_C3/1
  Runnable_IMAP_10ms_sys/466(IMAPve_g_ORI_RoadedgeL0_DxStart) -> IMAPve_g_ORI_RoadedgeL0_DxStart/1
  Runnable_IMAP_10ms_sys/373(IMAPve_d_MP5_DMS_UserAccount) -> IMAPve_d_MP5_DMS_UserAccount/1
  Runnable_IMAP_10ms_sys/366(IMAPve_d_MP5_DMS_Sensity) -> IMAPve_d_MP5_DMS_Sensity/1
  Runnable_IMAP_10ms_sys/422(IMAPva_g_ORI_Obj_LengthStdDev) -> IMAPva_g_ORI_Obj_LengthStdDev/1
  Runnable_IMAP_10ms_sys/444(IMAPve_d_ORI_L0_MeasureType) -> IMAPve_d_ORI_L0_MeasureType/1
  Runnable_IMAP_10ms_sys/453(IMAPve_g_ORI_L1_ExistProb) -> IMAPve_g_ORI_L1_ExistProb/1
  SDFAve_g_R1_C1_FR_PRE_COEF/1 -> Runnable_IMAP_10ms_sys/166(SDFAve_g_R1_C1_FR_PRE_COEF)
  Runnable_IMAP_10ms_sys/135(IMAPve_d_EMS_Brake_Pedal) -> IMAPve_d_EMS_Brake_Pedal/1
  Runnable_IMAP_10ms_sys/179(IMAPve_d_ORI_Lane_Valid) -> IMAPve_d_ORI_Lane_Valid/1
  Runnable_IMAP_10ms_sys/177(IMAPva_g_ORI_Obj_Width) -> IMAPva_g_ORI_Obj_Width/1
  Runnable_IMAP_10ms_sys/401(IMAPve_d_ORI_FS_FullBlockage0) -> IMAPve_d_ORI_FS_FullBlockage0/1
  Runnable_IMAP_10ms_sys/189(IMAPve_g_ORI_L0_TLC) -> IMAPve_g_ORI_L0_TLC/1
  SDFAve_g_R1_C0_FR_PRE_COEF/1 -> Runnable_IMAP_10ms_sys/165(SDFAve_g_R1_C0_FR_PRE_COEF)
  SWINve_g_actual_powertrain_torque/1 -> Runnable_IMAP_10ms_sys/10(SWINve_g_EMS_Actual_torque)
  Runnable_IMAP_10ms_sys/438(IMAPva_d_ORI_Obj_DirectionIndicator) -> IMAPva_d_ORI_Obj_DirectionIndicator/1
  SDFAve_g_R0_C0_BACK_COEF/1 -> Runnable_IMAP_10ms_sys/142(SDFAve_g_R0_C0_BACK_COEF)
  Runnable_IMAP_10ms_sys/446(IMAPve_d_ORI_R0_ID) -> IMAPve_d_ORI_R0_ID/1
  Runnable_IMAP_10ms_sys/61(IMAPve_d_BCM_Door_Lock_State) -> IMAPve_d_BCM_Door_Lock_State/1
  Runnable_IMAP_10ms_sys/203(IMAPve_g_ORI_R0_C2) -> IMAPve_g_ORI_R0_C2/1
  CAFDva_y_F_CameraData420/1 -> Runnable_IMAP_10ms_sys/240(CAFDva_y_F_CameraData420)
  Runnable_IMAP_10ms_sys/470(IMAPve_g_ORI_RoadedgeL0_C3) -> IMAPve_g_ORI_RoadedgeL0_C3/1
  Runnable_IMAP_10ms_sys/457(IMAPve_g_ORI_L1_TypeConf) -> IMAPve_g_ORI_L1_TypeConf/1
  CAFDva_y_F_CameraData423/1 -> Runnable_IMAP_10ms_sys/244(CAFDva_y_F_CameraData423)
  Runnable_IMAP_10ms_sys/381(IMAPve_d_Powertrain_Torque_Valid) -> IMAPve_d_Powertrain_Torque_Valid/1
  Runnable_IMAP_10ms_sys/460(IMAPve_g_ORI_R1_Dxstart) -> IMAPve_g_ORI_R1_Dxstart/1
  SDFAve_g_R1_C0_COEF/1 -> Runnable_IMAP_10ms_sys/122(SDFAve_g_R1_C0_COEF)
  Runnable_IMAP_10ms_sys/352(IMAPve_d_TCU_TCU_Available) -> IMAPve_d_TCU_TCU_Available/1
  Runnable_IMAP_10ms_sys/205(IMAPve_g_ORI_R0_C0) -> IMAPve_g_ORI_R0_C0/1
  Runnable_IMAP_10ms_sys/430(IMAPva_g_ORI_Obj_AngleRateStdDev) -> IMAPva_g_ORI_Obj_AngleRateStdDev/1
  Runnable_IMAP_10ms_sys/5(IMAPve_d_FCW_Sensitivity) -> IMAPve_d_FCW_Sensitivity/1
  Runnable_IMAP_10ms_sys/429(IMAPva_g_ORI_Obj_AngleRate) -> IMAPva_g_ORI_Obj_AngleRate/1
  Runnable_IMAP_10ms_sys/435(IMAPva_g_ORI_Obj_HeadingStdDev) -> IMAPva_g_ORI_Obj_HeadingStdDev/1
  Runnable_IMAP_10ms_sys/207(IMAPve_d_ORI_R0_LT) -> IMAPve_d_ORI_R0_LT/1
  Runnable_IMAP_10ms_sys/222(IMAPve_d_Sensor_Status) -> IMAPve_d_Sensor_Status/1
  SWINve_y_BCM_PassDoorSt/1 -> Runnable_IMAP_10ms_sys/208(SWINve_y_BCM_RFDoorSwitchSt)
  Runnable_IMAP_10ms_sys/282(IMAPve_g_L1_W) -> IMAPve_g_L1_W/1
  SDFAve_g_L0_C3_COEF/1 -> Runnable_IMAP_10ms_sys/92(SDFAve_g_L0_C3_COEF)
  Runnable_IMAP_10ms_sys/396(IMAPve_d_ORI_FS_Splashes0) -> IMAPve_d_ORI_FS_Splashes0/1
  Runnable_IMAP_10ms_sys/439(IMAPva_d_ORI_Obj_BrakeLight) -> IMAPva_d_ORI_Obj_BrakeLight/1
  Runnable_IMAP_10ms_sys/193(IMAPve_g_ORI_L1_C2) -> IMAPve_g_ORI_L1_C2/1
  Runnable_IMAP_10ms_sys/272(IMAPve_g_R0_TLC) -> IMAPve_g_R0_TLC/1
  Runnable_IMAP_10ms_sys/176(IMAPva_g_ORI_Obj_RAngle) -> IMAPva_g_ORI_Obj_RAngle/1
  Runnable_IMAP_10ms_sys/209(IMAPve_g_ORI_R0_TLC) -> IMAPve_g_ORI_R0_TLC/1
  Runnable_IMAP_10ms_sys/397(IMAPve_d_ORI_FS_SunRay0) -> IMAPve_d_ORI_FS_SunRay0/1
  Runnable_IMAP_10ms_sys/421(IMAPva_g_ORI_Obj_Height) -> IMAPva_g_ORI_Obj_Height/1
  SDFAve_y_TSR_Sign_Type/1 -> Runnable_IMAP_10ms_sys/170(SDFAve_y_TSR_Sign_Type)
  Runnable_IMAP_10ms_sys/269(IMAPve_d_R0_Type) -> IMAPve_d_R0_Type/1
  Runnable_IMAP_10ms_sys/442(IMAPve_g_ORI_L0_DxStart) -> IMAPve_g_ORI_L0_DxStart/1
  Runnable_IMAP_10ms_sys/309(IMAPve_g_R0_Range_Back) -> IMAPve_g_R0_Range_Back/1
  Runnable_IMAP_10ms_sys/386(IMAPve_d_ESC_AEBJerk_Available) -> IMAPve_d_ESC_AEBJerk_Available/1
  Runnable_IMAP_10ms_sys/210(IMAPve_g_ORI_R0_W) -> IMAPve_g_ORI_R0_W/1
  Runnable_IMAP_10ms_sys/428(IMAPva_g_ORI_Obj_3DAngleStdDev) -> IMAPva_g_ORI_Obj_3DAngleStdDev/1
  Runnable_IMAP_10ms_sys/48(IMAPve_d_BCM_HazardLamp) -> IMAPve_d_BCM_HazardLamp/1
  Runnable_IMAP_10ms_sys/432(IMAPva_g_ORI_Obj_PhiBottomStdDev) -> IMAPva_g_ORI_Obj_PhiBottomStdDev/1
  Runnable_IMAP_10ms_sys/8(IMAPve_d_ISA_ISLC_Mode) -> IMAPve_d_ISA_ISLC_Mode/1
  Runnable_IMAP_10ms_sys/459(IMAPve_g_ORI_R1_ExistProb) -> IMAPve_g_ORI_R1_ExistProb/1
  Runnable_IMAP_10ms_sys/450(IMAPve_d_ORI_R0_MeasureType) -> IMAPve_d_ORI_R0_MeasureType/1
  SDFAve_y_CONSTRUCTION_AREA/1 -> Runnable_IMAP_10ms_sys/88(SDFAve_y_CONSTRUCTION_AREA)
  Runnable_IMAP_10ms_sys/218(IMAPve_g_ORI_R1_VR) -> IMAPve_g_ORI_R1_VR/1
  Runnable_IMAP_10ms_sys/364(IMAPve_d_MP5_DMS_SystemEnable) -> IMAPve_d_MP5_DMS_SystemEnable/1
  Runnable_IMAP_10ms_sys/250(IMAPve_d_Road_Type) -> IMAPve_d_Road_Type/1
  Runnable_IMAP_10ms_sys/75(IMAPve_g_EMS_Driver_Torque) -> IMAPve_g_EMS_Driver_Torque/1
  Runnable_IMAP_10ms_sys/465(IMAPve_g_ORI_RoadedgeL0_ExistProb) -> IMAPve_g_ORI_RoadedgeL0_ExistProb/1
  Runnable_IMAP_10ms_sys/276(IMAPve_g_L1_C2) -> IMAPve_g_L1_C2/1
  Runnable_IMAP_10ms_sys/151(IMAPve_g_BCM_Battery_Voltage) -> IMAPve_g_BCM_Battery_Voltage/1
  Runnable_IMAP_10ms_sys/260(IMAPve_g_L0_W) -> IMAPve_g_L0_W/1
  Runnable_IMAP_10ms_sys/290(IMAPve_d_R1_Q) -> IMAPve_d_R1_Q/1
  SDFAve_g_R1_C1_BACK_COEF/1 -> Runnable_IMAP_10ms_sys/161(SDFAve_g_R1_C1_BACK_COEF)
  Runnable_IMAP_10ms_sys/427(IMAPva_g_ORI_Obj_RAngleStdDev) -> IMAPva_g_ORI_Obj_RAngleStdDev/1
  CAFDva_y_F_CameraData425/1 -> Runnable_IMAP_10ms_sys/231(CAFDva_y_F_CameraData425)
  SWINve_y_yrs_fault/1 -> Runnable_IMAP_10ms_sys/192(SWINve_y_ESC_YawrateValidity)
  Runnable_IMAP_10ms_sys/304(IMAPve_g_L0_Range_FR_Pred) -> IMAPve_g_L0_Range_FR_Pred/1
  Runnable_IMAP_10ms_sys/467(IMAPve_g_ORI_RoadedgeL0_DxEnd) -> IMAPve_g_ORI_RoadedgeL0_DxEnd/1
  Runnable_IMAP_10ms_sys/365(IMAPve_d_MP5_DMS_DelUserNum) -> IMAPve_d_MP5_DMS_DelUserNum/1
  Runnable_IMAP_10ms_sys/362(IMAPve_d_MP5_AutoPilot_Switch) -> IMAPve_d_MP5_AutoPilot_Switch/1
  SDFAve_g_R0_C0_COEF/1 -> Runnable_IMAP_10ms_sys/100(SDFAve_g_R0_C0_COEF)
  Runnable_IMAP_10ms_sys/93(IMAPve_d_Brake_Pedal_Fault) -> IMAPve_d_Brake_Pedal_Fault/1
  Runnable_IMAP_10ms_sys/477(IMAPve_g_ORI_RoadedgeR0_DxEnd) -> IMAPve_g_ORI_RoadedgeR0_DxEnd/1
